simulink model "DYN_6DOF"  (R2018b)
settings: Solver=ode3  StartTime=0.0  StopTime=50  FixedStep=0.01  RelTol=1e-3
(part 2 of 18)

== matlab function DYN_6DOF/Dynamics ==
  data: the input; M output; C output; G output; thed input; m input; I input; len input; x input; y input; z input
function [M,C,G] = fcn(the, thed, m, I, len,x,y,z)
the1 = the(1); the2 = the(2); the3 = the(3);
the4 = the(4); the5 = the(5); the6 = the(6);
the1_dot = thed(1); the2_dot = thed(2); the3_dot = thed(3);
the4_dot = thed(4); the5_dot = thed(5); the6_dot = thed(6);

a1 = len(1);
a2 = len(2); a3 = len(3);
d4 = len(4); 
d7 = len(5)+len(6); d1 = len(7); 
g = 9.81;
m1 = m(1); 
m2 = m(2); 
m3 = m(3); 
m4 = m(4); 
m5 = m(5); 
m6 = m(6);

x1 = x(1); y1 = y(1); z1 = z(1);
x2 = x(2); y2 = y(2); z2 = z(2);
x3 = x(3); y3 = y(3); z3 = z(3);
x4 = x(4); y4 = y(4); z4 = z(4);
x5 = x(5); y5 = y(5); z5 = z(5);
x6 = x(6); y6 = y(6); z6 = z(6);

Ixx1 = I(1,1); Ixx2 = I(2,1); Ixx3 = I(3,1); Ixx4 = I(4,1); Ixx5 = I(5,1); Ixx6 = I(6,1);
Iyy1 = I(1,2); Iyy2 = I(2,2); Iyy3 = I(3,2); Iyy4 = I(4,2); Iyy5 = I(5,2); Iyy6 = I(6,2);
Izz1 = I(1,3); Izz2 = I(2,3); Izz3 = I(3,3); Izz4 = I(4,3); Izz5 = I(5,3); Izz6 = I(6,3);
IPx1 = I(1,4); IPx2 = I(2,4); IPx3 = I(3,4); IPx4 = I(4,4); IPx5 = I(5,4); IPx6 = I(6,4);
IPy1 = I(1,5); IPy2 = I(2,5); IPy3 = I(3,5); IPy4 = I(4,5); IPy5 = I(5,5); IPy6 = I(6,5);
IPz1 = I(1,6); IPz2 = I(2,6); IPz3 = I(3,6); IPz4 = I(4,6); IPz5 = I(5,6); IPz6 = I(6,6);

M = ...
[Ixx2 + Ixx5 + Iyy3 + Iyy6 + Izz1 + Izz4 + a1^2*m2 + a1^2*m3 + a1^2*m4 + a1^2*m5 + a1^2*m6 + a3^2*m4 + a3^2*m5 + a3^2*m6 + m1*x1^2 + m3*x3^2 + m4*x4^2 + m6*x6^2 + m1*y1^2 + m2*y2^2 + m4*y4^2 + m5*y5^2 + m2*z2^2 + m3*z3^2 + m5*z5^2 + m6*z6^2 - Ixx2*cos(the2)^2 + Ixx3*cos(the2)^2 + Ixx3*cos(the3)^2 - Ixx5*cos(the2)^2 - Ixx5*cos(the3)^2 + Ixx6*cos(the2)^2 + Ixx6*cos(the3)^2 - Ixx5*cos(the5)^2 + Ixx6*cos(the6)^2 + Iyy2*cos(the2)^2 - Iyy3*cos(the2)^2 - Iyy3*cos(the3)^2 + Iyy4*cos(the2)^2 + Iyy4*cos(the3)^2 - Iyy6*cos(the2)^2 - Iyy6*cos(the3)^2 + Iyy5*cos(the5)^2 - Iyy6*cos(the5)^2 - Iyy6*cos(the6)^2 - Izz4*cos(the2)^2 - Izz4*cos(the3)^2 + Izz5*cos(the2)^2 + Izz5*cos(the3)^2 + Izz6*cos(the5)^2 - IPx2*sin(2*the2) + IPx3*sin(2*the2) + IPx3*sin(2*the3) - IPx5*sin(2*the5) + IPx6*sin(2*the6) - 2*Ixx3*cos(the2)^2*cos(the3)^2 + Ixx4*cos(the2)^2*cos(the4)^2 + 2*Ixx5*cos(the2)^2*cos(the3)^2 + Ixx4*cos(the3)^2*cos(the4)^2 - 2*Ixx6*cos(the2)^2*cos(the3)^2 + Ixx5*cos(the2)^2*cos(the5)^2 - Ixx6*cos(the2)^2*cos(the4)^2 + Ixx5*cos(the3)^2*cos(the5)^2 - Ixx6*cos(the3)^2*cos(the4)^2 - 2*Ixx6*cos(the2)^2*cos(the6)^2 - 2*Ixx6*cos(the3)^2*cos(the6)^2 - Ixx6*cos(the5)^2*cos(the6)^2 + 2*Iyy3*cos(the2)^2*cos(the3)^2 - 2*Iyy4*cos(the2)^2*cos(the3)^2 - Iyy4*cos(the2)^2*cos(the4)^2 - Iyy4*cos(the3)^2*cos(the4)^2 + Iyy5*cos(the2)^2*cos(the4)^2 + 2*Iyy6*cos(the2)^2*cos(the3)^2 - Iyy5*cos(the2)^2*cos(the5)^2 + Iyy5*cos(the3)^2*cos(the4)^2 - Iyy5*cos(the3)^2*cos(the5)^2 + Iyy6*cos(the2)^2*cos(the5)^2 + 2*Iyy6*cos(the2)^2*cos(the6)^2 + Iyy6*cos(the3)^2*cos(the5)^2 + 2*Iyy6*cos(the3)^2*cos(the6)^2 + Iyy6*cos(the5)^2*cos(the6)^2 + 2*Izz4*cos(the2)^2*cos(the3)^2 - 2*Izz5*cos(the2)^2*cos(the3)^2 - Izz5*cos(the2)^2*cos(the4)^2 - Izz5*cos(the3)^2*cos(the4)^2 + Izz6*cos(the2)^2*cos(the4)^2 - Izz6*cos(the2)^2*cos(the5)^2 + Izz6*cos(the3)^2*cos(the4)^2 - Izz6*cos(the3)^2*cos(the5)^2 + a2^2*m3*cos(the2)^2 + a2^2*m4*cos(the2)^2 + a2^2*m5*cos(the2)^2 - a3^2*m4*cos(the2)^2 + a2^2*m6*cos(the2)^2 - a3^2*m4*cos(the3)^2 - a3^2*m5*cos(the2)^2 - a3^2*m5*cos(the3)^2 - a3^2*m6*cos(the2)^2 - a3^2*m6*cos(the3)^2 + d4^2*m4*cos(the2)^2 + d4^2*m4*cos(the3)^2 + d4^2*m5*cos(the2)^2 + d4^2*m5*cos(the3)^2 + d4^2*m6*cos(the2)^2 + d4^2*m6*cos(the3)^2 + m2*x2^2*cos(the2)^2 - m3*x3^2*cos(the2)^2 - m3*x3^2*cos(the3)^2 + m5*x5^2*cos(the2)^2 + m5*x5^2*cos(the3)^2 - m6*x6^2*cos(the2)^2 + m5*x5^2*cos(the5)^2 - m6*x6^2*cos(the3)^2 - m6*x6^2*cos(the6)^2 - m2*y2^2*cos(the2)^2 + m3*y3^2*cos(the2)^2 + m3*y3^2*cos(the3)^2 - m4*y4^2*cos(the2)^2 - m4*y4^2*cos(the3)^2 + m6*y6^2*cos(the2)^2 - m5*y5^2*cos(the5)^2 + m6*y6^2*cos(the3)^2 + m6*y6^2*cos(the5)^2 + m6*y6^2*cos(the6)^2 + m4*z4^2*cos(the2)^2 + m4*z4^2*cos(the3)^2 - m5*z5^2*cos(the2)^2 - m5*z5^2*cos(the3)^2 - m6*z6^2*cos(the5)^2 - m2*x2*y2*sin(2*the2) + m3*x3*y3*sin(2*the2) + m3*x3*y3*sin(2*the3) - m5*x5*y5*sin(2*the5) + m6*x6*y6*sin(2*the6) + 2*m3*x3^2*cos(the2)^2*cos(the3)^2 - m4*x4^2*cos(the2)^2*cos(the4)^2 - m4*x4^2*cos(the3)^2*cos(the4)^2 - 2*m5*x5^2*cos(the2)^2*cos(the3)^2 - m5*x5^2*cos(the2)^2*cos(the5)^2 + 2*m6*x6^2*cos(the2)^2*cos(the3)^2 - m5*x5^2*cos(the3)^2*cos(the5)^2 + m6*x6^2*cos(the2)^2*cos(the4)^2 + m6*x6^2*cos(the3)^2*cos(the4)^2 + 2*m6*x6^2*cos(the2)^2*cos(the6)^2 + 2*m6*x6^2*cos(the3)^2*cos(the6)^2 + m6*x6^2*cos(the5)^2*cos(the6)^2 - 2*m3*y3^2*cos(the2)^2*cos(the3)^2 + 2*m4*y4^2*cos(the2)^2*cos(the3)^2 + m4*y4^2*cos(the2)^2*cos(the4)^2 + m4*y4^2*cos(the3)^2*cos(the4)^2 - m5*y5^2*cos(the2)^2*cos(the4)^2 + m5*y5^2*cos(the2)^2*cos(the5)^2 - m5*y5^2*cos(the3)^2*cos(the4)^2 - 2*m6*y6^2*cos(the2)^2*cos(the3)^2 + m5*y5^2*cos(the3)^2*cos(the5)^2 - m6*y6^2*cos(the2)^2*cos(the5)^2 - 2*m6*y6^2*cos(the2)^2*cos(the6)^2 - m6*y6^2*cos(the3)^2*cos(the5)^2 - 2*m6*y6^2*cos(the3)^2*cos(the6)^2 - m6*y6^2*cos(the5)^2*cos(the6)^2 - 2*m4*z4^2*cos(the2)^2*cos(the3)^2 + 2*m5*z5^2*cos(the2)^2*cos(the3)^2 + m5*z5^2*cos(the2)^2*cos(the4)^2 + m5*z5^2*cos(the3)^2*cos(the4)^2 - m6*z6^2*cos(the2)^2*cos(the4)^2 + m6*z6^2*cos(the2)^2*cos(the5)^2 - m6*z6^2*cos(the3)^2*cos(the4)^2 + m6*z6^2*cos(the3)^2*cos(the5)^2 - 2*IPx5*cos(the2)*cos(the4)*sin(the2) - 2*IPx5*cos(the3)*cos(the4)*sin(the3) + 2*IPz4*cos(the2)*cos(the4)*sin(the2) + 2*IPz4*cos(the3)*cos(the4)*sin(the3) - 2*IPz6*cos(the5)*cos(the6)*sin(the5) - 2*Ixx4*cos(the2)^2*cos(the3)^2*cos(the4)^2 - 2*Ixx5*cos(the2)^2*cos(the3)^2*cos(the5)^2 + 2*Ixx6*cos(the2)^2*cos(the3)^2*cos(the4)^2 + Ixx5*cos(the2)^2*cos(the4)^2*cos(the5)^2 + Ixx5*cos(the3)^2*cos(the4)^2*cos(the5)^2 + 4*Ixx6*cos(the2)^2*cos(the3)^2*cos(the6)^2 + Ixx6*cos(the2)^2*cos(the4)^2*cos(the6)^2 + Ixx6*cos(the2)^2*cos(the5)^2*cos(the6)^2 + Ixx6*cos(the3)^2*cos(the4)^2*cos(the6)^2 + Ixx6*cos(the3)^2*cos(the5)^2*cos(the6)^2 + 2*Iyy4*cos(the2)^2*cos(the3)^2*cos(the4)^2 - 2*Iyy5*cos(the2)^2*cos(the3)^2*cos(the4)^2 + 2*Iyy5*cos(the2)^2*cos(the3)^2*cos(the5)^2 - Iyy5*cos(the2)^2*cos(the4)^2*cos(the5)^2 - 2*Iyy6*cos(the2)^2*cos(the3)^2*cos(the5)^2 - Iyy5*cos(the3)^2*cos(the4)^2*cos(the5)^2 - 4*Iyy6*cos(the2)^2*cos(the3)^2*cos(the6)^2 + Iyy6*cos(the2)^2*cos(the4)^2*cos(the5)^2 - Iyy6*cos(the2)^2*cos(the4)^2*cos(the6)^2 + Iyy6*cos(the3)^2*cos(the4)^2*cos(the5)^2 - Iyy6*cos(the2)^2*cos(the5)^2*cos(the6)^2 - Iyy6*cos(the3)^2*cos(the4)^2*cos(the6)^2 - Iyy6*cos(the3)^2*cos(the5)^2*cos(the6)^2 + 2*Izz5*cos(the2)^2*cos(the3)^2*cos(the4)^2 - 2*Izz6*cos(the2)^2*cos(the3)^2*cos(the4)^2 + 2*Izz6*cos(the2)^2*cos(the3)^2*cos(the5)^2 - Izz6*cos(the2)^2*cos(the4)^2*cos(the5)^2 - Izz6*cos(the3)^2*cos(the4)^2*cos(the5)^2 - 2*IPy4*cos(the2)*sin(the2)*sin(the4) - 2*IPy4*cos(the3)*sin(the3)*sin(the4) + 2*IPy6*cos(the5)*sin(the5)*sin(the6) + 2*a1*a2*m3*cos(the2) + 2*a1*a2*m4*cos(the2) + 2*a1*a2*m5*cos(the2) + 2*a1*a2*m6*cos(the2) + 2*a1*m2*x2*cos(the2) + 2*a3*m4*x4*cos(the4) - 2*a1*m2*y2*sin(the2) - 2*a3*m4*y4*sin(the4) + 2*a3*m5*z5*sin(the4) - 4*IPx3*cos(the2)*cos(the3)^2*sin(the2) - 4*IPx3*cos(the2)^2*cos(the3)*sin(the3) + 2*IPx4*cos(the2)^2*cos(the4)*sin(the4) + 2*IPx4*cos(the3)^2*cos(the4)*sin(the4) + 2*IPx5*cos(the2)^2*cos(the5)*sin(the5) + 2*IPx5*cos(the3)^2*cos(the5)*sin(the5) - 4*IPx6*cos(the2)^2*cos(the6)*sin(the6) - 4*IPx6*cos(the3)^2*cos(the6)*sin(the6) - 2*IPx6*cos(the5)^2*cos(the6)*sin(the6) + a3*d4*m4*sin(2*the2) + a3*d4*m4*sin(2*the3) + a3*d4*m5*sin(2*the2) + a3*d4*m5*sin(2*the3) + a3*d4*m6*sin(2*the2) + a3*d4*m6*sin(2*the3) + 2*d4*m4*z4*cos(the2)^2 + 2*d4*m4*z4*cos(the3)^2 + a3*m4*z4*sin(2*the2) + a3*m4*z4*sin(2*the3) + 2*a3^2*m4*cos(the2)^2*cos(the3)^2 + 2*a3^2*m5*cos(the2)^2*cos(the3)^2 + 2*a3^2*m6*cos(the2)^2*cos(the3)^2 - 2*d4^2*m4*cos(the2)^2*cos(the3)^2 - 2*d4^2*m5*cos(the2)^2*cos(the3)^2 - 2*d4^2*m6*cos(the2)^2*cos(the3)^2 - 2*IPz6*cos(the2)*cos(the4)*cos(the6)*sin(the2) - 2*IPz6*cos(the3)*cos(the4)*cos(the6)*sin(the3) - 4*d4*m4*z4*cos(the2)^2*cos(the3)^2 + 2*IPy5*cos(the2)*cos(the5)*sin(the2)*sin(the4) + 2*IPy5*cos(the3)*cos(the5)*sin(the3)*sin(the4) + 2*IPy6*cos(the2)*cos(the4)*sin(the2)*sin(the6) + 2*IPy6*cos(the3)*cos(the4)*sin(the3)*sin(the6) + 2*Ixx3*cos(the2)*cos(the3)*sin(the2)*sin(the3) - 2*Ixx5*cos(the2)*cos(the3)*sin(the2)*sin(the3) + 2*Ixx6*cos(the2)*cos(the3)*sin(the2)*sin(the3) - 2*Iyy3*cos(the2)*cos(the3)*sin(the2)*sin(the3) + 2*Iyy4*cos(the2)*cos(the3)*sin(the2)*sin(the3) - 2*Iyy6*cos(the2)*cos(the3)*sin(the2)*sin(the3) - 2*Izz4*cos(the2)*cos(the3)*sin(the2)*sin(the3) + 2*Izz5*cos(the2)*cos(the3)*sin(the2)*sin(the3) + 2*IPx6*cos(the2)*sin(the2)*sin(the4)*sin(the5) + 2*IPx6*cos(the3)*sin(the3)*sin(the4)*sin(the5) + 2*IPz5*cos(the2)*sin(the2)*sin(the4)*sin(the5) + 2*IPz5*cos(the3)*sin(the3)*sin(the4)*sin(the5) + 2*a1*a3*m4*cos(the2)*cos(the3) + 2*a1*a3*m5*cos(the2)*cos(the3) + 2*a1*a3*m6*cos(the2)*cos(the3) + 2*m4*x4^2*cos(the2)^2*cos(the3)^2*cos(the4)^2 + 2*m5*x5^2*cos(the2)^2*cos(the3)^2*cos(the5)^2 - m5*x5^2*cos(the2)^2*cos(the4)^2*cos(the5)^2 - 2*m6*x6^2*cos(the2)^2*cos(the3)^2*cos(the4)^2 - m5*x5^2*cos(the3)^2*cos(the4)^2*cos(the5)^2 - 4*m6*x6^2*cos(the2)^2*cos(the3)^2*cos(the6)^2 - m6*x6^2*cos(the2)^2*cos(the4)^2*cos(the6)^2 - m6*x6^2*cos(the2)^2*cos(the5)^2*cos(the6)^2 - m6*x6^2*cos(the3)^2*cos(the4)^2*cos(the6)^2 - m6*x6^2*cos(the3)^2*cos(the5)^2*cos(the6)^2 - 2*m4*y4^2*cos(the2)^2*cos(the3)^2*cos(the4)^2 + 2*m5*y5^2*cos(the2)^2*cos(the3)^2*cos(the4)^2 - 2*m5*y5^2*cos(the2)^2*cos(the3)^2*cos(the5)^2 + m5*y5^2*cos(the2)^2*cos(the4)^2*cos(the5)^2 + m5*y5^2*cos(the3)^2*cos(the4)^2*cos(the5)^2 + 2*m6*y6^2*cos(the2)^2*cos(the3)^2*cos(the5)^2 + 4*m6*y6^2*cos(the2)^2*cos(the3)^2*cos(the6)^2 - m6*y6^2*cos(the2)^2*cos(the4)^2*cos(the5)^2 + m6*y6^2*cos(the2)^2*cos(the4)^2*cos(the6)^2 - m6*y6^2*cos(the3)^2*cos(the4)^2*cos(the5)^2 + m6*y6^2*cos(the2)^2*cos(the5)^2*cos(the6)^2 + m6*y6^2*cos(the3)^2*cos(the4)^2*cos(the6)^2 + m6*y6^2*cos(the3)^2*cos(the5)^2*cos(the6)^2 - 2*m5*z5^2*cos(the2)^2*cos(the3)^2*cos(the4)^2 + 2*m6*z6^2*cos(the2)^2*cos(the3)^2*cos(the4)^2 - 2*m6*z6^2*cos(the2)^2*cos(the3)^2*cos(the5)^2 + m6*z6^2*cos(the2)^2*cos(the4)^2*cos(the5)^2 + m6*z6^2*cos(the3)^2*cos(the4)^2*cos(the5)^2 - 2*a1*d4*m4*cos(the2)*sin(the3) - 2*a1*d4*m4*cos(the3)*sin(the2) - 2*a1*d4*m5*cos(the2)*sin(the3) - 2*a1*d4*m5*cos(the3)*sin(the2) - 2*a1*d4*m6*cos(the2)*sin(the3) - 2*a1*d4*m6*cos(the3)*sin(the2) + 2*a1*m3*x3*cos(the2)*cos(the3) + 2*a3*m5*x5*cos(the4)*cos(the5) - 2*a1*a3*m4*sin(the2)*sin(the3) - 2*a1*a3*m5*sin(the2)*sin(the3) - 2*a1*a3*m6*sin(the2)*sin(the3) - 2*a1*m3*y3*cos(the2)*sin(the3) - 2*a1*m3*y3*cos(the3)*sin(the2) - 2*a3*m5*y5*cos(the4)*sin(the5) - 2*a3*m6*y6*cos(the6)*sin(the4) - 2*a1*m4*z4*cos(the2)*sin(the3) - 2*a1*m4*z4*cos(the3)*sin(the2) - 2*a3*m6*z6*cos(the4)*sin(the5) - 2*a1*m3*x3*sin(the2)*sin(the3) - 2*a3*m6*x6*sin(the4)*sin(the6) + 4*IPx5*cos(the2)*cos(the3)^2*cos(the4)*sin(the2) + 4*IPx5*cos(the2)^2*cos(the3)*cos(the4)*sin(the3) + 4*IPx5*cos(the2)*cos(the4)*cos(the5)^2*sin(the2) + 4*IPx5*cos(the3)*cos(the4)*cos(the5)^2*sin(the3) - 2*IPx6*cos(the2)^2*cos(the4)*cos(the5)*sin(the4) - 2*IPx6*cos(the3)^2*cos(the4)*cos(the5)*sin(the4) - 4*IPz4*cos(the2)*cos(the3)^2*cos(the4)*sin(the2) - 4*IPz4*cos(the2)^2*cos(the3)*cos(the4)*sin(the3) - 2*IPz5*cos(the2)^2*cos(the4)*cos(the5)*sin(the4) - 2*IPz5*cos(the3)^2*cos(the4)*cos(the5)*sin(the4) + 2*IPz6*cos(the2)^2*cos(the5)*cos(the6)*sin(the5) + 2*IPz6*cos(the3)^2*cos(the5)*cos(the6)*sin(the5) - 2*Ixx5*cos(the2)^2*cos(the3)^2*cos(the4)^2*cos(the5)^2 - 2*Ixx6*cos(the2)^2*cos(the3)^2*cos(the4)^2*cos(the6)^2 - 2*Ixx6*cos(the2)^2*cos(the3)^2*cos(the5)^2*cos(the6)^2 + Ixx6*cos(the2)^2*cos(the4)^2*cos(the5)^2*cos(the6)^2 + Ixx6*cos(the3)^2*cos(the4)^2*cos(the5)^2*cos(the6)^2 + 2*Iyy5*cos(the2)^2*cos(the3)^2*cos(the4)^2*cos(the5)^2 - 2*Iyy6*cos(the2)^2*cos(the3)^2*cos(the4)^2*cos(the5)^2 + 2*Iyy6*cos(the2)^2*cos(the3)^2*cos(the4)^2*cos(the6)^2 + 2*Iyy6*cos(the2)^2*cos(the3)^2*cos(the5)^2*cos(the6)^2 - Iyy6*cos(the2)^2*cos(the4)^2*cos(the5)^2*cos(the6)^2 - Iyy6*cos(the3)^2*cos(the4)^2*cos(the5)^2*cos(the6)^2 + 2*Izz6*cos(the2)^2*cos(the3)^2*cos(the4)^2*cos(the5)^2 + 4*IPy4*cos(the2)*cos(the3)^2*sin(the2)*sin(the4) + 4*IPy4*cos(the2)^2*cos(the3)*sin(the3)*sin(the4) + 2*IPy5*cos(the2)^2*cos(the4)*sin(the4)*sin(the5) + 2*IPy5*cos(the3)^2*cos(the4)*sin(the4)*sin(the5) - 2*IPy6*cos(the2)^2*cos(the5)*sin(the5)*sin(the6) - 2*IPy6*cos(the3)^2*cos(the5)*sin(the5)*sin(the6) + 2*a2*a3*m4*cos(the2)^2*cos(the3) + 2*a2*a3*m5*cos(the2)^2*cos(the3) + 2*a2*a3*m6*cos(the2)^2*cos(the3) - 2*a2*d4*m4*cos(the2)^2*sin(the3) - 2*a2*d4*m5*cos(the2)^2*sin(the3) - 2*a2*d4*m6*cos(the2)^2*sin(the3) + 2*a2*m3*x3*cos(the2)^2*cos(the3) - 2*a3*m4*x4*cos(the2)^2*cos(the4) - 2*a3*m4*x4*cos(the3)^2*cos(the4) + 2*d4*m5*y5*cos(the2)^2*cos(the5) + 2*d4*m5*y5*cos(the3)^2*cos(the5) + 2*d4*m6*z6*cos(the2)^2*cos(the5) + 2*d4*m6*z6*cos(the3)^2*cos(the5) - 2*a2*m3*y3*cos(the2)^2*sin(the3) + 2*a3*m4*y4*cos(the2)^2*sin(the4) + 2*a3*m4*y4*cos(the3)^2*sin(the4) - 2*a2*m4*z4*cos(the2)^2*sin(the3) - 2*a3*m5*z5*cos(the2)^2*sin(the4) - 2*a3*m5*z5*cos(the3)^2*sin(the4) + 2*d4*m5*x5*cos(the2)^2*sin(the5) + 2*d4*m5*x5*cos(the3)^2*sin(the5) - 4*IPx4*cos(the2)^2*cos(the3)^2*cos(the4)*sin(the4) - 4*IPx5*cos(the2)^2*cos(the3)^2*cos(the5)*sin(the5) + 2*IPx5*cos(the2)^2*cos(the4)^2*cos(the5)*sin(the5) + 2*IPx5*cos(the3)^2*cos(the4)^2*cos(the5)*sin(the5) + 8*IPx6*cos(the2)^2*cos(the3)^2*cos(the6)*sin(the6) + 2*IPx6*cos(the2)^2*cos(the4)^2*cos(the6)*sin(the6) + 2*IPx6*cos(the2)^2*cos(the5)^2*cos(the6)*sin(the6) + 2*IPx6*cos(the3)^2*cos(the4)^2*cos(the6)*sin(the6) + 2*IPx6*cos(the3)^2*cos(the5)^2*cos(the6)*sin(the6) - 2*Ixx5*cos(the2)*cos(the4)*cos(the5)*sin(the2)*sin(the5) - 2*Ixx5*cos(the3)*cos(the4)*cos(the5)*sin(the3)*sin(the5) + 2*Iyy5*cos(the2)*cos(the4)*cos(the5)*sin(the2)*sin(the5) - 2*Iyy6*cos(the2)*cos(the4)*cos(the5)*sin(the2)*sin(the5) + 2*Iyy5*cos(the3)*cos(the4)*cos(the5)*sin(the3)*sin(the5) - 2*Iyy6*cos(the3)*cos(the4)*cos(the5)*sin(the3)*sin(the5) + 2*Izz6*cos(the2)*cos(the4)*cos(the5)*sin(the2)*sin(the5) + 2*Izz6*cos(the3)*cos(the4)*cos(the5)*sin(the3)*sin(the5) - 2*a3^2*m4*cos(the2)*cos(the3)*sin(the2)*sin(the3) - 2*a3^2*m5*cos(the2)*cos(the3)*sin(the2)*sin(the3) - 2*a3^2*m6*cos(the2)*cos(the3)*sin(the2)*sin(the3) - 4*IPx5*cos(the2)^2*cos(the3)^2*cos(the4)^2*cos(the5)*sin(the5) - 4*IPx6*cos(the2)^2*cos(the3)^2*cos(the4)^2*cos(the6)*sin(the6) - 4*IPx6*cos(the2)^2*cos(the3)^2*cos(the5)^2*cos(the6)*sin(the6) + 2*IPx6*cos(the2)^2*cos(the4)^2*cos(the5)^2*cos(the6)*sin(the6) + 2*IPx6*cos(the3)^2*cos(the4)^2*cos(the5)^2*cos(the6)*sin(the6) + 2*d4^2*m4*cos(the2)*cos(the3)*sin(the2)*sin(the3) + 2*d4^2*m5*cos(the2)*cos(the3)*sin(the2)*sin(the3) + 2*d4^2*m6*cos(the2)*cos(the3)*sin(the2)*sin(the3) - 2*IPz6*cos(the2)*cos(the5)*sin(the2)*sin(the4)*sin(the6) - 2*IPz6*cos(the3)*cos(the5)*sin(the3)*sin(the4)*sin(the6) - 2*m3*x3^2*cos(the2)*cos(the3)*sin(the2)*sin(the3) + 2*m5*x5^2*cos(the2)*cos(the3)*sin(the2)*sin(the3) - 2*m6*x6^2*cos(the2)*cos(the3)*sin(the2)*sin(the3) + 2*m3*y3^2*cos(the2)*cos(the3)*sin(the2)*sin(the3) - 2*m4*y4^2*cos(the2)*cos(the3)*sin(the2)*sin(the3) + 2*m6*y6^2*cos(the2)*cos(the3)*sin(the2)*sin(the3) + 2*m4*z4^2*cos(the2)*cos(the3)*sin(the2)*sin(the3) - 2*m5*z5^2*cos(the2)*cos(the3)*sin(the2)*sin(the3) - 2*a2*d4*m4*cos(the2)*cos(the3)*sin(the2) - 2*a2*d4*m5*cos(the2)*cos(the3)*sin(the2) - 2*a2*d4*m6*cos(the2)*cos(the3)*sin(the2) + 2*a1*m4*x4*cos(the2)*cos(the3)*cos(the4) + 2*a3*m6*x6*cos(the4)*cos(the5)*cos(the6) - 2*a2*a3*m4*cos(the2)*sin(the2)*sin(the3) - 2*a2*a3*m5*cos(the2)*sin(the2)*sin(the3) - 2*a2*a3*m6*cos(the2)*sin(the2)*sin(the3) - 2*a2*m3*y3*cos(the2)*cos(the3)*sin(the2) - 2*a1*m4*y4*cos(the2)*cos(the3)*sin(the4) - 2*a1*m5*y5*cos(the2)*cos(the5)*sin(the3) - 2*a1*m5*y5*cos(the3)*cos(the5)*sin(the2) + 2*a3*m5*y5*cos(the2)*cos(the5)*sin(the2) + 2*a3*m5*y5*cos(the3)*cos(the5)*sin(the3) - 2*a3*m6*y6*cos(the4)*cos(the5)*sin(the6) - 2*a2*m4*z4*cos(the2)*cos(the3)*sin(the2) + 2*a1*m5*z5*cos(the2)*cos(the3)*sin(the4) - 2*a1*m6*z6*cos(the2)*cos(the5)*sin(the3) - 2*a1*m6*z6*cos(the3)*cos(the5)*sin(the2) + 2*a3*m6*z6*cos(the2)*cos(the5)*sin(the2) + 2*a3*m6*z6*cos(the3)*cos(the5)*sin(the3) + 2*d4*m4*x4*cos(the2)*cos(the4)*sin(the2) + 2*d4*m4*x4*cos(the3)*cos(the4)*sin(the3) - 2*a2*m3*x3*cos(the2)*sin(the2)*sin(the3) - 2*a1*m4*x4*cos(the4)*sin(the2)*sin(the3) - 2*a1*m5*x5*cos(the2)*sin(the3)*sin(the5) - 2*a1*m5*x5*cos(the3)*sin(the2)*sin(the5) + 2*a3*m5*x5*cos(the2)*sin(the2)*sin(the5) + 2*a3*m5*x5*cos(the3)*sin(the3)*sin(the5) + 4*IPz6*cos(the2)*cos(the3)^2*cos(the4)*cos(the6)*sin(the2) + 4*IPz6*cos(the2)^2*cos(the3)*cos(the4)*cos(the6)*sin(the3) + 4*IPz6*cos(the2)*cos(the4)*cos(the5)^2*cos(the6)*sin(the2) + 4*IPz6*cos(the3)*cos(the4)*cos(the5)^2*cos(the6)*sin(the3) - 2*d4*m4*y4*cos(the2)*sin(the2)*sin(the4) - 2*d4*m4*y4*cos(the3)*sin(the3)*sin(the4) + 2*d4*m5*z5*cos(the2)*sin(the2)*sin(the4) + 2*d4*m5*z5*cos(the3)*sin(the3)*sin(the4) - 2*m5*x5*y5*cos(the2)*cos(the4)*sin(the2) - 2*m5*x5*y5*cos(the3)*cos(the4)*sin(the3) + 2*m4*x4*z4*cos(the2)*cos(the4)*sin(the2) + 2*m4*x4*z4*cos(the3)*cos(the4)*sin(the3) - 2*m6*x6*z6*cos(the5)*cos(the6)*sin(the5) + 2*a1*m4*y4*sin(the2)*sin(the3)*sin(the4) - 2*a1*m5*z5*sin(the2)*sin(the3)*sin(the4) - 4*IPy5*cos(the2)*cos(the3)^2*cos(the5)*sin(the2)*sin(the4) - 4*IPy5*cos(the2)^2*cos(the3)*cos(the5)*sin(the3)*sin(the4) - 4*IPy6*cos(the2)*cos(the3)^2*cos(the4)*sin(the2)*sin(the6) - 4*IPy6*cos(the2)^2*cos(the3)*cos(the4)*sin(the3)*sin(the6) - 4*IPy6*cos(the2)*cos(the4)*cos(the5)^2*sin(the2)*sin(the6) - 4*IPy6*cos(the3)*cos(the4)*cos(the5)^2*sin(the3)*sin(the6) - 2*IPy6*cos(the2)^2*cos(the4)*cos(the6)*sin(the4)*sin(the5) - 2*IPy6*cos(the3)^2*cos(the4)*cos(the6)*sin(the4)*sin(the5) + 2*Ixx4*cos(the2)*cos(the3)*cos(the4)^2*sin(the2)*sin(the3) + 2*Ixx5*cos(the2)*cos(the3)*cos(the5)^2*sin(the2)*sin(the3) - 2*Ixx6*cos(the2)*cos(the3)*cos(the4)^2*sin(the2)*sin(the3) - 4*Ixx6*cos(the2)*cos(the3)*cos(the6)^2*sin(the2)*sin(the3) - 2*Iyy4*cos(the2)*cos(the3)*cos(the4)^2*sin(the2)*sin(the3) + 2*Iyy5*cos(the2)*cos(the3)*cos(the4)^2*sin(the2)*sin(the3) - 2*Iyy5*cos(the2)*cos(the3)*cos(the5)^2*sin(the2)*sin(the3) + 2*Iyy6*cos(the2)*cos(the3)*cos(the5)^2*sin(the2)*sin(the3) + 4*Iyy6*cos(the2)*cos(the3)*cos(the6)^2*sin(the2)*sin(the3) - 2*Izz5*cos(the2)*cos(the3)*cos(the4)^2*sin(the2)*sin(the3) + 2*Izz6*cos(the2)*cos(the3)*cos(the4)^2*sin(the2)*sin(the3) - 2*Izz6*cos(the2)*cos(the3)*cos(the5)^2*sin(the2)*sin(the3) - 2*m4*y4*z4*cos(the2)*sin(the2)*sin(the4) - 2*m4*y4*z4*cos(the3)*sin(the3)*sin(the4) + 2*m6*y6*z6*cos(the5)*sin(the5)*sin(the6) - 4*IPx6*cos(the2)*cos(the3)^2*sin(the2)*sin(the4)*sin(the5) - 4*IPx6*cos(the2)^2*cos(the3)*sin(the3)*sin(the4)*sin(the5) - 4*IPx6*cos(the2)*cos(the6)^2*sin(the2)*sin(the4)*sin(the5) - 4*IPx6*cos(the3)*cos(the6)^2*sin(the3)*sin(the4)*sin(the5) - 4*IPz5*cos(the2)*cos(the3)^2*sin(the2)*sin(the4)*sin(the5) - 4*IPz5*cos(the2)^2*cos(the3)*sin(the3)*sin(the4)*sin(the5) - 2*IPz6*cos(the2)^2*cos(the4)*sin(the4)*sin(the5)*sin(the6) - 2*IPz6*cos(the3)^2*cos(the4)*sin(the4)*sin(the5)*sin(the6) + 2*m5*x5^2*cos(the2)^2*cos(the3)^2*cos(the4)^2*cos(the5)^2 + 2*m6*x6^2*cos(the2)^2*cos(the3)^2*cos(the4)^2*cos(the6)^2 + 2*m6*x6^2*cos(the2)^2*cos(the3)^2*cos(the5)^2*cos(the6)^2 - m6*x6^2*cos(the2)^2*cos(the4)^2*cos(the5)^2*cos(the6)^2 - m6*x6^2*cos(the3)^2*cos(the4)^2*cos(the5)^2*cos(the6)^2 - 2*m5*y5^2*cos(the2)^2*cos(the3)^2*cos(the4)^2*cos(the5)^2 + 2*m6*y6^2*cos(the2)^2*cos(the3)^2*cos(the4)^2*cos(the5)^2 - 2*m6*y6^2*cos(the2)^2*cos(the3)^2*cos(the4)^2*cos(the6)^2 - 2*m6*y6^2*cos(the2)^2*cos(the3)^2*cos(the5)^2*cos(the6)^2 + m6*y6^2*cos(the2)^2*cos(the4)^2*cos(the5)^2*cos(the6)^2 + m6*y6^2*cos(the3)^2*cos(the4)^2*cos(the5)^2*cos(the6)^2 - 2*m6*z6^2*cos(the2)^2*cos(the3)^2*cos(the4)^2*cos(the5)^2 - 4*a3*d4*m4*cos(the2)*cos(the3)^2*sin(the2) - 4*a3*d4*m4*cos(the2)^2*cos(the3)*sin(the3) - 4*a3*d4*m5*cos(the2)*cos(the3)^2*sin(the2) - 4*a3*d4*m5*cos(the2)^2*cos(the3)*sin(the3) - 4*a3*d4*m6*cos(the2)*cos(the3)^2*sin(the2) - 4*a3*d4*m6*cos(the2)^2*cos(the3)*sin(the3) + 2*a2*m4*x4*cos(the2)^2*cos(the3)*cos(the4) - 2*a3*m5*x5*cos(the2)^2*cos(the4)*cos(the5) - 2*a3*m5*x5*cos(the3)^2*cos(the4)*cos(the5) - 2*a2*m4*y4*cos(the2)^2*cos(the3)*sin(the4) - 2*a2*m5*y5*cos(the2)^2*cos(the5)*sin(the3) + 2*a3*m5*y5*cos(the2)^2*cos(the4)*sin(the5) + 2*a3*m5*y5*cos(the3)^2*cos(the4)*sin(the5) + 2*a3*m6*y6*cos(the2)^2*cos(the6)*sin(the4) + 2*a3*m6*y6*cos(the3)^2*cos(the6)*sin(the4) - 4*a3*m4*z4*cos(the2)*cos(the3)^2*sin(the2) - 4*a3*m4*z4*cos(the2)^2*cos(the3)*sin(the3) + 2*a2*m5*z5*cos(the2)^2*cos(the3)*sin(the4) - 2*a2*m6*z6*cos(the2)^2*cos(the5)*sin(the3) + 2*a3*m6*z6*cos(the2)^2*cos(the4)*sin(the5) + 2*a3*m6*z6*cos(the3)^2*cos(the4)*sin(the5) + 2*d4*m6*x6*cos(the2)^2*cos(the6)*sin(the5) + 2*d4*m6*x6*cos(the3)^2*cos(the6)*sin(the5) - 2*a2*m5*x5*cos(the2)^2*sin(the3)*sin(the5) + 2*a3*m6*x6*cos(the2)^2*sin(the4)*sin(the6) + 2*a3*m6*x6*cos(the3)^2*sin(the4)*sin(the6) - 8*IPx5*cos(the2)*cos(the3)^2*cos(the4)*cos(the5)^2*sin(the2) - 8*IPx5*cos(the2)^2*cos(the3)*cos(the4)*cos(the5)^2*sin(the3) + 4*IPx6*cos(the2)^2*cos(the3)^2*cos(the4)*cos(the5)*sin(the4) + 4*IPx6*cos(the2)^2*cos(the4)*cos(the5)*cos(the6)^2*sin(the4) + 4*IPx6*cos(the3)^2*cos(the4)*cos(the5)*cos(the6)^2*sin(the4) + 4*IPz5*cos(the2)^2*cos(the3)^2*cos(the4)*cos(the5)*sin(the4) - 4*IPz6*cos(the2)^2*cos(the3)^2*cos(the5)*cos(the6)*sin(the5) + 2*IPz6*cos(the2)^2*cos(the4)^2*cos(the5)*cos(the6)*sin(the5) + 2*IPz6*cos(the3)^2*cos(the4)^2*cos(the5)*cos(the6)*sin(the5) - 2*d4*m6*y6*cos(the2)^2*sin(the5)*sin(the6) - 2*d4*m6*y6*cos(the3)^2*sin(the5)*sin(the6) - 4*m3*x3*y3*cos(the2)*cos(the3)^2*sin(the2) - 4*m3*x3*y3*cos(the2)^2*cos(the3)*sin(the3) + 2*m4*x4*y4*cos(the2)^2*cos(the4)*sin(the4) + 2*m4*x4*y4*cos(the3)^2*cos(the4)*sin(the4) + 2*m5*x5*y5*cos(the2)^2*cos(the5)*sin(the5) + 2*m5*x5*y5*cos(the3)^2*cos(the5)*sin(the5) - 4*m6*x6*y6*cos(the2)^2*cos(the6)*sin(the6) - 4*m6*x6*y6*cos(the3)^2*cos(the6)*sin(the6) - 2*m6*x6*y6*cos(the5)^2*cos(the6)*sin(the6) - 2*Ixx6*cos(the2)^2*cos(the3)^2*cos(the4)^2*cos(the5)^2*cos(the6)^2 + 2*Iyy6*cos(the2)^2*cos(the3)^2*cos(the4)^2*cos(the5)^2*cos(the6)^2 - 4*IPy5*cos(the2)^2*cos(the3)^2*cos(the4)*sin(the4)*sin(the5) + 4*IPy6*cos(the2)^2*cos(the3)^2*cos(the5)*sin(the5)*sin(the6) - 2*IPy6*cos(the2)^2*cos(the4)^2*cos(the5)*sin(the5)*sin(the6) - 2*IPy6*cos(the3)^2*cos(the4)^2*cos(the5)*sin(the5)*sin(the6) + 4*a3*m4*x4*cos(the2)^2*cos(the3)^2*cos(the4) - 4*d4*m5*y5*cos(the2)^2*cos(the3)^2*cos(the5) - 4*d4*m6*z6*cos(the2)^2*cos(the3)^2*cos(the5) - 4*a3*m4*y4*cos(the2)^2*cos(the3)^2*sin(the4) + 4*a3*m5*z5*cos(the2)^2*cos(the3)^2*sin(the4) - 4*d4*m5*x5*cos(the2)^2*cos(the3)^2*sin(the5) - 2*IPy6*cos(the2)*cos(the5)*cos(the6)*sin(the2)*sin(the4) - 2*IPy6*cos(the3)*cos(the5)*cos(the6)*sin(the3)*sin(the4) + 2*a1*m5*x5*cos(the2)*cos(the3)*cos(the4)*cos(the5) - 2*a2*m5*y5*cos(the2)*cos(the3)*cos(the5)*sin(the2) - 2*a1*m5*y5*cos(the2)*cos(the3)*cos(the4)*sin(the5) - 2*a1*m6*y6*cos(the2)*cos(the3)*cos(the6)*sin(the4) - 2*a2*m6*z6*cos(the2)*cos(the3)*cos(the5)*sin(the2) - 2*a1*m6*z6*cos(the2)*cos(the3)*cos(the4)*sin(the5) + 2*d4*m5*x5*cos(the2)*cos(the4)*cos(the5)*sin(the2) + 2*d4*m5*x5*cos(the3)*cos(the4)*cos(the5)*sin(the3) - 2*a2*m4*x4*cos(the2)*cos(the4)*sin(the2)*sin(the3) - 2*a2*m5*x5*cos(the2)*cos(the3)*sin(the2)*sin(the5) - 2*a1*m5*x5*cos(the4)*cos(the5)*sin(the2)*sin(the3) - 2*a1*m6*x6*cos(the2)*cos(the3)*sin(the4)*sin(the6) - 2*a1*m6*x6*cos(the2)*cos(the6)*sin(the3)*sin(the5) - 2*a1*m6*x6*cos(the3)*cos(the6)*sin(the2)*sin(the5) + 2*a3*m6*x6*cos(the2)*cos(the6)*sin(the2)*sin(the5) + 2*a3*m6*x6*cos(the3)*cos(the6)*sin(the3)*sin(the5) - 2*d4*m5*y5*cos(the2)*cos(the4)*sin(the2)*sin(the5) - 2*d4*m5*y5*cos(the3)*cos(the4)*sin(the3)*sin(the5) - 2*d4*m6*y6*cos(the2)*cos(the6)*sin(the2)*sin(the4) - 2*d4*m6*y6*cos(the3)*cos(the6)*sin(the3)*sin(the4) + 4*d4*m4*z4*cos(the2)*cos(the3)*sin(the2)*sin(the3) - 2*d4*m6*z6*cos(the2)*cos(the4)*sin(the2)*sin(the5) - 2*d4*m6*z6*cos(the3)*cos(the4)*sin(the3)*sin(the5) - 2*m6*x6*z6*cos(the2)*cos(the4)*cos(the6)*sin(the2) - 2*m6*x6*z6*cos(the3)*cos(the4)*cos(the6)*sin(the3) + 2*a2*m4*y4*cos(the2)*sin(the2)*sin(the3)*sin(the4) + 2*a1*m5*y5*cos(the4)*sin(the2)*sin(the3)*sin(the5) + 2*a1*m6*y6*cos(the6)*sin(the2)*sin(the3)*sin(the4) + 2*a1*m6*y6*cos(the2)*sin(the3)*sin(the5)*sin(the6) + 2*a1*m6*y6*cos(the3)*sin(the2)*sin(the5)*sin(the6) - 2*a3*m6*y6*cos(the2)*sin(the2)*sin(the5)*sin(the6) - 2*a3*m6*y6*cos(the3)*sin(the3)*sin(the5)*sin(the6) - 2*a2*m5*z5*cos(the2)*sin(the2)*sin(the3)*sin(the4) + 2*a1*m6*z6*cos(the4)*sin(the2)*sin(the3)*sin(the5) + 4*IPy6*cos(the2)*cos(the3)^2*cos(the5)*cos(the6)*sin(the2)*sin(the4) + 4*IPy6*cos(the2)^2*cos(the3)*cos(the5)*cos(the6)*sin(the3)*sin(the4) + 4*Ixx5*cos(the2)*cos(the3)^2*cos(the4)*cos(the5)*sin(the2)*sin(the5) + 4*Ixx5*cos(the2)^2*cos(the3)*cos(the4)*cos(the5)*sin(the3)*sin(the5) - 2*Ixx6*cos(the2)*cos(the4)*cos(the5)*cos(the6)^2*sin(the2)*sin(the5) - 2*Ixx6*cos(the3)*cos(the4)*cos(the5)*cos(the6)^2*sin(the3)*sin(the5) - 2*Ixx6*cos(the2)^2*cos(the4)*cos(the5)*cos(the6)*sin(the4)*sin(the6) - 2*Ixx6*cos(the3)^2*cos(the4)*cos(the5)*cos(the6)*sin(the4)*sin(the6) - 4*Iyy5*cos(the2)*cos(the3)^2*cos(the4)*cos(the5)*sin(the2)*sin(the5) - 4*Iyy5*cos(the2)^2*cos(the3)*cos(the4)*cos(the5)*sin(the3)*sin(the5) + 4*Iyy6*cos(the2)*cos(the3)^2*cos(the4)*cos(the5)*sin(the2)*sin(the5) + 4*Iyy6*cos(the2)^2*cos(the3)*cos(the4)*cos(the5)*sin(the3)*sin(the5) + 2*Iyy6*cos(the2)*cos(the4)*cos(the5)*cos(the6)^2*sin(the2)*sin(the5) + 2*Iyy6*cos(the3)*cos(the4)*cos(the5)*cos(the6)^2*sin(the3)*sin(the5) + 2*Iyy6*cos(the2)^2*cos(the4)*cos(the5)*cos(the6)*sin(the4)*sin(the6) + 2*Iyy6*cos(the3)^2*cos(the4)*cos(the5)*cos(the6)*sin(the4)*sin(the6) - 4*Izz6*cos(the2)*cos(the3)^2*cos(the4)*cos(the5)*sin(the2)*sin(the5) - 4*Izz6*cos(the2)^2*cos(the3)*cos(the4)*cos(the5)*sin(the3)*sin(the5) - 2*d4*m6*x6*cos(the2)*sin(the2)*sin(the4)*sin(the6) - 2*d4*m6*x6*cos(the3)*sin(the3)*sin(the4)*sin(the6) + 2*m5*y5*z5*cos(the2)*cos(the5)*sin(the2)*sin(the4) + 2*m5*y5*z5*cos(the3)*cos(the5)*sin(the3)*sin(the4) + 2*m6*y6*z6*cos(the2)*cos(the4)*sin(the2)*sin(the6) + 2*m6*y6*z6*cos(the3)*cos(the4)*sin(the3)*sin(the6) + 2*a1*m6*x6*sin(the2)*sin(the3)*sin(the4)*sin(the6) - 4*IPx6*cos(the2)^2*cos(the3)^2*cos(the4)^2*cos(the5)^2*cos(the6)*sin(the6) + 4*IPz6*cos(the2)*cos(the3)^2*cos(the5)*sin(the2)*sin(the4)*sin(the6) + 4*IPz6*cos(the2)^2*cos(the3)*cos(the5)*sin(the3)*sin(the4)*sin(the6) + 2*m6*x6*y6*cos(the2)*sin(the2)*sin(the4)*sin(the5) + 2*m6*x6*y6*cos(the3)*sin(the3)*sin(the4)*sin(the5) + 2*m5*x5*z5*cos(the2)*sin(the2)*sin(the4)*sin(the5) + 2*m5*x5*z5*cos(the3)*sin(the3)*sin(the4)*sin(the5) - 2*m4*x4^2*cos(the2)*cos(the3)*cos(the4)^2*sin(the2)*sin(the3) - 2*m5*x5^2*cos(the2)*cos(the3)*cos(the5)^2*sin(the2)*sin(the3) + 2*m6*x6^2*cos(the2)*cos(the3)*cos(the4)^2*sin(the2)*sin(the3) + 4*m6*x6^2*cos(the2)*cos(the3)*cos(the6)^2*sin(the2)*sin(the3) + 2*m4*y4^2*cos(the2)*cos(the3)*cos(the4)^2*sin(the2)*sin(the3) - 2*m5*y5^2*cos(the2)*cos(the3)*cos(the4)^2*sin(the2)*sin(the3) + 2*m5*y5^2*cos(the2)*cos(the3)*cos(the5)^2*sin(the2)*sin(the3) - 2*m6*y6^2*cos(the2)*cos(the3)*cos(the5)^2*sin(the2)*sin(the3) - 4*m6*y6^2*cos(the2)*cos(the3)*cos(the6)^2*sin(the2)*sin(the3) + 2*m5*z5^2*cos(the2)*cos(the3)*cos(the4)^2*sin(the2)*sin(the3) - 2*m6*z6^2*cos(the2)*cos(the3)*cos(the4)^2*sin(the2)*sin(the3) + 2*m6*z6^2*cos(the2)*cos(the3)*cos(the5)^2*sin(the2)*sin(the3) + 2*a2*m5*x5*cos(the2)^2*cos(the3)*cos(the4)*cos(the5) - 2*a3*m6*x6*cos(the2)^2*cos(the4)*cos(the5)*cos(the6) - 2*a3*m6*x6*cos(the3)^2*cos(the4)*cos(the5)*cos(the6) - 4*a3*m5*y5*cos(the2)*cos(the3)^2*cos(the5)*sin(the2) - 2*a2*m5*y5*cos(the2)^2*cos(the3)*cos(the4)*sin(the5) - 4*a3*m5*y5*cos(the2)^2*cos(the3)*cos(the5)*sin(the3) - 2*a2*m6*y6*cos(the2)^2*cos(the3)*cos(the6)*sin(the4) + 2*a3*m6*y6*cos(the2)^2*cos(the4)*cos(the5)*sin(the6) + 2*a3*m6*y6*cos(the3)^2*cos(the4)*cos(the5)*sin(the6) - 4*a3*m6*z6*cos(the2)*cos(the3)^2*cos(the5)*sin(the2) - 2*a2*m6*z6*cos(the2)^2*cos(the3)*cos(the4)*sin(the5) - 4*a3*m6*z6*cos(the2)^2*cos(the3)*cos(the5)*sin(the3) - 4*d4*m4*x4*cos(the2)*cos(the3)^2*cos(the4)*sin(the2) - 4*d4*m4*x4*cos(the2)^2*cos(the3)*cos(the4)*sin(the3) - 4*a3*m5*x5*cos(the2)*cos(the3)^2*sin(the2)*sin(the5) - 4*a3*m5*x5*cos(the2)^2*cos(the3)*sin(the3)*sin(the5) - 2*a2*m6*x6*cos(the2)^2*cos(the3)*sin(the4)*sin(the6) - 2*a2*m6*x6*cos(the2)^2*cos(the6)*sin(the3)*sin(the5) - 8*IPz6*cos(the2)*cos(the3)^2*cos(the4)*cos(the5)^2*cos(the6)*sin(the2) - 8*IPz6*cos(the2)^2*cos(the3)*cos(the4)*cos(the5)^2*cos(the6)*sin(the3) + 4*d4*m4*y4*cos(the2)*cos(the3)^2*sin(the2)*sin(the4) + 4*d4*m4*y4*cos(the2)^2*cos(the3)*sin(the3)*sin(the4) - 4*d4*m5*z5*cos(the2)*cos(the3)^2*sin(the2)*sin(the4) - 4*d4*m5*z5*cos(the2)^2*cos(the3)*sin(the3)*sin(the4) + 4*m5*x5*y5*cos(the2)*cos(the3)^2*cos(the4)*sin(the2) + 4*m5*x5*y5*cos(the2)^2*cos(the3)*cos(the4)*sin(the3) + 4*m5*x5*y5*cos(the2)*cos(the4)*cos(the5)^2*sin(the2) + 4*m5*x5*y5*cos(the3)*cos(the4)*cos(the5)^2*sin(the3) - 2*m6*x6*y6*cos(the2)^2*cos(the4)*cos(the5)*sin(the4) - 2*m6*x6*y6*cos(the3)^2*cos(the4)*cos(the5)*sin(the4) - 4*m4*x4*z4*cos(the2)*cos(the3)^2*cos(the4)*sin(the2) - 4*m4*x4*z4*cos(the2)^2*cos(the3)*cos(the4)*sin(the3) - 2*m5*x5*z5*cos(the2)^2*cos(the4)*cos(the5)*sin(the4) - 2*m5*x5*z5*cos(the3)^2*cos(the4)*cos(the5)*sin(the4) + 2*m6*x6*z6*cos(the2)^2*cos(the5)*cos(the6)*sin(the5) + 2*m6*x6*z6*cos(the3)^2*cos(the5)*cos(the6)*sin(the5) + 2*a2*m6*y6*cos(the2)^2*sin(the3)*sin(the5)*sin(the6) + 8*IPy6*cos(the2)*cos(the3)^2*cos(the4)*cos(the5)^2*sin(the2)*sin(the6) + 8*IPy6*cos(the2)^2*cos(the3)*cos(the4)*cos(the5)^2*sin(the3)*sin(the6) + 4*IPy6*cos(the2)^2*cos(the3)^2*cos(the4)*cos(the6)*sin(the4)*sin(the5) + 2*Ixx5*cos(the2)*cos(the3)*cos(the4)^2*cos(the5)^2*sin(the2)*sin(the3) + 2*Ixx6*cos(the2)*cos(the3)*cos(the4)^2*cos(the6)^2*sin(the2)*sin(the3) + 2*Ixx6*cos(the2)*cos(the3)*cos(the5)^2*cos(the6)^2*sin(the2)*sin(the3) - 2*Iyy5*cos(the2)*cos(the3)*cos(the4)^2*cos(the5)^2*sin(the2)*sin(the3) + 2*Iyy6*cos(the2)*cos(the3)*cos(the4)^2*cos(the5)^2*sin(the2)*sin(the3) - 2*Iyy6*cos(the2)*cos(the3)*cos(the4)^2*cos(the6)^2*sin(the2)*sin(the3) - 2*Iyy6*cos(the2)*cos(the3)*cos(the5)^2*cos(the6)^2*sin(the2)*sin(the3) - 2*Izz6*cos(the2)*cos(the3)*cos(the4)^2*cos(the5)^2*sin(the2)*sin(the3) + 4*m4*y4*z4*cos(the2)*cos(the3)^2*sin(the2)*sin(the4) + 4*m4*y4*z4*cos(the2)^2*cos(the3)*sin(the3)*sin(the4) + 2*m5*y5*z5*cos(the2)^2*cos(the4)*sin(the4)*sin(the5) + 2*m5*y5*z5*cos(the3)^2*cos(the4)*sin(the4)*sin(the5) - 2*m6*y6*z6*cos(the2)^2*cos(the5)*sin(the5)*sin(the6) - 2*m6*y6*z6*cos(the3)^2*cos(the5)*sin(the5)*sin(the6) + 8*IPx6*cos(the2)*cos(the3)^2*cos(the6)^2*sin(the2)*sin(the4)*sin(the5) + 8*IPx6*cos(the2)^2*cos(the3)*cos(the6)^2*sin(the3)*sin(the4)*sin(the5) + 4*IPz6*cos(the2)^2*cos(the3)^2*cos(the4)*sin(the4)*sin(the5)*sin(the6) + 2*m6*x6^2*cos(the2)^2*cos(the3)^2*cos(the4)^2*cos(the5)^2*cos(the6)^2 - 2*m6*y6^2*cos(the2)^2*cos(the3)^2*cos(the4)^2*cos(the5)^2*cos(the6)^2 + 4*a3*m5*x5*cos(the2)^2*cos(the3)^2*cos(the4)*cos(the5) - 4*a3*m5*y5*cos(the2)^2*cos(the3)^2*cos(the4)*sin(the5) - 4*a3*m6*y6*cos(the2)^2*cos(the3)^2*cos(the6)*sin(the4) - 4*a3*m6*z6*cos(the2)^2*cos(the3)^2*cos(the4)*sin(the5) - 4*d4*m6*x6*cos(the2)^2*cos(the3)^2*cos(the6)*sin(the5) - 4*a3*m6*x6*cos(the2)^2*cos(the3)^2*sin(the4)*sin(the6) - 8*IPx6*cos(the2)^2*cos(the3)^2*cos(the4)*cos(the5)*cos(the6)^2*sin(the4) - 4*IPz6*cos(the2)^2*cos(the3)^2*cos(the4)^2*cos(the5)*cos(the6)*sin(the5) + 4*d4*m6*y6*cos(the2)^2*cos(the3)^2*sin(the5)*sin(the6) + 4*IPx4*cos(the2)*cos(the3)*cos(the4)*sin(the2)*sin(the3)*sin(the4) + 4*IPx5*cos(the2)*cos(the3)*cos(the5)*sin(the2)*sin(the3)*sin(the5) - 8*IPx6*cos(the2)*cos(the3)*cos(the6)*sin(the2)*sin(the3)*sin(the6) - 4*m4*x4*y4*cos(the2)^2*cos(the3)^2*cos(the4)*sin(the4) - 4*m5*x5*y5*cos(the2)^2*cos(the3)^2*cos(the5)*sin(the5) + 2*m5*x5*y5*cos(the2)^2*cos(the4)^2*cos(the5)*sin(the5) + 2*m5*x5*y5*cos(the3)^2*cos(the4)^2*cos(the5)*sin(the5) + 8*m6*x6*y6*cos(the2)^2*cos(the3)^2*cos(the6)*sin(the6) + 2*m6*x6*y6*cos(the2)^2*cos(the4)^2*cos(the6)*sin(the6) + 2*m6*x6*y6*cos(the2)^2*cos(the5)^2*cos(the6)*sin(the6) + 2*m6*x6*y6*cos(the3)^2*cos(the4)^2*cos(the6)*sin(the6) + 2*m6*x6*y6*cos(the3)^2*cos(the5)^2*cos(the6)*sin(the6) + 4*IPy6*cos(the2)^2*cos(the3)^2*cos(the4)^2*cos(the5)*sin(the5)*sin(the6) + 2*Ixx6*cos(the2)*cos(the6)*sin(the2)*sin(the4)*sin(the5)*sin(the6) + 2*Ixx6*cos(the3)*cos(the6)*sin(the3)*sin(the4)*sin(the5)*sin(the6) - 2*Iyy6*cos(the2)*cos(the6)*sin(the2)*sin(the4)*sin(the5)*sin(the6) - 2*Iyy6*cos(the3)*cos(the6)*sin(the3)*sin(the4)*sin(the5)*sin(the6) + 2*m5*x5^2*cos(the2)*cos(the4)*cos(the5)*sin(the2)*sin(the5) + 2*m5*x5^2*cos(the3)*cos(the4)*cos(the5)*sin(the3)*sin(the5) - 2*m5*y5^2*cos(the2)*cos(the4)*cos(the5)*sin(the2)*sin(the5) - 2*m5*y5^2*cos(the3)*cos(the4)*cos(the5)*sin(the3)*sin(the5) + 2*m6*y6^2*cos(the2)*cos(the4)*cos(the5)*sin(the2)*sin(the5) + 2*m6*y6^2*cos(the3)*cos(the4)*cos(the5)*sin(the3)*sin(the5) - 2*m6*z6^2*cos(the2)*cos(the4)*cos(the5)*sin(the2)*sin(the5) - 2*m6*z6^2*cos(the3)*cos(the4)*cos(the5)*sin(the3)*sin(the5) + 4*d4*m5*y5*cos(the2)*cos(the3)*cos(the5)*sin(the2)*sin(the3) - 2*d4*m6*y6*cos(the2)*cos(the4)*cos(the5)*sin(the2)*sin(the6) - 2*d4*m6*y6*cos(the3)*cos(the4)*cos(the5)*sin(the3)*sin(the6) + 4*d4*m6*z6*cos(the2)*cos(the3)*cos(the5)*sin(the2)*sin(the3) + 4*a3*m4*y4*cos(the2)*cos(the3)*sin(the2)*sin(the3)*sin(the4) + 2*a2*m5*y5*cos(the2)*cos(the4)*sin(the2)*sin(the3)*sin(the5) + 2*a2*m6*y6*cos(the2)*cos(the6)*sin(the2)*sin(the3)*sin(the4) + 2*a2*m6*y6*cos(the2)*cos(the3)*sin(the2)*sin(the5)*sin(the6) + 2*a1*m6*y6*cos(the4)*cos(the5)*sin(the2)*sin(the3)*sin(the6) - 4*a3*m5*z5*cos(the2)*cos(the3)*sin(the2)*sin(the3)*sin(the4) + 2*a2*m6*z6*cos(the2)*cos(the4)*sin(the2)*sin(the3)*sin(the5) + 4*d4*m5*x5*cos(the2)*cos(the3)*sin(the2)*sin(the3)*sin(the5) - 2*m6*y6*z6*cos(the2)*cos(the5)*cos(the6)*sin(the2)*sin(the4) - 2*m6*y6*z6*cos(the3)*cos(the5)*cos(the6)*sin(the3)*sin(the4) + 2*a2*m6*x6*cos(the2)*sin(the2)*sin(the3)*sin(the4)*sin(the6) + 4*IPx5*cos(the2)*cos(the3)*cos(the4)^2*cos(the5)*sin(the2)*sin(the3)*sin(the5) + 4*IPx6*cos(the2)*cos(the3)*cos(the4)^2*cos(the6)*sin(the2)*sin(the3)*sin(the6) + 4*IPx6*cos(the2)*cos(the3)*cos(the5)^2*cos(the6)*sin(the2)*sin(the3)*sin(the6) - 4*m5*x5*y5*cos(the2)^2*cos(the3)^2*cos(the4)^2*cos(the5)*sin(the5) - 4*m6*x6*y6*cos(the2)^2*cos(the3)^2*cos(the4)^2*cos(the6)*sin(the6) - 4*m6*x6*y6*cos(the2)^2*cos(the3)^2*cos(the5)^2*cos(the6)*sin(the6) + 2*m6*x6*y6*cos(the2)^2*cos(the4)^2*cos(the5)^2*cos(the6)*sin(the6) + 2*m6*x6*y6*cos(the3)^2*cos(the4)^2*cos(the5)^2*cos(the6)*sin(the6) - 2*m6*x6*z6*cos(the2)*cos(the5)*sin(the2)*sin(the4)*sin(the6) - 2*m6*x6*z6*cos(the3)*cos(the5)*sin(the3)*sin(the4)*sin(the6) - 4*Ixx6*cos(the2)*cos(the3)^2*cos(the6)*sin(the2)*sin(the4)*sin(the5)*sin(the6) - 4*Ixx6*cos(the2)^2*cos(the3)*cos(the6)*sin(the3)*sin(the4)*sin(the5)*sin(the6) + 4*Iyy6*cos(the2)*cos(the3)^2*cos(the6)*sin(the2)*sin(the4)*sin(the5)*sin(the6) + 4*Iyy6*cos(the2)^2*cos(the3)*cos(the6)*sin(the3)*sin(the4)*sin(the5)*sin(the6) - 4*m5*x5^2*cos(the2)*cos(the3)^2*cos(the4)*cos(the5)*sin(the2)*sin(the5) - 4*m5*x5^2*cos(the2)^2*cos(the3)*cos(the4)*cos(the5)*sin(the3)*sin(the5) + 2*m6*x6^2*cos(the2)*cos(the4)*cos(the5)*cos(the6)^2*sin(the2)*sin(the5) + 2*m6*x6^2*cos(the3)*cos(the4)*cos(the5)*cos(the6)^2*sin(the3)*sin(the5) + 2*m6*x6^2*cos(the2)^2*cos(the4)*cos(the5)*cos(the6)*sin(the4)*sin(the6) + 2*m6*x6^2*cos(the3)^2*cos(the4)*cos(the5)*cos(the6)*sin(the4)*sin(the6) + 4*m5*y5^2*cos(the2)*cos(the3)^2*cos(the4)*cos(the5)*sin(the2)*sin(the5) + 4*m5*y5^2*cos(the2)^2*cos(the3)*cos(the4)*cos(the5)*sin(the3)*sin(the5) - 4*m6*y6^2*cos(the2)*cos(the3)^2*cos(the4)*cos(the5)*sin(the2)*sin(the5) - 4*m6*y6^2*cos(the2)^2*cos(the3)*cos(the4)*cos(the5)*sin(the3)*sin(the5) - 2*m6*y6^2*cos(the2)*cos(the4)*cos(the5)*cos(the6)^2*sin(the2)*sin(the5) - 2*m6*y6^2*cos(the3)*cos(the4)*cos(the5)*cos(the6)^2*sin(the3)*sin(the5) - 2*m6*y6^2*cos(the2)^2*cos(the4)*cos(the5)*cos(the6)*sin(the4)*sin(the6) - 2*m6*y6^2*cos(the3)^2*cos(the4)*cos(the5)*cos(the6)*sin(the4)*sin(the6) + 4*m6*z6^2*cos(the2)*cos(the3)^2*cos(the4)*cos(the5)*sin(the2)*sin(the5) + 4*m6*z6^2*cos(the2)^2*cos(the3)*cos(the4)*cos(the5)*sin(the3)*sin(the5) + 2*a2*m6*x6*cos(the2)^2*cos(the3)*cos(the4)*cos(the5)*cos(the6) - 2*a2*m6*y6*cos(the2)^2*cos(the3)*cos(the4)*cos(the5)*sin(the6) - 4*d4*m5*x5*cos(the2)*cos(the3)^2*cos(the4)*cos(the5)*sin(the2) - 4*d4*m5*x5*cos(the2)^2*cos(the3)*cos(the4)*cos(the5)*sin(the3) - 4*a3*m6*x6*cos(the2)*cos(the3)^2*cos(the6)*sin(the2)*sin(the5) - 4*a3*m6*x6*cos(the2)^2*cos(the3)*cos(the6)*sin(the3)*sin(the5) + 4*d4*m5*y5*cos(the2)*cos(the3)^2*cos(the4)*sin(the2)*sin(the5) + 4*d4*m5*y5*cos(the2)^2*cos(the3)*cos(the4)*sin(the3)*sin(the5) + 4*d4*m6*y6*cos(the2)*cos(the3)^2*cos(the6)*sin(the2)*sin(the4) + 4*d4*m6*y6*cos(the2)^2*cos(the3)*cos(the6)*sin(the3)*sin(the4) + 4*d4*m6*z6*cos(the2)*cos(the3)^2*cos(the4)*sin(the2)*sin(the5) + 4*d4*m6*z6*cos(the2)^2*cos(the3)*cos(the4)*sin(the3)*sin(the5) + 4*m6*x6*z6*cos(the2)*cos(the3)^2*cos(the4)*cos(the6)*sin(the2) + 4*m6*x6*z6*cos(the2)^2*cos(the3)*cos(the4)*cos(the6)*sin(the3) + 4*m6*x6*z6*cos(the2)*cos(the4)*cos(the5)^2*cos(the6)*sin(the2) + 4*m6*x6*z6*cos(the3)*cos(the4)*cos(the5)^2*cos(the6)*sin(the3) + 4*a3*m6*y6*cos(the2)*cos(the3)^2*sin(the2)*sin(the5)*sin(the6) + 4*a3*m6*y6*cos(the2)^2*cos(the3)*sin(the3)*sin(the5)*sin(the6) + 4*Ixx6*cos(the2)*cos(the3)^2*cos(the4)*cos(the5)*cos(the6)^2*sin(the2)*sin(the5) + 4*Ixx6*cos(the2)^2*cos(the3)*cos(the4)*cos(the5)*cos(the6)^2*sin(the3)*sin(the5) + 4*Ixx6*cos(the2)^2*cos(the3)^2*cos(the4)*cos(the5)*cos(the6)*sin(the4)*sin(the6) - 4*Iyy6*cos(the2)*cos(the3)^2*cos(the4)*cos(the5)*cos(the6)^2*sin(the2)*sin(the5) - 4*Iyy6*cos(the2)^2*cos(the3)*cos(the4)*cos(the5)*cos(the6)^2*sin(the3)*sin(the5) - 4*Iyy6*cos(the2)^2*cos(the3)^2*cos(the4)*cos(the5)*cos(the6)*sin(the4)*sin(the6) + 4*d4*m6*x6*cos(the2)*cos(the3)^2*sin(the2)*sin(the4)*sin(the6) + 4*d4*m6*x6*cos(the2)^2*cos(the3)*sin(the3)*sin(the4)*sin(the6) - 4*m5*y5*z5*cos(the2)*cos(the3)^2*cos(the5)*sin(the2)*sin(the4) - 4*m5*y5*z5*cos(the2)^2*cos(the3)*cos(the5)*sin(the3)*sin(the4) - 4*m6*y6*z6*cos(the2)*cos(the3)^2*cos(the4)*sin(the2)*sin(the6) - 4*m6*y6*z6*cos(the2)^2*cos(the3)*cos(the4)*sin(the3)*sin(the6) - 4*m6*y6*z6*cos(the2)*cos(the4)*cos(the5)^2*sin(the2)*sin(the6) - 4*m6*y6*z6*cos(the3)*cos(the4)*cos(the5)^2*sin(the3)*sin(the6) - 2*m6*y6*z6*cos(the2)^2*cos(the4)*cos(the6)*sin(the4)*sin(the5) - 2*m6*y6*z6*cos(the3)^2*cos(the4)*cos(the6)*sin(the4)*sin(the5) - 4*m6*x6*y6*cos(the2)*cos(the3)^2*sin(the2)*sin(the4)*sin(the5) - 4*m6*x6*y6*cos(the2)^2*cos(the3)*sin(the3)*sin(the4)*sin(the5) - 4*m6*x6*y6*cos(the2)*cos(the6)^2*sin(the2)*sin(the4)*sin(the5) - 4*m6*x6*y6*cos(the3)*cos(the6)^2*sin(the3)*sin(the4)*sin(the5) - 4*m5*x5*z5*cos(the2)*cos(the3)^2*sin(the2)*sin(the4)*sin(the5) - 4*m5*x5*z5*cos(the2)^2*cos(the3)*sin(the3)*sin(the4)*sin(the5) - 2*m6*x6*z6*cos(the2)^2*cos(the4)*sin(the4)*sin(the5)*sin(the6) - 2*m6*x6*z6*cos(the3)^2*cos(the4)*sin(the4)*sin(the5)*sin(the6) - 2*m5*x5^2*cos(the2)*cos(the3)*cos(the4)^2*cos(the5)^2*sin(the2)*sin(the3) - 2*m6*x6^2*cos(the2)*cos(the3)*cos(the4)^2*cos(the6)^2*sin(the2)*sin(the3) - 2*m6*x6^2*cos(the2)*cos(the3)*cos(the5)^2*cos(the6)^2*sin(the2)*sin(the3) + 2*m5*y5^2*cos(the2)*cos(the3)*cos(the4)^2*cos(the5)^2*sin(the2)*sin(the3) - 2*m6*y6^2*cos(the2)*cos(the3)*cos(the4)^2*cos(the5)^2*sin(the2)*sin(the3) + 2*m6*y6^2*cos(the2)*cos(the3)*cos(the4)^2*cos(the6)^2*sin(the2)*sin(the3) + 2*m6*y6^2*cos(the2)*cos(the3)*cos(the5)^2*cos(the6)^2*sin(the2)*sin(the3) + 2*m6*z6^2*cos(the2)*cos(the3)*cos(the4)^2*cos(the5)^2*sin(the2)*sin(the3) + 4*a3*m6*x6*cos(the2)^2*cos(the3)^2*cos(the4)*cos(the5)*cos(the6) - 4*a3*m6*y6*cos(the2)^2*cos(the3)^2*cos(the4)*cos(the5)*sin(the6) - 4*IPx6*cos(the2)*cos(the3)*cos(the4)*cos(the5)*sin(the2)*sin(the3)*sin(the4) - 4*IPx6*cos(the2)*cos(the4)*cos(the5)*cos(the6)*sin(the2)*sin(the5)*sin(the6) - 4*IPx6*cos(the3)*cos(the4)*cos(the5)*cos(the6)*sin(the3)*sin(the5)*sin(the6) - 4*IPz5*cos(the2)*cos(the3)*cos(the4)*cos(the5)*sin(the2)*sin(the3)*sin(the4) + 4*IPz6*cos(the2)*cos(the3)*cos(the5)*cos(the6)*sin(the2)*sin(the3)*sin(the5) - 8*m5*x5*y5*cos(the2)*cos(the3)^2*cos(the4)*cos(the5)^2*sin(the2) - 8*m5*x5*y5*cos(the2)^2*cos(the3)*cos(the4)*cos(the5)^2*sin(the3) + 4*m6*x6*y6*cos(the2)^2*cos(the3)^2*cos(the4)*cos(the5)*sin(the4) + 4*m6*x6*y6*cos(the2)^2*cos(the4)*cos(the5)*cos(the6)^2*sin(the4) + 4*m6*x6*y6*cos(the3)^2*cos(the4)*cos(the5)*cos(the6)^2*sin(the4) + 4*m5*x5*z5*cos(the2)^2*cos(the3)^2*cos(the4)*cos(the5)*sin(the4) - 4*m6*x6*z6*cos(the2)^2*cos(the3)^2*cos(the5)*cos(the6)*sin(the5) + 2*m6*x6*z6*cos(the2)^2*cos(the4)^2*cos(the5)*cos(the6)*sin(the5) + 2*m6*x6*z6*cos(the3)^2*cos(the4)^2*cos(the5)*cos(the6)*sin(the5) + 2*Ixx6*cos(the2)*cos(the3)*cos(the4)^2*cos(the5)^2*cos(the6)^2*sin(the2)*sin(the3) - 2*Iyy6*cos(the2)*cos(the3)*cos(the4)^2*cos(the5)^2*cos(the6)^2*sin(the2)*sin(the3) + 4*IPy5*cos(the2)*cos(the3)*cos(the4)*sin(the2)*sin(the3)*sin(the4)*sin(the5) - 4*IPy6*cos(the2)*cos(the3)*cos(the5)*sin(the2)*sin(the3)*sin(the5)*sin(the6) - 4*m5*y5*z5*cos(the2)^2*cos(the3)^2*cos(the4)*sin(the4)*sin(the5) + 4*m6*y6*z6*cos(the2)^2*cos(the3)^2*cos(the5)*sin(the5)*sin(the6) - 2*m6*y6*z6*cos(the2)^2*cos(the4)^2*cos(the5)*sin(the5)*sin(the6) - 2*m6*y6*z6*cos(the3)^2*cos(the4)^2*cos(the5)*sin(the5)*sin(the6) + 2*a1*m6*x6*cos(the2)*cos(the3)*cos(the4)*cos(the5)*cos(the6) - 2*a1*m6*y6*cos(the2)*cos(the3)*cos(the4)*cos(the5)*sin(the6) + 2*d4*m6*x6*cos(the2)*cos(the4)*cos(the5)*cos(the6)*sin(the2) + 2*d4*m6*x6*cos(the3)*cos(the4)*cos(the5)*cos(the6)*sin(the3) - 2*m6*x6^2*cos(the2)*cos(the6)*sin(the2)*sin(the4)*sin(the5)*sin(the6) - 2*m6*x6^2*cos(the3)*cos(the6)*sin(the3)*sin(the4)*sin(the5)*sin(the6) + 2*m6*y6^2*cos(the2)*cos(the6)*sin(the2)*sin(the4)*sin(the5)*sin(the6) + 2*m6*y6^2*cos(the3)*cos(the6)*sin(the3)*sin(the4)*sin(the5)*sin(the6) - 4*a3*m4*x4*cos(the2)*cos(the3)*cos(the4)*sin(the2)*sin(the3) - 2*a2*m5*x5*cos(the2)*cos(the4)*cos(the5)*sin(the2)*sin(the3) - 2*a2*m6*x6*cos(the2)*cos(the3)*cos(the6)*sin(the2)*sin(the5) - 2*a1*m6*x6*cos(the4)*cos(the5)*cos(the6)*sin(the2)*sin(the3) - 4*IPy6*cos(the2)*cos(the3)*cos(the4)^2*cos(the5)*sin(the2)*sin(the3)*sin(the5)*sin(the6) + 4*m6*y6*z6*cos(the2)^2*cos(the3)^2*cos(the4)^2*cos(the5)*sin(the5)*sin(the6) - 4*d4*m6*x6*cos(the2)*cos(the3)^2*cos(the4)*cos(the5)*cos(the6)*sin(the2) - 4*d4*m6*x6*cos(the2)^2*cos(the3)*cos(the4)*cos(the5)*cos(the6)*sin(the3) + 4*m6*x6^2*cos(the2)*cos(the3)^2*cos(the6)*sin(the2)*sin(the4)*sin(the5)*sin(the6) + 4*m6*x6^2*cos(the2)^2*cos(the3)*cos(the6)*sin(the3)*sin(the4)*sin(the5)*sin(the6) - 4*m6*y6^2*cos(the2)*cos(the3)^2*cos(the6)*sin(the2)*sin(the4)*sin(the5)*sin(the6) - 4*m6*y6^2*cos(the2)^2*cos(the3)*cos(the6)*sin(the3)*sin(the4)*sin(the5)*sin(the6) + 4*d4*m6*y6*cos(the2)*cos(the3)^2*cos(the4)*cos(the5)*sin(the2)*sin(the6) + 4*d4*m6*y6*cos(the2)^2*cos(the3)*cos(the4)*cos(the5)*sin(the3)*sin(the6) + 4*m6*y6*z6*cos(the2)*cos(the3)^2*cos(the5)*cos(the6)*sin(the2)*sin(the4) + 4*m6*y6*z6*cos(the2)^2*cos(the3)*cos(the5)*cos(the6)*sin(the3)*sin(the4) + 4*IPx6*cos(the2)*cos(the3)*cos(the4)^2*cos(the5)^2*cos(the6)*sin(the2)*sin(the3)*sin(the6) - 4*m6*x6*y6*cos(the2)^2*cos(the3)^2*cos(the4)^2*cos(the5)^2*cos(the6)*sin(the6) + 4*m6*x6*z6*cos(the2)*cos(the3)^2*cos(the5)*sin(the2)*sin(the4)*sin(the6) + 4*m6*x6*z6*cos(the2)^2*cos(the3)*cos(the5)*sin(the3)*sin(the4)*sin(the6) - 4*m6*x6^2*cos(the2)*cos(the3)^2*cos(the4)*cos(the5)*cos(the6)^2*sin(the2)*sin(the5) - 4*m6*x6^2*cos(the2)^2*cos(the3)*cos(the4)*cos(the5)*cos(the6)^2*sin(the3)*sin(the5) - 4*m6*x6^2*cos(the2)^2*cos(the3)^2*cos(the4)*cos(the5)*cos(the6)*sin(the4)*sin(the6) + 4*m6*y6^2*cos(the2)*cos(the3)^2*cos(the4)*cos(the5)*cos(the6)^2*sin(the2)*sin(the5) + 4*m6*y6^2*cos(the2)^2*cos(the3)*cos(the4)*cos(the5)*cos(the6)^2*sin(the3)*sin(the5) + 4*m6*y6^2*cos(the2)^2*cos(the3)^2*cos(the4)*cos(the5)*cos(the6)*sin(the4)*sin(the6) - 8*m6*x6*z6*cos(the2)*cos(the3)^2*cos(the4)*cos(the5)^2*cos(the6)*sin(the2) - 8*m6*x6*z6*cos(the2)^2*cos(the3)*cos(the4)*cos(the5)^2*cos(the6)*sin(the3) - 4*IPy6*cos(the2)*cos(the3)*cos(the4)*cos(the6)*sin(the2)*sin(the3)*sin(the4)*sin(the5) + 8*m6*y6*z6*cos(the2)*cos(the3)^2*cos(the4)*cos(the5)^2*sin(the2)*sin(the6) + 8*m6*y6*z6*cos(the2)^2*cos(the3)*cos(the4)*cos(the5)^2*sin(the3)*sin(the6) + 4*m6*y6*z6*cos(the2)^2*cos(the3)^2*cos(the4)*cos(the6)*sin(the4)*sin(the5) - 4*IPz6*cos(the2)*cos(the3)*cos(the4)*sin(the2)*sin(the3)*sin(the4)*sin(the5)*sin(the6) + 8*m6*x6*y6*cos(the2)*cos(the3)^2*cos(the6)^2*sin(the2)*sin(the4)*sin(the5) + 8*m6*x6*y6*cos(the2)^2*cos(the3)*cos(the6)^2*sin(the3)*sin(the4)*sin(the5) + 4*m6*x6*z6*cos(the2)^2*cos(the3)^2*cos(the4)*sin(the4)*sin(the5)*sin(the6) - 2*m6*x6^2*cos(the2)*cos(the3)*cos(the4)^2*cos(the5)^2*cos(the6)^2*sin(the2)*sin(the3) + 2*m6*y6^2*cos(the2)*cos(the3)*cos(the4)^2*cos(the5)^2*cos(the6)^2*sin(the2)*sin(the3) - 4*a3*m5*x5*cos(the2)*cos(the3)*cos(the4)*cos(the5)*sin(the2)*sin(the3) - 2*a2*m6*x6*cos(the2)*cos(the4)*cos(the5)*cos(the6)*sin(the2)*sin(the3) + 4*a3*m5*y5*cos(the2)*cos(the3)*cos(the4)*sin(the2)*sin(the3)*sin(the5) + 4*a3*m6*y6*cos(the2)*cos(the3)*cos(the6)*sin(the2)*sin(the3)*sin(the4) + 2*a2*m6*y6*cos(the2)*cos(the4)*cos(the5)*sin(the2)*sin(the3)*sin(the6) + 4*a3*m6*z6*cos(the2)*cos(the3)*cos(the4)*sin(the2)*sin(the3)*sin(the5) + 4*d4*m6*x6*cos(the2)*cos(the3)*cos(the6)*sin(the2)*sin(the3)*sin(the5) + 4*a3*m6*x6*cos(the2)*cos(the3)*sin(the2)*sin(the3)*sin(the4)*sin(the6) + 8*IPx6*cos(the2)*cos(the3)*cos(the4)*cos(the5)*cos(the6)^2*sin(the2)*sin(the3)*sin(the4) + 8*IPx6*cos(the2)*cos(the3)^2*cos(the4)*cos(the5)*cos(the6)*sin(the2)*sin(the5)*sin(the6) + 8*IPx6*cos(the2)^2*cos(the3)*cos(the4)*cos(the5)*cos(the6)*sin(the3)*sin(the5)*sin(the6) + 4*IPz6*cos(the2)*cos(the3)*cos(the4)^2*cos(the5)*cos(the6)*sin(the2)*sin(the3)*sin(the5) - 4*d4*m6*y6*cos(the2)*cos(the3)*sin(the2)*sin(the3)*sin(the5)*sin(the6) - 8*m6*x6*y6*cos(the2)^2*cos(the3)^2*cos(the4)*cos(the5)*cos(the6)^2*sin(the4) - 4*m6*x6*z6*cos(the2)^2*cos(the3)^2*cos(the4)^2*cos(the5)*cos(the6)*sin(the5) + 4*m4*x4*y4*cos(the2)*cos(the3)*cos(the4)*sin(the2)*sin(the3)*sin(the4) + 4*m5*x5*y5*cos(the2)*cos(the3)*cos(the5)*sin(the2)*sin(the3)*sin(the5) - 8*m6*x6*y6*cos(the2)*cos(the3)*cos(the6)*sin(the2)*sin(the3)*sin(the6) + 4*m5*x5*y5*cos(the2)*cos(the3)*cos(the4)^2*cos(the5)*sin(the2)*sin(the3)*sin(the5) + 4*m6*x6*y6*cos(the2)*cos(the3)*cos(the4)^2*cos(the6)*sin(the2)*sin(the3)*sin(the6) + 4*m6*x6*y6*cos(the2)*cos(the3)*cos(the5)^2*cos(the6)*sin(the2)*sin(the3)*sin(the6) - 4*Ixx6*cos(the2)*cos(the3)*cos(the4)*cos(the5)*cos(the6)*sin(the2)*sin(the3)*sin(the4)*sin(the6) + 4*Iyy6*cos(the2)*cos(the3)*cos(the4)*cos(the5)*cos(the6)*sin(the2)*sin(the3)*sin(the4)*sin(the6) - 4*a3*m6*x6*cos(the2)*cos(the3)*cos(the4)*cos(the5)*cos(the6)*sin(the2)*sin(the3) + 4*a3*m6*y6*cos(the2)*cos(the3)*cos(the4)*cos(the5)*sin(the2)*sin(the3)*sin(the6) - 4*m6*x6*y6*cos(the2)*cos(the3)*cos(the4)*cos(the5)*sin(the2)*sin(the3)*sin(the4) - 4*m6*x6*y6*cos(the2)*cos(the4)*cos(the5)*cos(the6)*sin(the2)*sin(the5)*sin(the6) - 4*m6*x6*y6*cos(the3)*cos(the4)*cos(the5)*cos(the6)*sin(the3)*sin(the5)*sin(the6) - 4*m5*x5*z5*cos(the2)*cos(the3)*cos(the4)*cos(the5)*sin(the2)*sin(the3)*sin(the4) + 4*m6*x6*z6*cos(the2)*cos(the3)*cos(the5)*cos(the6)*sin(the2)*sin(the3)*sin(the5) + 4*m5*y5*z5*cos(the2)*cos(the3)*cos(the4)*sin(the2)*sin(the3)*sin(the4)*sin(the5) - 4*m6*y6*z6*cos(the2)*cos(the3)*cos(the5)*sin(the2)*sin(the3)*sin(the5)*sin(the6) + 8*m6*x6*y6*cos(the2)*cos(the3)*cos(the4)*cos(the5)*cos(the6)^2*sin(the2)*sin(the3)*sin(the4) + 8*m6*x6*y6*cos(the2)*cos(the3)^2*cos(the4)*cos(the5)*cos(the6)*sin(the2)*sin(the5)*sin(the6) + 8*m6*x6*y6*cos(the2)^2*cos(the3)*cos(the4)*cos(the5)*cos(the6)*sin(the3)*sin(the5)*sin(the6) + 4*m6*x6*z6*cos(the2)*cos(the3)*cos(the4)^2*cos(the5)*cos(the6)*sin(the2)*sin(the3)*sin(the5) - 4*m6*y6*z6*cos(the2)*cos(the3)*cos(the4)^2*cos(the5)*sin(the2)*sin(the3)*sin(the5)*sin(the6) + 4*m6*x6*y6*cos(the2)*cos(the3)*cos(the4)^2*cos(the5)^2*cos(the6)*sin(the2)*sin(the3)*sin(the6) + 4*m6*x6^2*cos(the2)*cos(the3)*cos(the4)*cos(the5)*cos(the6)*sin(the2)*sin(the3)*sin(the4)*sin(the6) - 4*m6*y6^2*cos(the2)*cos(the3)*cos(the4)*cos(the5)*cos(the6)*sin(the2)*sin(the3)*sin(the4)*sin(the6) - 4*m6*y6*z6*cos(the2)*cos(the3)*cos(the4)*cos(the6)*sin(the2)*sin(the3)*sin(the4)*sin(the5) - 4*m6*x6*z6*cos(the2)*cos(the3)*cos(the4)*sin(the2)*sin(the3)*sin(the4)*sin(the5)*sin(the6),IPy2*cos(the2) + IPz2*sin(the2) + IPy3*cos(the2)*cos(the3) + IPx4*cos(the2)*sin(the3) + IPx4*cos(the3)*sin(the2) + IPz3*cos(the2)*sin(the3) + IPz3*cos(the3)*sin(the2) - IPy3*sin(the2)*sin(the3) - IPy4*cos(the2)*cos(the3)*cos(the4) + IPx5*cos(the2)*cos(the3)*sin(the4) - IPx6*cos(the2)*cos(the5)*sin(the3) - IPx6*cos(the3)*cos(the5)*sin(the2) - IPz4*cos(the2)*cos(the3)*sin(the4) - IPz5*cos(the2)*cos(the5)*sin(the3) - IPz5*cos(the3)*cos(the5)*sin(the2) + IPy4*cos(the4)*sin(the2)*sin(the3) + IPy5*cos(the2)*sin(the3)*sin(the5) + IPy5*cos(the3)*sin(the2)*sin(the5) - IPx5*sin(the2)*sin(the3)*sin(the4) + IPz4*sin(the2)*sin(the3)*sin(the4) + a2*m3*z3*sin(the2) + m2*y2*z2*cos(the2) - 2*IPx4*cos(the2)*cos(the4)^2*sin(the3) - 2*IPx4*cos(the3)*cos(the4)^2*sin(the2) + m2*x2*z2*sin(the2) + IPy5*cos(the2)*cos(the3)*cos(the4)*cos(the5) + IPx6*cos(the2)*cos(the3)*cos(the4)*sin(the5) + IPz5*cos(the2)*cos(the3)*cos(the4)*sin(the5) + IPz6*cos(the2)*cos(the3)*cos(the6)*sin(the4) - IPy5*cos(the4)*cos(the5)*sin(the2)*sin(the3) - IPy6*cos(the2)*cos(the3)*sin(the4)*sin(the6) - IPy6*cos(the2)*cos(the6)*sin(the3)*sin(the5) - IPy6*cos(the3)*cos(the6)*sin(the2)*sin(the5) + Ixx4*cos(the2)*cos(the4)*sin(the3)*sin(the4) + Ixx4*cos(the3)*cos(the4)*sin(the2)*sin(the4) - Ixx6*cos(the2)*cos(the4)*sin(the3)*sin(the4) - Ixx6*cos(the3)*cos(the4)*sin(the2)*sin(the4) - Iyy4*cos(the2)*cos(the4)*sin(the3)*sin(the4) - Iyy4*cos(the3)*cos(the4)*sin(the2)*sin(the4) + Iyy5*cos(the2)*cos(the4)*sin(the3)*sin(the4) + Iyy5*cos(the3)*cos(the4)*sin(the2)*sin(the4) - Izz5*cos(the2)*cos(the4)*sin(the3)*sin(the4) - Izz5*cos(the3)*cos(the4)*sin(the2)*sin(the4) + Izz6*cos(the2)*cos(the4)*sin(the3)*sin(the4) + Izz6*cos(the3)*cos(the4)*sin(the2)*sin(the4) - IPx6*cos(the4)*sin(the2)*sin(the3)*sin(the5) - IPz5*cos(the4)*sin(the2)*sin(the3)*sin(the5) - IPz6*cos(the6)*sin(the2)*sin(the3)*sin(the4) - IPz6*cos(the2)*sin(the3)*sin(the5)*sin(the6) - IPz6*cos(the3)*sin(the2)*sin(the5)*sin(the6) + IPy6*sin(the2)*sin(the3)*sin(the4)*sin(the6) - a2*m4*y4*cos(the4)*sin(the2) + a2*m5*z5*cos(the4)*sin(the2) + m3*y3*z3*cos(the2)*cos(the3) - a2*m4*x4*sin(the2)*sin(the4) - 2*IPx5*cos(the2)*cos(the3)*cos(the5)^2*sin(the4) + 2*IPx6*cos(the2)*cos(the4)^2*cos(the5)*sin(the3) + 2*IPx6*cos(the3)*cos(the4)^2*cos(the5)*sin(the2) + 2*IPx6*cos(the2)*cos(the5)*cos(the6)^2*sin(the3) + 2*IPx6*cos(the3)*cos(the5)*cos(the6)^2*sin(the2) + 2*IPz5*cos(the2)*cos(the4)^2*cos(the5)*sin(the3) + 2*IPz5*cos(the3)*cos(the4)^2*cos(the5)*sin(the2) + m4*x4*y4*cos(the2)*sin(the3) + m4*x4*y4*cos(the3)*sin(the2) + m3*x3*z3*cos(the2)*sin(the3) + m3*x3*z3*cos(the3)*sin(the2) - 2*IPy5*cos(the2)*cos(the4)^2*sin(the3)*sin(the5) - 2*IPy5*cos(the3)*cos(the4)^2*sin(the2)*sin(the5) - m3*y3*z3*sin(the2)*sin(the3) + 2*IPx5*cos(the5)^2*sin(the2)*sin(the3)*sin(the4) + Ixx5*cos(the2)*cos(the3)*cos(the5)*sin(the4)*sin(the5) - Ixx6*cos(the2)*cos(the5)*cos(the6)*sin(the3)*sin(the6) - Ixx6*cos(the3)*cos(the5)*cos(the6)*sin(the2)*sin(the6) - Iyy5*cos(the2)*cos(the3)*cos(the5)*sin(the4)*sin(the5) + Iyy6*cos(the2)*cos(the3)*cos(the5)*sin(the4)*sin(the5) + Iyy6*cos(the2)*cos(the5)*cos(the6)*sin(the3)*sin(the6) + Iyy6*cos(the3)*cos(the5)*cos(the6)*sin(the2)*sin(the6) - Izz6*cos(the2)*cos(the3)*cos(the5)*sin(the4)*sin(the5) + IPz6*cos(the4)*cos(the5)*sin(the2)*sin(the3)*sin(the6) - Ixx5*cos(the5)*sin(the2)*sin(the3)*sin(the4)*sin(the5) + Iyy5*cos(the5)*sin(the2)*sin(the3)*sin(the4)*sin(the5) - Iyy6*cos(the5)*sin(the2)*sin(the3)*sin(the4)*sin(the5) + Izz6*cos(the5)*sin(the2)*sin(the3)*sin(the4)*sin(the5) - m4*x4^2*cos(the2)*cos(the4)*sin(the3)*sin(the4) - m4*x4^2*cos(the3)*cos(the4)*sin(the2)*sin(the4) + m6*x6^2*cos(the2)*cos(the4)*sin(the3)*sin(the4) + m6*x6^2*cos(the3)*cos(the4)*sin(the2)*sin(the4) + m4*y4^2*cos(the2)*cos(the4)*sin(the3)*sin(the4) + m4*y4^2*cos(the3)*cos(the4)*sin(the2)*sin(the4) - m5*y5^2*cos(the2)*cos(the4)*sin(the3)*sin(the4) - m5*y5^2*cos(the3)*cos(the4)*sin(the2)*sin(the4) + m5*z5^2*cos(the2)*cos(the4)*sin(the3)*sin(the4) + m5*z5^2*cos(the3)*cos(the4)*sin(the2)*sin(the4) - m6*z6^2*cos(the2)*cos(the4)*sin(the3)*sin(the4) - m6*z6^2*cos(the3)*cos(the4)*sin(the2)*sin(the4) - d4*m4*y4*cos(the2)*cos(the3)*cos(the4) + d4*m5*z5*cos(the2)*cos(the3)*cos(the4) - a3*m4*y4*cos(the2)*cos(the4)*sin(the3) - a3*m4*y4*cos(the3)*cos(the4)*sin(the2) - a2*m6*y6*cos(the4)*cos(the6)*sin(the2) + a3*m5*z5*cos(the2)*cos(the4)*sin(the3) + a3*m5*z5*cos(the3)*cos(the4)*sin(the2) - d4*m4*x4*cos(the2)*cos(the3)*sin(the4) - m4*y4*z4*cos(the2)*cos(the3)*cos(the4) - a3*m4*x4*cos(the2)*sin(the3)*sin(the4) - a3*m4*x4*cos(the3)*sin(the2)*sin(the4) - a2*m5*x5*cos(the5)*sin(the2)*sin(the4) - a2*m6*x6*cos(the4)*sin(the2)*sin(the6) - 2*IPx6*cos(the2)*cos(the3)*cos(the4)*cos(the6)^2*sin(the5) - 2*IPz6*cos(the2)*cos(the3)*cos(the5)^2*cos(the6)*sin(the4) + d4*m4*y4*cos(the4)*sin(the2)*sin(the3) - d4*m5*z5*cos(the4)*sin(the2)*sin(the3) + m5*x5*y5*cos(the2)*cos(the3)*sin(the4) - m6*x6*y6*cos(the2)*cos(the5)*sin(the3) - m6*x6*y6*cos(the3)*cos(the5)*sin(the2) - m4*x4*z4*cos(the2)*cos(the3)*sin(the4) - m5*x5*z5*cos(the2)*cos(the5)*sin(the3) - m5*x5*z5*cos(the3)*cos(the5)*sin(the2) + a2*m5*y5*sin(the2)*sin(the4)*sin(the5) + a2*m6*z6*sin(the2)*sin(the4)*sin(the5) + 2*IPy6*cos(the2)*cos(the3)*cos(the5)^2*sin(the4)*sin(the6) + 2*IPy6*cos(the2)*cos(the4)^2*cos(the6)*sin(the3)*sin(the5) + 2*IPy6*cos(the3)*cos(the4)^2*cos(the6)*sin(the2)*sin(the5) + Ixx5*cos(the2)*cos(the4)*cos(the5)^2*sin(the3)*sin(the4) + Ixx5*cos(the3)*cos(the4)*cos(the5)^2*sin(the2)*sin(the4) + Ixx6*cos(the2)*cos(the4)*cos(the6)^2*sin(the3)*sin(the4) + Ixx6*cos(the3)*cos(the4)*cos(the6)^2*sin(the2)*sin(the4) - Iyy5*cos(the2)*cos(the4)*cos(the5)^2*sin(the3)*sin(the4) - Iyy5*cos(the3)*cos(the4)*cos(the5)^2*sin(the2)*sin(the4) + Iyy6*cos(the2)*cos(the4)*cos(the5)^2*sin(the3)*sin(the4) + Iyy6*cos(the3)*cos(the4)*cos(the5)^2*sin(the2)*sin(the4) - Iyy6*cos(the2)*cos(the4)*cos(the6)^2*sin(the3)*sin(the4) - Iyy6*cos(the3)*cos(the4)*cos(the6)^2*sin(the2)*sin(the4) - Izz6*cos(the2)*cos(the4)*cos(the5)^2*sin(the3)*sin(the4) - Izz6*cos(the3)*cos(the4)*cos(the5)^2*sin(the2)*sin(the4) + d4*m4*x4*sin(the2)*sin(the3)*sin(the4) + m4*y4*z4*cos(the4)*sin(the2)*sin(the3) + m5*y5*z5*cos(the2)*sin(the3)*sin(the5) + m5*y5*z5*cos(the3)*sin(the2)*sin(the5) + 2*IPx6*cos(the4)*cos(the6)^2*sin(the2)*sin(the3)*sin(the5) + 2*IPz6*cos(the2)*cos(the4)^2*sin(the3)*sin(the5)*sin(the6) + 2*IPz6*cos(the3)*cos(the4)^2*sin(the2)*sin(the5)*sin(the6) + 2*IPz6*cos(the5)^2*cos(the6)*sin(the2)*sin(the3)*sin(the4) - m5*x5*y5*sin(the2)*sin(the3)*sin(the4) + m4*x4*z4*sin(the2)*sin(the3)*sin(the4) - 2*IPy6*cos(the5)^2*sin(the2)*sin(the3)*sin(the4)*sin(the6) - 4*IPx6*cos(the2)*cos(the4)^2*cos(the5)*cos(the6)^2*sin(the3) - 4*IPx6*cos(the3)*cos(the4)^2*cos(the5)*cos(the6)^2*sin(the2) - 2*m4*x4*y4*cos(the2)*cos(the4)^2*sin(the3) - 2*m4*x4*y4*cos(the3)*cos(the4)^2*sin(the2) - IPy6*cos(the2)*cos(the3)*cos(the4)*cos(the5)*cos(the6) - IPz6*cos(the2)*cos(the3)*cos(the4)*cos(the5)*sin(the6) + IPy6*cos(the4)*cos(the5)*cos(the6)*sin(the2)*sin(the3) - d4*m6*y6*cos(the2)*cos(the3)*cos(the4)*cos(the6) - a3*m6*y6*cos(the2)*cos(the4)*cos(the6)*sin(the3) - a3*m6*y6*cos(the3)*cos(the4)*cos(the6)*sin(the2) - d4*m5*x5*cos(the2)*cos(the3)*cos(the5)*sin(the4) - d4*m6*x6*cos(the2)*cos(the3)*cos(the4)*sin(the6) + m5*x5^2*cos(the5)*sin(the2)*sin(the3)*sin(the4)*sin(the5) - m5*y5^2*cos(the5)*sin(the2)*sin(the3)*sin(the4)*sin(the5) + m6*y6^2*cos(the5)*sin(the2)*sin(the3)*sin(the4)*sin(the5) - m6*z6^2*cos(the5)*sin(the2)*sin(the3)*sin(the4)*sin(the5) + m5*y5*z5*cos(the2)*cos(the3)*cos(the4)*cos(the5) - a3*m5*x5*cos(the2)*cos(the5)*sin(the3)*sin(the4) - a3*m5*x5*cos(the3)*cos(the5)*sin(the2)*sin(the4) - a3*m6*x6*cos(the2)*cos(the4)*sin(the3)*sin(the6) - a3*m6*x6*cos(the3)*cos(the4)*sin(the2)*sin(the6) - a2*m6*x6*cos(the5)*cos(the6)*sin(the2)*sin(the4) + d4*m5*y5*cos(the2)*cos(the3)*sin(the4)*sin(the5) + d4*m6*y6*cos(the4)*cos(the6)*sin(the2)*sin(the3) + d4*m6*z6*cos(the2)*cos(the3)*sin(the4)*sin(the5) + m6*x6*y6*cos(the2)*cos(the3)*cos(the4)*sin(the5) + m5*x5*z5*cos(the2)*cos(the3)*cos(the4)*sin(the5) + m6*x6*z6*cos(the2)*cos(the3)*cos(the6)*sin(the4) + a3*m5*y5*cos(the2)*sin(the3)*sin(the4)*sin(the5) + a3*m5*y5*cos(the3)*sin(the2)*sin(the4)*sin(the5) + a2*m6*y6*cos(the5)*sin(the2)*sin(the4)*sin(the6) + a3*m6*z6*cos(the2)*sin(the3)*sin(the4)*sin(the5) + a3*m6*z6*cos(the3)*sin(the2)*sin(the4)*sin(the5) + Ixx6*cos(the2)*cos(the3)*cos(the5)*cos(the6)^2*sin(the4)*sin(the5) + 2*Ixx6*cos(the2)*cos(the4)^2*cos(the5)*cos(the6)*sin(the3)*sin(the6) + 2*Ixx6*cos(the3)*cos(the4)^2*cos(the5)*cos(the6)*sin(the2)*sin(the6) - Iyy6*cos(the2)*cos(the3)*cos(the5)*cos(the6)^2*sin(the4)*sin(the5) - 2*Iyy6*cos(the2)*cos(the4)^2*cos(the5)*cos(the6)*sin(the3)*sin(the6) - 2*Iyy6*cos(the3)*cos(the4)^2*cos(the5)*cos(the6)*sin(the2)*sin(the6) + d4*m5*x5*cos(the5)*sin(the2)*sin(the3)*sin(the4) + d4*m6*x6*cos(the4)*sin(the2)*sin(the3)*sin(the6) - m5*y5*z5*cos(the4)*cos(the5)*sin(the2)*sin(the3) - m6*y6*z6*cos(the2)*cos(the3)*sin(the4)*sin(the6) - m6*y6*z6*cos(the2)*cos(the6)*sin(the3)*sin(the5) - m6*y6*z6*cos(the3)*cos(the6)*sin(the2)*sin(the5) - d4*m5*y5*sin(the2)*sin(the3)*sin(the4)*sin(the5) - d4*m6*z6*sin(the2)*sin(the3)*sin(the4)*sin(the5) - m6*x6*y6*cos(the4)*sin(the2)*sin(the3)*sin(the5) - m5*x5*z5*cos(the4)*sin(the2)*sin(the3)*sin(the5) - m6*x6*z6*cos(the6)*sin(the2)*sin(the3)*sin(the4) - m6*x6*z6*cos(the2)*sin(the3)*sin(the5)*sin(the6) - m6*x6*z6*cos(the3)*sin(the2)*sin(the5)*sin(the6) - Ixx6*cos(the5)*cos(the6)^2*sin(the2)*sin(the3)*sin(the4)*sin(the5) + Iyy6*cos(the5)*cos(the6)^2*sin(the2)*sin(the3)*sin(the4)*sin(the5) - m5*x5^2*cos(the2)*cos(the4)*cos(the5)^2*sin(the3)*sin(the4) - m5*x5^2*cos(the3)*cos(the4)*cos(the5)^2*sin(the2)*sin(the4) - m6*x6^2*cos(the2)*cos(the4)*cos(the6)^2*sin(the3)*sin(the4) - m6*x6^2*cos(the3)*cos(the4)*cos(the6)^2*sin(the2)*sin(the4) + m5*y5^2*cos(the2)*cos(the4)*cos(the5)^2*sin(the3)*sin(the4) + m5*y5^2*cos(the3)*cos(the4)*cos(the5)^2*sin(the2)*sin(the4) - m6*y6^2*cos(the2)*cos(the4)*cos(the5)^2*sin(the3)*sin(the4) - m6*y6^2*cos(the3)*cos(the4)*cos(the5)^2*sin(the2)*sin(the4) + m6*y6^2*cos(the2)*cos(the4)*cos(the6)^2*sin(the3)*sin(the4) + m6*y6^2*cos(the3)*cos(the4)*cos(the6)^2*sin(the2)*sin(the4) + m6*z6^2*cos(the2)*cos(the4)*cos(the5)^2*sin(the3)*sin(the4) + m6*z6^2*cos(the3)*cos(the4)*cos(the5)^2*sin(the2)*sin(the4) + m6*y6*z6*sin(the2)*sin(the3)*sin(the4)*sin(the6) - 2*m5*x5*y5*cos(the2)*cos(the3)*cos(the5)^2*sin(the4) + 2*m6*x6*y6*cos(the2)*cos(the4)^2*cos(the5)*sin(the3) + 2*m6*x6*y6*cos(the3)*cos(the4)^2*cos(the5)*sin(the2) + 2*m6*x6*y6*cos(the2)*cos(the5)*cos(the6)^2*sin(the3) + 2*m6*x6*y6*cos(the3)*cos(the5)*cos(the6)^2*sin(the2) + 2*m5*x5*z5*cos(the2)*cos(the4)^2*cos(the5)*sin(the3) + 2*m5*x5*z5*cos(the3)*cos(the4)^2*cos(the5)*sin(the2) + Ixx6*cos(the2)*cos(the4)*cos(the5)^2*cos(the6)^2*sin(the3)*sin(the4) + Ixx6*cos(the3)*cos(the4)*cos(the5)^2*cos(the6)^2*sin(the2)*sin(the4) - Iyy6*cos(the2)*cos(the4)*cos(the5)^2*cos(the6)^2*sin(the3)*sin(the4) - Iyy6*cos(the3)*cos(the4)*cos(the5)^2*cos(the6)^2*sin(the2)*sin(the4) - 2*m5*y5*z5*cos(the2)*cos(the4)^2*sin(the3)*sin(the5) - 2*m5*y5*z5*cos(the3)*cos(the4)^2*sin(the2)*sin(the5) + 2*m5*x5*y5*cos(the5)^2*sin(the2)*sin(the3)*sin(the4) + Ixx6*cos(the2)*cos(the3)*cos(the4)*cos(the6)*sin(the5)*sin(the6) - Iyy6*cos(the2)*cos(the3)*cos(the4)*cos(the6)*sin(the5)*sin(the6) + 2*IPx5*cos(the2)*cos(the4)*cos(the5)*sin(the3)*sin(the4)*sin(the5) + 2*IPx5*cos(the3)*cos(the4)*cos(the5)*sin(the2)*sin(the4)*sin(the5) + 2*IPx6*cos(the2)*cos(the4)*cos(the6)*sin(the3)*sin(the4)*sin(the6) + 2*IPx6*cos(the3)*cos(the4)*cos(the6)*sin(the2)*sin(the4)*sin(the6) - Ixx6*cos(the4)*cos(the6)*sin(the2)*sin(the3)*sin(the5)*sin(the6) + Iyy6*cos(the4)*cos(the6)*sin(the2)*sin(the3)*sin(the5)*sin(the6) - m5*x5^2*cos(the2)*cos(the3)*cos(the5)*sin(the4)*sin(the5) + m6*x6^2*cos(the2)*cos(the5)*cos(the6)*sin(the3)*sin(the6) + m6*x6^2*cos(the3)*cos(the5)*cos(the6)*sin(the2)*sin(the6) + m5*y5^2*cos(the2)*cos(the3)*cos(the5)*sin(the4)*sin(the5) - m6*y6^2*cos(the2)*cos(the3)*cos(the5)*sin(the4)*sin(the5) - m6*y6^2*cos(the2)*cos(the5)*cos(the6)*sin(the3)*sin(the6) - m6*y6^2*cos(the3)*cos(the5)*cos(the6)*sin(the2)*sin(the6) + m6*z6^2*cos(the2)*cos(the3)*cos(the5)*sin(the4)*sin(the5) + d4*m6*y6*cos(the2)*cos(the3)*cos(the5)*sin(the4)*sin(the6) - m6*x6*z6*cos(the2)*cos(the3)*cos(the4)*cos(the5)*sin(the6) + a3*m6*y6*cos(the2)*cos(the5)*sin(the3)*sin(the4)*sin(the6) + a3*m6*y6*cos(the3)*cos(the5)*sin(the2)*sin(the4)*sin(the6) + d4*m6*x6*cos(the5)*cos(the6)*sin(the2)*sin(the3)*sin(the4) + m6*y6*z6*cos(the4)*cos(the5)*cos(the6)*sin(the2)*sin(the3) + 2*IPx6*cos(the2)*cos(the4)*cos(the5)^2*cos(the6)*sin(the3)*sin(the4)*sin(the6) + 2*IPx6*cos(the3)*cos(the4)*cos(the5)^2*cos(the6)*sin(the2)*sin(the4)*sin(the6) - d4*m6*y6*cos(the5)*sin(the2)*sin(the3)*sin(the4)*sin(the6) + m6*x6*z6*cos(the4)*cos(the5)*sin(the2)*sin(the3)*sin(the6) - m6*x6^2*cos(the2)*cos(the3)*cos(the5)*cos(the6)^2*sin(the4)*sin(the5) - 2*m6*x6^2*cos(the2)*cos(the4)^2*cos(the5)*cos(the6)*sin(the3)*sin(the6) - 2*m6*x6^2*cos(the3)*cos(the4)^2*cos(the5)*cos(the6)*sin(the2)*sin(the6) + m6*y6^2*cos(the2)*cos(the3)*cos(the5)*cos(the6)^2*sin(the4)*sin(the5) + 2*m6*y6^2*cos(the2)*cos(the4)^2*cos(the5)*cos(the6)*sin(the3)*sin(the6) + 2*m6*y6^2*cos(the3)*cos(the4)^2*cos(the5)*cos(the6)*sin(the2)*sin(the6) + m6*x6^2*cos(the5)*cos(the6)^2*sin(the2)*sin(the3)*sin(the4)*sin(the5) - m6*y6^2*cos(the5)*cos(the6)^2*sin(the2)*sin(the3)*sin(the4)*sin(the5) - 2*m6*x6*y6*cos(the2)*cos(the3)*cos(the4)*cos(the6)^2*sin(the5) - 2*m6*x6*z6*cos(the2)*cos(the3)*cos(the5)^2*cos(the6)*sin(the4) + 2*m6*y6*z6*cos(the2)*cos(the3)*cos(the5)^2*sin(the4)*sin(the6) + 2*m6*y6*z6*cos(the2)*cos(the4)^2*cos(the6)*sin(the3)*sin(the5) + 2*m6*y6*z6*cos(the3)*cos(the4)^2*cos(the6)*sin(the2)*sin(the5) + 2*m6*x6*y6*cos(the4)*cos(the6)^2*sin(the2)*sin(the3)*sin(the5) + 2*m6*x6*z6*cos(the2)*cos(the4)^2*sin(the3)*sin(the5)*sin(the6) + 2*m6*x6*z6*cos(the3)*cos(the4)^2*sin(the2)*sin(the5)*sin(the6) + 2*m6*x6*z6*cos(the5)^2*cos(the6)*sin(the2)*sin(the3)*sin(the4) - m6*x6^2*cos(the2)*cos(the4)*cos(the5)^2*cos(the6)^2*sin(the3)*sin(the4) - m6*x6^2*cos(the3)*cos(the4)*cos(the5)^2*cos(the6)^2*sin(the2)*sin(the4) + m6*y6^2*cos(the2)*cos(the4)*cos(the5)^2*cos(the6)^2*sin(the3)*sin(the4) + m6*y6^2*cos(the3)*cos(the4)*cos(the5)^2*cos(the6)^2*sin(the2)*sin(the4) - 2*m6*y6*z6*cos(the5)^2*sin(the2)*sin(the3)*sin(the4)*sin(the6) + 2*IPx6*cos(the2)*cos(the3)*cos(the5)*cos(the6)*sin(the4)*sin(the5)*sin(the6) + 2*IPz6*cos(the2)*cos(the4)*cos(the5)*cos(the6)*sin(the3)*sin(the4)*sin(the5) + 2*IPz6*cos(the3)*cos(the4)*cos(the5)*cos(the6)*sin(the2)*sin(the4)*sin(the5) - 4*m6*x6*y6*cos(the2)*cos(the4)^2*cos(the5)*cos(the6)^2*sin(the3) - 4*m6*x6*y6*cos(the3)*cos(the4)^2*cos(the5)*cos(the6)^2*sin(the2) - 2*IPy6*cos(the2)*cos(the4)*cos(the5)*sin(the3)*sin(the4)*sin(the5)*sin(the6) - 2*IPy6*cos(the3)*cos(the4)*cos(the5)*sin(the2)*sin(the4)*sin(the5)*sin(the6) - m6*x6^2*cos(the2)*cos(the3)*cos(the4)*cos(the6)*sin(the5)*sin(the6) + m6*y6^2*cos(the2)*cos(the3)*cos(the4)*cos(the6)*sin(the5)*sin(the6) - 2*IPx6*cos(the5)*cos(the6)*sin(the2)*sin(the3)*sin(the4)*sin(the5)*sin(the6) - d4*m6*x6*cos(the2)*cos(the3)*cos(the5)*cos(the6)*sin(the4) + m6*x6^2*cos(the4)*cos(the6)*sin(the2)*sin(the3)*sin(the5)*sin(the6) - m6*y6^2*cos(the4)*cos(the6)*sin(the2)*sin(the3)*sin(the5)*sin(the6) - m6*y6*z6*cos(the2)*cos(the3)*cos(the4)*cos(the5)*cos(the6) - a3*m6*x6*cos(the2)*cos(the5)*cos(the6)*sin(the3)*sin(the4) - a3*m6*x6*cos(the3)*cos(the5)*cos(the6)*sin(the2)*sin(the4) + 2*m5*x5*y5*cos(the2)*cos(the4)*cos(the5)*sin(the3)*sin(the4)*sin(the5) + 2*m5*x5*y5*cos(the3)*cos(the4)*cos(the5)*sin(the2)*sin(the4)*sin(the5) + 2*m6*x6*y6*cos(the2)*cos(the4)*cos(the6)*sin(the3)*sin(the4)*sin(the6) + 2*m6*x6*y6*cos(the3)*cos(the4)*cos(the6)*sin(the2)*sin(the4)*sin(the6) + 2*m6*x6*y6*cos(the2)*cos(the4)*cos(the5)^2*cos(the6)*sin(the3)*sin(the4)*sin(the6) + 2*m6*x6*y6*cos(the3)*cos(the4)*cos(the5)^2*cos(the6)*sin(the2)*sin(the4)*sin(the6) + 2*m6*x6*y6*cos(the2)*cos(the3)*cos(the5)*cos(the6)*sin(the4)*sin(the5)*sin(the6) + 2*m6*x6*z6*cos(the2)*cos(the4)*cos(the5)*cos(the6)*sin(the3)*sin(the4)*sin(the5) + 2*m6*x6*z6*cos(the3)*cos(the4)*cos(the5)*cos(the6)*sin(the2)*sin(the4)*sin(the5) - 2*m6*y6*z6*cos(the2)*cos(the4)*cos(the5)*sin(the3)*sin(the4)*sin(the5)*sin(the6) - 2*m6*y6*z6*cos(the3)*cos(the4)*cos(the5)*sin(the2)*sin(the4)*sin(the5)*sin(the6) - 2*m6*x6*y6*cos(the5)*cos(the6)*sin(the2)*sin(the3)*sin(the4)*sin(the5)*sin(the6),IPy3*cos(the2)*cos(the3) + IPx4*cos(the2)*sin(the3) + IPx4*cos(the3)*sin(the2) + IPz3*cos(the2)*sin(the3) + IPz3*cos(the3)*sin(the2) - IPy3*sin(the2)*sin(the3) - IPy4*cos(the2)*cos(the3)*cos(the4) + IPx5*cos(the2)*cos(the3)*sin(the4) - IPx6*cos(the2)*cos(the5)*sin(the3) - IPx6*cos(the3)*cos(the5)*sin(the2) - IPz4*cos(the2)*cos(the3)*sin(the4) - IPz5*cos(the2)*cos(the5)*sin(the3) - IPz5*cos(the3)*cos(the5)*sin(the2) + IPy4*cos(the4)*sin(the2)*sin(the3) + IPy5*cos(the2)*sin(the3)*sin(the5) + IPy5*cos(the3)*sin(the2)*sin(the5) - IPx5*sin(the2)*sin(the3)*sin(the4) + IPz4*sin(the2)*sin(the3)*sin(the4) - 2*IPx4*cos(the2)*cos(the4)^2*sin(the3) - 2*IPx4*cos(the3)*cos(the4)^2*sin(the2) + IPy5*cos(the2)*cos(the3)*cos(the4)*cos(the5) + IPx6*cos(the2)*cos(the3)*cos(the4)*sin(the5) + IPz5*cos(the2)*cos(the3)*cos(the4)*sin(the5) + IPz6*cos(the2)*cos(the3)*cos(the6)*sin(the4) - IPy5*cos(the4)*cos(the5)*sin(the2)*sin(the3) - IPy6*cos(the2)*cos(the3)*sin(the4)*sin(the6) - IPy6*cos(the2)*cos(the6)*sin(the3)*sin(the5) - IPy6*cos(the3)*cos(the6)*sin(the2)*sin(the5) + Ixx4*cos(the2)*cos(the4)*sin(the3)*sin(the4) + Ixx4*cos(the3)*cos(the4)*sin(the2)*sin(the4) - Ixx6*cos(the2)*cos(the4)*sin(the3)*sin(the4) - Ixx6*cos(the3)*cos(the4)*sin(the2)*sin(the4) - Iyy4*cos(the2)*cos(the4)*sin(the3)*sin(the4) - Iyy4*cos(the3)*cos(the4)*sin(the2)*sin(the4) + Iyy5*cos(the2)*cos(the4)*sin(the3)*sin(the4) + Iyy5*cos(the3)*cos(the4)*sin(the2)*sin(the4) - Izz5*cos(the2)*cos(the4)*sin(the3)*sin(the4) - Izz5*cos(the3)*cos(the4)*sin(the2)*sin(the4) + Izz6*cos(the2)*cos(the4)*sin(the3)*sin(the4) + Izz6*cos(the3)*cos(the4)*sin(the2)*sin(the4) - IPx6*cos(the4)*sin(the2)*sin(the3)*sin(the5) - IPz5*cos(the4)*sin(the2)*sin(the3)*sin(the5) - IPz6*cos(the6)*sin(the2)*sin(the3)*sin(the4) - IPz6*cos(the2)*sin(the3)*sin(the5)*sin(the6) - IPz6*cos(the3)*sin(the2)*sin(the5)*sin(the6) + IPy6*sin(the2)*sin(the3)*sin(the4)*sin(the6) + m3*y3*z3*cos(the2)*cos(the3) - 2*IPx5*cos(the2)*cos(the3)*cos(the5)^2*sin(the4) + 2*IPx6*cos(the2)*cos(the4)^2*cos(the5)*sin(the3) + 2*IPx6*cos(the3)*cos(the4)^2*cos(the5)*sin(the2) + 2*IPx6*cos(the2)*cos(the5)*cos(the6)^2*sin(the3) + 2*IPx6*cos(the3)*cos(the5)*cos(the6)^2*sin(the2) + 2*IPz5*cos(the2)*cos(the4)^2*cos(the5)*sin(the3) + 2*IPz5*cos(the3)*cos(the4)^2*cos(the5)*sin(the2) + m4*x4*y4*cos(the2)*sin(the3) + m4*x4*y4*cos(the3)*sin(the2) + m3*x3*z3*cos(the2)*sin(the3) + m3*x3*z3*cos(the3)*sin(the2) - 2*IPy5*cos(the2)*cos(the4)^2*sin(the3)*sin(the5) - 2*IPy5*cos(the3)*cos(the4)^2*sin(the2)*sin(the5) - m3*y3*z3*sin(the2)*sin(the3) + 2*IPx5*cos(the5)^2*sin(the2)*sin(the3)*sin(the4) + Ixx5*cos(the2)*cos(the3)*cos(the5)*sin(the4)*sin(the5) - Ixx6*cos(the2)*cos(the5)*cos(the6)*sin(the3)*sin(the6) - Ixx6*cos(the3)*cos(the5)*cos(the6)*sin(the2)*sin(the6) - Iyy5*cos(the2)*cos(the3)*cos(the5)*sin(the4)*sin(the5) + Iyy6*cos(the2)*cos(the3)*cos(the5)*sin(the4)*sin(the5) + Iyy6*cos(the2)*cos(the5)*cos(the6)*sin(the3)*sin(the6) + Iyy6*cos(the3)*cos(the5)*cos(the6)*sin(the2)*sin(the6) - Izz6*cos(the2)*cos(the3)*cos(the5)*sin(the4)*sin(the5) + IPz6*cos(the4)*cos(the5)*sin(the2)*sin(the3)*sin(the6) - Ixx5*cos(the5)*sin(the2)*sin(the3)*sin(the4)*sin(the5) + Iyy5*cos(the5)*sin(the2)*sin(the3)*sin(the4)*sin(the5) - Iyy6*cos(the5)*sin(the2)*sin(the3)*sin(the4)*sin(the5) + Izz6*cos(the5)*sin(the2)*sin(the3)*sin(the4)*sin(the5) - m4*x4^2*cos(the2)*cos(the4)*sin(the3)*sin(the4) - m4*x4^2*cos(the3)*cos(the4)*sin(the2)*sin(the4) + m6*x6^2*cos(the2)*cos(the4)*sin(the3)*sin(the4) + m6*x6^2*cos(the3)*cos(the4)*sin(the2)*sin(the4) + m4*y4^2*cos(the2)*cos(the4)*sin(the3)*sin(the4) + m4*y4^2*cos(the3)*cos(the4)*sin(the2)*sin(the4) - m5*y5^2*cos(the2)*cos(the4)*sin(the3)*sin(the4) - m5*y5^2*cos(the3)*cos(the4)*sin(the2)*sin(the4) + m5*z5^2*cos(the2)*cos(the4)*sin(the3)*sin(the4) + m5*z5^2*cos(the3)*cos(the4)*sin(the2)*sin(the4) - m6*z6^2*cos(the2)*cos(the4)*sin(the3)*sin(the4) - m6*z6^2*cos(the3)*cos(the4)*sin(the2)*sin(the4) - d4*m4*y4*cos(the2)*cos(the3)*cos(the4) + d4*m5*z5*cos(the2)*cos(the3)*cos(the4) - a3*m4*y4*cos(the2)*cos(the4)*sin(the3) - a3*m4*y4*cos(the3)*cos(the4)*sin(the2) + a3*m5*z5*cos(the2)*cos(the4)*sin(the3) + a3*m5*z5*cos(the3)*cos(the4)*sin(the2) - d4*m4*x4*cos(the2)*cos(the3)*sin(the4) - m4*y4*z4*cos(the2)*cos(the3)*cos(the4) - a3*m4*x4*cos(the2)*sin(the3)*sin(the4) - a3*m4*x4*cos(the3)*sin(the2)*sin(the4) - 2*IPx6*cos(the2)*cos(the3)*cos(the4)*cos(the6)^2*sin(the5) - 2*IPz6*cos(the2)*cos(the3)*cos(the5)^2*cos(the6)*sin(the4) + d4*m4*y4*cos(the4)*sin(the2)*sin(the3) - d4*m5*z5*cos(the4)*sin(the2)*sin(the3) + m5*x5*y5*cos(the2)*cos(the3)*sin(the4) - m6*x6*y6*cos(the2)*cos(the5)*sin(the3) - m6*x6*y6*cos(the3)*cos(the5)*sin(the2) - m4*x4*z4*cos(the2)*cos(the3)*sin(the4) - m5*x5*z5*cos(the2)*cos(the5)*sin(the3) - m5*x5*z5*cos(the3)*cos(the5)*sin(the2) + 2*IPy6*cos(the2)*cos(the3)*cos(the5)^2*sin(the4)*sin(the6) + 2*IPy6*cos(the2)*cos(the4)^2*cos(the6)*sin(the3)*sin(the5) + 2*IPy6*cos(the3)*cos(the4)^2*cos(the6)*sin(the2)*sin(the5) + Ixx5*cos(the2)*cos(the4)*cos(the5)^2*sin(the3)*sin(the4) + Ixx5*cos(the3)*cos(the4)*cos(the5)^2*sin(the2)*sin(the4) + Ixx6*cos(the2)*cos(the4)*cos(the6)^2*sin(the3)*sin(the4) + Ixx6*cos(the3)*cos(the4)*cos(the6)^2*sin(the2)*sin(the4) - Iyy5*cos(the2)*cos(the4)*cos(the5)^2*sin(the3)*sin(the4) - Iyy5*cos(the3)*cos(the4)*cos(the5)^2*sin(the2)*sin(the4) + Iyy6*cos(the2)*cos(the4)*cos(the5)^2*sin(the3)*sin(the4) + Iyy6*cos(the3)*cos(the4)*cos(the5)^2*sin(the2)*sin(the4) - Iyy6*cos(the2)*cos(the4)*cos(the6)^2*sin(the3)*sin(the4) - Iyy6*cos(the3)*cos(the4)*cos(the6)^2*sin(the2)*sin(the4) - Izz6*cos(the2)*cos(the4)*cos(the5)^2*sin(the3)*sin(the4) - Izz6*cos(the3)*cos(the4)*cos(the5)^2*sin(the2)*sin(the4) + d4*m4*x4*sin(the2)*sin(the3)*sin(the4) + m4*y4*z4*cos(the4)*sin(the2)*sin(the3) + m5*y5*z5*cos(the2)*sin(the3)*sin(the5) + m5*y5*z5*cos(the3)*sin(the2)*sin(the5) + 2*IPx6*cos(the4)*cos(the6)^2*sin(the2)*sin(the3)*sin(the5) + 2*IPz6*cos(the2)*cos(the4)^2*sin(the3)*sin(the5)*sin(the6) + 2*IPz6*cos(the3)*cos(the4)^2*sin(the2)*sin(the5)*sin(the6) + 2*IPz6*cos(the5)^2*cos(the6)*sin(the2)*sin(the3)*sin(the4) - m5*x5*y5*sin(the2)*sin(the3)*sin(the4) + m4*x4*z4*sin(the2)*sin(the3)*sin(the4) - 2*IPy6*cos(the5)^2*sin(the2)*sin(the3)*sin(the4)*sin(the6) - 4*IPx6*cos(the2)*cos(the4)^2*cos(the5)*cos(the6)^2*sin(the3) - 4*IPx6*cos(the3)*cos(the4)^2*cos(the5)*cos(the6)^2*sin(the2) - 2*m4*x4*y4*cos(the2)*cos(the4)^2*sin(the3) - 2*m4*x4*y4*cos(the3)*cos(the4)^2*sin(the2) - IPy6*cos(the2)*cos(the3)*cos(the4)*cos(the5)*cos(the6) - IPz6*cos(the2)*cos(the3)*cos(the4)*cos(the5)*sin(the6) + IPy6*cos(the4)*cos(the5)*cos(the6)*sin(the2)*sin(the3) - d4*m6*y6*cos(the2)*cos(the3)*cos(the4)*cos(the6) - a3*m6*y6*cos(the2)*cos(the4)*cos(the6)*sin(the3) - a3*m6*y6*cos(the3)*cos(the4)*cos(the6)*sin(the2) - d4*m5*x5*cos(the2)*cos(the3)*cos(the5)*sin(the4) - d4*m6*x6*cos(the2)*cos(the3)*cos(the4)*sin(the6) + m5*x5^2*cos(the5)*sin(the2)*sin(the3)*sin(the4)*sin(the5) - m5*y5^2*cos(the5)*sin(the2)*sin(the3)*sin(the4)*sin(the5) + m6*y6^2*cos(the5)*sin(the2)*sin(the3)*sin(the4)*sin(the5) - m6*z6^2*cos(the5)*sin(the2)*sin(the3)*sin(the4)*sin(the5) + m5*y5*z5*cos(the2)*cos(the3)*cos(the4)*cos(the5) - a3*m5*x5*cos(the2)*cos(the5)*sin(the3)*sin(the4) - a3*m5*x5*cos(the3)*cos(the5)*sin(the2)*sin(the4) - a3*m6*x6*cos(the2)*cos(the4)*sin(the3)*sin(the6) - a3*m6*x6*cos(the3)*cos(the4)*sin(the2)*sin(the6) + d4*m5*y5*cos(the2)*cos(the3)*sin(the4)*sin(the5) + d4*m6*y6*cos(the4)*cos(the6)*sin(the2)*sin(the3) + d4*m6*z6*cos(the2)*cos(the3)*sin(the4)*sin(the5) + m6*x6*y6*cos(the2)*cos(the3)*cos(the4)*sin(the5) + m5*x5*z5*cos(the2)*cos(the3)*cos(the4)*sin(the5) + m6*x6*z6*cos(the2)*cos(the3)*cos(the6)*sin(the4) + a3*m5*y5*cos(the2)*sin(the3)*sin(the4)*sin(the5) + a3*m5*y5*cos(the3)*sin(the2)*sin(the4)*sin(the5) + a3*m6*z6*cos(the2)*sin(the3)*sin(the4)*sin(the5) + a3*m6*z6*cos(the3)*sin(the2)*sin(the4)*sin(the5) + Ixx6*cos(the2)*cos(the3)*cos(the5)*cos(the6)^2*sin(the4)*sin(the5) + 2*Ixx6*cos(the2)*cos(the4)^2*cos(the5)*cos(the6)*sin(the3)*sin(the6) + 2*Ixx6*cos(the3)*cos(the4)^2*cos(the5)*cos(the6)*sin(the2)*sin(the6) - Iyy6*cos(the2)*cos(the3)*cos(the5)*cos(the6)^2*sin(the4)*sin(the5) - 2*Iyy6*cos(the2)*cos(the4)^2*cos(the5)*cos(the6)*sin(the3)*sin(the6) - 2*Iyy6*cos(the3)*cos(the4)^2*cos(the5)*cos(the6)*sin(the2)*sin(the6) + d4*m5*x5*cos(the5)*sin(the2)*sin(the3)*sin(the4) + d4*m6*x6*cos(the4)*sin(the2)*sin(the3)*sin(the6) - m5*y5*z5*cos(the4)*cos(the5)*sin(the2)*sin(the3) - m6*y6*z6*cos(the2)*cos(the3)*sin(the4)*sin(the6) - m6*y6*z6*cos(the2)*cos(the6)*sin(the3)*sin(the5) - m6*y6*z6*cos(the3)*cos(the6)*sin(the2)*sin(the5) - d4*m5*y5*sin(the2)*sin(the3)*sin(the4)*sin(the5) - d4*m6*z6*sin(the2)*sin(the3)*sin(the4)*sin(the5) - m6*x6*y6*cos(the4)*sin(the2)*sin(the3)*sin(the5) - m5*x5*z5*cos(the4)*sin(the2)*sin(the3)*sin(the5) - m6*x6*z6*cos(the6)*sin(the2)*sin(the3)*sin(the4) - m6*x6*z6*cos(the2)*sin(the3)*sin(the5)*sin(the6) - m6*x6*z6*cos(the3)*sin(the2)*sin(the5)*sin(the6) - Ixx6*cos(the5)*cos(the6)^2*sin(the2)*sin(the3)*sin(the4)*sin(the5) + Iyy6*cos(the5)*cos(the6)^2*sin(the2)*sin(the3)*sin(the4)*sin(the5) - m5*x5^2*cos(the2)*cos(the4)*cos(the5)^2*sin(the3)*sin(the4) - m5*x5^2*cos(the3)*cos(the4)*cos(the5)^2*sin(the2)*sin(the4) - m6*x6^2*cos(the2)*cos(the4)*cos(the6)^2*sin(the3)*sin(the4) - m6*x6^2*cos(the3)*cos(the4)*cos(the6)^2*sin(the2)*sin(the4) + m5*y5^2*cos(the2)*cos(the4)*cos(the5)^2*sin(the3)*sin(the4) + m5*y5^2*cos(the3)*cos(the4)*cos(the5)^2*sin(the2)*sin(the4) - m6*y6^2*cos(the2)*cos(the4)*cos(the5)^2*sin(the3)*sin(the4) - m6*y6^2*cos(the3)*cos(the4)*cos(the5)^2*sin(the2)*sin(the4) + m6*y6^2*cos(the2)*cos(the4)*cos(the6)^2*sin(the3)*sin(the4) + m6*y6^2*cos(the3)*cos(the4)*cos(the6)^2*sin(the2)*sin(the4) + m6*z6^2*cos(the2)*cos(the4)*cos(the5)^2*sin(the3)*sin(the4) + m6*z6^2*cos(the3)*cos(the4)*cos(the5)^2*sin(the2)*sin(the4) + m6*y6*z6*sin(the2)*sin(the3)*sin(the4)*sin(the6) - 2*m5*x5*y5*cos(the2)*cos(the3)*cos(the5)^2*sin(the4) + 2*m6*x6*y6*cos(the2)*cos(the4)^2*cos(the5)*sin(the3) + 2*m6*x6*y6*cos(the3)*cos(the4)^2*cos(the5)*sin(the2) + 2*m6*x6*y6*cos(the2)*cos(the5)*cos(the6)^2*sin(the3) + 2*m6*x6*y6*cos(the3)*cos(the5)*cos(the6)^2*sin(the2) + 2*m5*x5*z5*cos(the2)*cos(the4)^2*cos(the5)*sin(the3) + 2*m5*x5*z5*cos(the3)*cos(the4)^2*cos(the5)*sin(the2) + Ixx6*cos(the2)*cos(the4)*cos(the5)^2*cos(the6)^2*sin(the3)*sin(the4) + Ixx6*cos(the3)*cos(the4)*cos(the5)^2*cos(the6)^2*sin(the2)*sin(the4) - Iyy6*cos(the2)*cos(the4)*cos(the5)^2*cos(the6)^2*sin(the3)*sin(the4) - Iyy6*cos(the3)*cos(the4)*cos(the5)^2*cos(the6)^2*sin(the2)*sin(the4) - 2*m5*y5*z5*cos(the2)*cos(the4)^2*sin(the3)*sin(the5) - 2*m5*y5*z5*cos(the3)*cos(the4)^2*sin(the2)*sin(the5) + 2*m5*x5*y5*cos(the5)^2*sin(the2)*sin(the3)*sin(the4) + Ixx6*cos(the2)*cos(the3)*cos(the4)*cos(the6)*sin(the5)*sin(the6) - Iyy6*cos(the2)*cos(the3)*cos(the4)*cos(the6)*sin(the5)*sin(the6) + 2*IPx5*cos(the2)*cos(the4)*cos(the5)*sin(the3)*sin(the4)*sin(the5) + 2*IPx5*cos(the3)*cos(the4)*cos(the5)*sin(the2)*sin(the4)*sin(the5) + 2*IPx6*cos(the2)*cos(the4)*cos(the6)*sin(the3)*sin(the4)*sin(the6) + 2*IPx6*cos(the3)*cos(the4)*cos(the6)*sin(the2)*sin(the4)*sin(the6) - Ixx6*cos(the4)*cos(the6)*sin(the2)*sin(the3)*sin(the5)*sin(the6) + Iyy6*cos(the4)*cos(the6)*sin(the2)*sin(the3)*sin(the5)*sin(the6) - m5*x5^2*cos(the2)*cos(the3)*cos(the5)*sin(the4)*sin(the5) + m6*x6^2*cos(the2)*cos(the5)*cos(the6)*sin(the3)*sin(the6) + m6*x6^2*cos(the3)*cos(the5)*cos(the6)*sin(the2)*sin(the6) + m5*y5^2*cos(the2)*cos(the3)*cos(the5)*sin(the4)*sin(the5) - m6*y6^2*cos(the2)*cos(the3)*cos(the5)*sin(the4)*sin(the5) - m6*y6^2*cos(the2)*cos(the5)*cos(the6)*sin(the3)*sin(the6) - m6*y6^2*cos(the3)*cos(the5)*cos(the6)*sin(the2)*sin(the6) + m6*z6^2*cos(the2)*cos(the3)*cos(the5)*sin(the4)*sin(the5) + d4*m6*y6*cos(the2)*cos(the3)*cos(the5)*sin(the4)*sin(the6) - m6*x6*z6*cos(the2)*cos(the3)*cos(the4)*cos(the5)*sin(the6) + a3*m6*y6*cos(the2)*cos(the5)*sin(the3)*sin(the4)*sin(the6) + a3*m6*y6*cos(the3)*cos(the5)*sin(the2)*sin(the4)*sin(the6) + d4*m6*x6*cos(the5)*cos(the6)*sin(the2)*sin(the3)*sin(the4) + m6*y6*z6*cos(the4)*cos(the5)*cos(the6)*sin(the2)*sin(the3) + 2*IPx6*cos(the2)*cos(the4)*cos(the5)^2*cos(the6)*sin(the3)*sin(the4)*sin(the6) + 2*IPx6*cos(the3)*cos(the4)*cos(the5)^2*cos(the6)*sin(the2)*sin(the4)*sin(the6) - d4*m6*y6*cos(the5)*sin(the2)*sin(the3)*sin(the4)*sin(the6) + m6*x6*z6*cos(the4)*cos(the5)*sin(the2)*sin(the3)*sin(the6) - m6*x6^2*cos(the2)*cos(the3)*cos(the5)*cos(the6)^2*sin(the4)*sin(the5) - 2*m6*x6^2*cos(the2)*cos(the4)^2*cos(the5)*cos(the6)*sin(the3)*sin(the6) - 2*m6*x6^2*cos(the3)*cos(the4)^2*cos(the5)*cos(the6)*sin(the2)*sin(the6) + m6*y6^2*cos(the2)*cos(the3)*cos(the5)*cos(the6)^2*sin(the4)*sin(the5) + 2*m6*y6^2*cos(the2)*cos(the4)^2*cos(the5)*cos(the6)*sin(the3)*sin(the6) + 2*m6*y6^2*cos(the3)*cos(the4)^2*cos(the5)*cos(the6)*sin(the2)*sin(the6) + m6*x6^2*cos(the5)*cos(the6)^2*sin(the2)*sin(the3)*sin(the4)*sin(the5) - m6*y6^2*cos(the5)*cos(the6)^2*sin(the2)*sin(the3)*sin(the4)*sin(the5) - 2*m6*x6*y6*cos(the2)*cos(the3)*cos(the4)*cos(the6)^2*sin(the5) - 2*m6*x6*z6*cos(the2)*cos(the3)*cos(the5)^2*cos(the6)*sin(the4) + 2*m6*y6*z6*cos(the2)*cos(the3)*cos(the5)^2*sin(the4)*sin(the6) + 2*m6*y6*z6*cos(the2)*cos(the4)^2*cos(the6)*sin(the3)*sin(the5) + 2*m6*y6*z6*cos(the3)*cos(the4)^2*cos(the6)*sin(the2)*sin(the5) + 2*m6*x6*y6*cos(the4)*cos(the6)^2*sin(the2)*sin(the3)*sin(the5) + 2*m6*x6*z6*cos(the2)*cos(the4)^2*sin(the3)*sin(the5)*sin(the6) + 2*m6*x6*z6*cos(the3)*cos(the4)^2*sin(the2)*sin(the5)*sin(the6) + 2*m6*x6*z6*cos(the5)^2*cos(the6)*sin(the2)*sin(the3)*sin(the4) - m6*x6^2*cos(the2)*cos(the4)*cos(the5)^2*cos(the6)^2*sin(the3)*sin(the4) - m6*x6^2*cos(the3)*cos(the4)*cos(the5)^2*cos(the6)^2*sin(the2)*sin(the4) + m6*y6^2*cos(the2)*cos(the4)*cos(the5)^2*cos(the6)^2*sin(the3)*sin(the4) + m6*y6^2*cos(the3)*cos(the4)*cos(the5)^2*cos(the6)^2*sin(the2)*sin(the4) - 2*m6*y6*z6*cos(the5)^2*sin(the2)*sin(the3)*sin(the4)*sin(the6) + 2*IPx6*cos(the2)*cos(the3)*cos(the5)*cos(the6)*sin(the4)*sin(the5)*sin(the6) + 2*IPz6*cos(the2)*cos(the4)*cos(the5)*cos(the6)*sin(the3)*sin(the4)*sin(the5) + 2*IPz6*cos(the3)*cos(the4)*cos(the5)*cos(the6)*sin(the2)*sin(the4)*sin(the5) - 4*m6*x6*y6*cos(the2)*cos(the4)^2*cos(the5)*cos(the6)^2*sin(the3) - 4*m6*x6*y6*cos(the3)*cos(the4)^2*cos(the5)*cos(the6)^2*sin(the2) - 2*IPy6*cos(the2)*cos(the4)*cos(the5)*sin(the3)*sin(the4)*sin(the5)*sin(the6) - 2*IPy6*cos(the3)*cos(the4)*cos(the5)*sin(the2)*sin(the4)*sin(the5)*sin(the6) - m6*x6^2*cos(the2)*cos(the3)*cos(the4)*cos(the6)*sin(the5)*sin(the6) + m6*y6^2*cos(the2)*cos(the3)*cos(the4)*cos(the6)*sin(the5)*sin(the6) - 2*IPx6*cos(the5)*cos(the6)*sin(the2)*sin(the3)*sin(the4)*sin(the5)*sin(the6) - d4*m6*x6*cos(the2)*cos(the3)*cos(the5)*cos(the6)*sin(the4) + m6*x6^2*cos(the4)*cos(the6)*sin(the2)*sin(the3)*sin(the5)*sin(the6) - m6*y6^2*cos(the4)*cos(the6)*sin(the2)*sin(the3)*sin(the5)*sin(the6) - m6*y6*z6*cos(the2)*cos(the3)*cos(the4)*cos(the5)*cos(the6) - a3*m6*x6*cos(the2)*cos(the5)*cos(the6)*sin(the3)*sin(the4) - a3*m6*x6*cos(the3)*cos(the5)*cos(the6)*sin(the2)*sin(the4) + 2*m5*x5*y5*cos(the2)*cos(the4)*cos(the5)*sin(the3)*sin(the4)*sin(the5) + 2*m5*x5*y5*cos(the3)*cos(the4)*cos(the5)*sin(the2)*sin(the4)*sin(the5) + 2*m6*x6*y6*cos(the2)*cos(the4)*cos(the6)*sin(the3)*sin(the4)*sin(the6) + 2*m6*x6*y6*cos(the3)*cos(the4)*cos(the6)*sin(the2)*sin(the4)*sin(the6) + 2*m6*x6*y6*cos(the2)*cos(the4)*cos(the5)^2*cos(the6)*sin(the3)*sin(the4)*sin(the6) + 2*m6*x6*y6*cos(the3)*cos(the4)*cos(the5)^2*cos(the6)*sin(the2)*sin(the4)*sin(the6) + 2*m6*x6*y6*cos(the2)*cos(the3)*cos(the5)*cos(the6)*sin(the4)*sin(the5)*sin(the6) + 2*m6*x6*z6*cos(the2)*cos(the4)*cos(the5)*cos(the6)*sin(the3)*sin(the4)*sin(the5) + 2*m6*x6*z6*cos(the3)*cos(the4)*cos(the5)*cos(the6)*sin(the2)*sin(the4)*sin(the5) - 2*m6*y6*z6*cos(the2)*cos(the4)*cos(the5)*sin(the3)*sin(the4)*sin(the5)*sin(the6) - 2*m6*y6*z6*cos(the3)*cos(the4)*cos(the5)*sin(the2)*sin(the4)*sin(the5)*sin(the6) - 2*m6*x6*y6*cos(the5)*cos(the6)*sin(the2)*sin(the3)*sin(the4)*sin(the5)*sin(the6),Ixx5*sin(the2)*sin(the3) - Iyy6*cos(the2)*cos(the3) - Izz4*cos(the2)*cos(the3) - Ixx5*cos(the2)*cos(the3) + Iyy6*sin(the2)*sin(the3) + Izz4*sin(the2)*sin(the3) - IPx5*cos(the2)*cos(the4)*sin(the3) - IPx5*cos(the3)*cos(the4)*sin(the2) + IPz4*cos(the2)*cos(the4)*sin(the3) + IPz4*cos(the3)*cos(the4)*sin(the2) - IPy4*cos(the2)*sin(the3)*sin(the4) - IPy4*cos(the3)*sin(the2)*sin(the4) - m4*x4^2*cos(the2)*cos(the3) - m6*x6^2*cos(the2)*cos(the3) - m4*y4^2*cos(the2)*cos(the3) - m5*y5^2*cos(the2)*cos(the3) - m5*z5^2*cos(the2)*cos(the3) - m6*z6^2*cos(the2)*cos(the3) + m4*x4^2*sin(the2)*sin(the3) + m6*x6^2*sin(the2)*sin(the3) + m4*y4^2*sin(the2)*sin(the3) + m5*y5^2*sin(the2)*sin(the3) + m5*z5^2*sin(the2)*sin(the3) + m6*z6^2*sin(the2)*sin(the3) - a1*m4*x4*cos(the4) + a1*m4*y4*sin(the4) - a1*m5*z5*sin(the4) + Ixx5*cos(the2)*cos(the3)*cos(the5)^2 - Ixx6*cos(the2)*cos(the3)*cos(the6)^2 - Iyy5*cos(the2)*cos(the3)*cos(the5)^2 + Iyy6*cos(the2)*cos(the3)*cos(the5)^2 + Iyy6*cos(the2)*cos(the3)*cos(the6)^2 - Izz6*cos(the2)*cos(the3)*cos(the5)^2 - Ixx5*cos(the5)^2*sin(the2)*sin(the3) + Ixx6*cos(the6)^2*sin(the2)*sin(the3) + Iyy5*cos(the5)^2*sin(the2)*sin(the3) - Iyy6*cos(the5)^2*sin(the2)*sin(the3) - Iyy6*cos(the6)^2*sin(the2)*sin(the3) + Izz6*cos(the5)^2*sin(the2)*sin(the3) + 2*IPx5*cos(the2)*cos(the3)*cos(the5)*sin(the5) - 2*IPx6*cos(the2)*cos(the3)*cos(the6)*sin(the6) - IPz6*cos(the2)*cos(the4)*cos(the6)*sin(the3) - IPz6*cos(the3)*cos(the4)*cos(the6)*sin(the2) + IPy5*cos(the2)*cos(the5)*sin(the3)*sin(the4) + IPy5*cos(the3)*cos(the5)*sin(the2)*sin(the4) + IPy6*cos(the2)*cos(the4)*sin(the3)*sin(the6) + IPy6*cos(the3)*cos(the4)*sin(the2)*sin(the6) - 2*IPx5*cos(the5)*sin(the2)*sin(the3)*sin(the5) + IPx6*cos(the2)*sin(the3)*sin(the4)*sin(the5) + IPx6*cos(the3)*sin(the2)*sin(the4)*sin(the5) + 2*IPx6*cos(the6)*sin(the2)*sin(the3)*sin(the6) + IPz5*cos(the2)*sin(the3)*sin(the4)*sin(the5) + IPz5*cos(the3)*sin(the2)*sin(the4)*sin(the5) - a2*m4*x4*cos(the2)*cos(the4) - a1*m5*x5*cos(the4)*cos(the5) + a2*m4*y4*cos(the2)*sin(the4) + a1*m5*y5*cos(the4)*sin(the5) + a1*m6*y6*cos(the6)*sin(the4) - a2*m5*z5*cos(the2)*sin(the4) + a1*m6*z6*cos(the4)*sin(the5) + a1*m6*x6*sin(the4)*sin(the6) + 2*IPx5*cos(the2)*cos(the4)*cos(the5)^2*sin(the3) + 2*IPx5*cos(the3)*cos(the4)*cos(the5)^2*sin(the2) - m5*x5^2*cos(the2)*cos(the3)*cos(the5)^2 + m6*x6^2*cos(the2)*cos(the3)*cos(the6)^2 + m5*y5^2*cos(the2)*cos(the3)*cos(the5)^2 - m6*y6^2*cos(the2)*cos(the3)*cos(the5)^2 - m6*y6^2*cos(the2)*cos(the3)*cos(the6)^2 + m6*z6^2*cos(the2)*cos(the3)*cos(the5)^2 + m5*x5^2*cos(the5)^2*sin(the2)*sin(the3) - m6*x6^2*cos(the6)^2*sin(the2)*sin(the3) - m5*y5^2*cos(the5)^2*sin(the2)*sin(the3) + m6*y6^2*cos(the5)^2*sin(the2)*sin(the3) + m6*y6^2*cos(the6)^2*sin(the2)*sin(the3) - m6*z6^2*cos(the5)^2*sin(the2)*sin(the3) + Ixx6*cos(the2)*cos(the3)*cos(the5)^2*cos(the6)^2 - Iyy6*cos(the2)*cos(the3)*cos(the5)^2*cos(the6)^2 - Ixx6*cos(the5)^2*cos(the6)^2*sin(the2)*sin(the3) + Iyy6*cos(the5)^2*cos(the6)^2*sin(the2)*sin(the3) - Ixx5*cos(the2)*cos(the4)*cos(the5)*sin(the3)*sin(the5) - Ixx5*cos(the3)*cos(the4)*cos(the5)*sin(the2)*sin(the5) + Iyy5*cos(the2)*cos(the4)*cos(the5)*sin(the3)*sin(the5) + Iyy5*cos(the3)*cos(the4)*cos(the5)*sin(the2)*sin(the5) - Iyy6*cos(the2)*cos(the4)*cos(the5)*sin(the3)*sin(the5) - Iyy6*cos(the3)*cos(the4)*cos(the5)*sin(the2)*sin(the5) + Izz6*cos(the2)*cos(the4)*cos(the5)*sin(the3)*sin(the5) + Izz6*cos(the3)*cos(the4)*cos(the5)*sin(the2)*sin(the5) - IPz6*cos(the2)*cos(the5)*sin(the3)*sin(the4)*sin(the6) - IPz6*cos(the3)*cos(the5)*sin(the2)*sin(the4)*sin(the6) - 2*IPz6*cos(the5)*cos(the6)*sin(the2)*sin(the3)*sin(the5) + 2*IPy6*cos(the5)*sin(the2)*sin(the3)*sin(the5)*sin(the6) - a3*m4*x4*cos(the2)*cos(the3)*cos(the4) - a2*m5*x5*cos(the2)*cos(the4)*cos(the5) - a1*m6*x6*cos(the4)*cos(the5)*cos(the6) + a3*m4*y4*cos(the2)*cos(the3)*sin(the4) + a2*m5*y5*cos(the2)*cos(the4)*sin(the5) + a2*m6*y6*cos(the2)*cos(the6)*sin(the4) + a1*m6*y6*cos(the4)*cos(the5)*sin(the6) - a3*m5*z5*cos(the2)*cos(the3)*sin(the4) + a2*m6*z6*cos(the2)*cos(the4)*sin(the5) + d4*m4*x4*cos(the2)*cos(the4)*sin(the3) + d4*m4*x4*cos(the3)*cos(the4)*sin(the2) + a3*m4*x4*cos(the4)*sin(the2)*sin(the3) + a2*m6*x6*cos(the2)*sin(the4)*sin(the6) + 2*IPx6*cos(the2)*cos(the3)*cos(the5)^2*cos(the6)*sin(the6) + 2*IPz6*cos(the2)*cos(the4)*cos(the5)^2*cos(the6)*sin(the3) + 2*IPz6*cos(the3)*cos(the4)*cos(the5)^2*cos(the6)*sin(the2) - d4*m4*y4*cos(the2)*sin(the3)*sin(the4) - d4*m4*y4*cos(the3)*sin(the2)*sin(the4) + d4*m5*z5*cos(the2)*sin(the3)*sin(the4) + d4*m5*z5*cos(the3)*sin(the2)*sin(the4) - m5*x5*y5*cos(the2)*cos(the4)*sin(the3) - m5*x5*y5*cos(the3)*cos(the4)*sin(the2) + m4*x4*z4*cos(the2)*cos(the4)*sin(the3) + m4*x4*z4*cos(the3)*cos(the4)*sin(the2) - a3*m4*y4*sin(the2)*sin(the3)*sin(the4) + a3*m5*z5*sin(the2)*sin(the3)*sin(the4) - 2*IPy6*cos(the2)*cos(the4)*cos(the5)^2*sin(the3)*sin(the6) - 2*IPy6*cos(the3)*cos(the4)*cos(the5)^2*sin(the2)*sin(the6) - m4*y4*z4*cos(the2)*sin(the3)*sin(the4) - m4*y4*z4*cos(the3)*sin(the2)*sin(the4) - 2*IPx6*cos(the2)*cos(the6)^2*sin(the3)*sin(the4)*sin(the5) - 2*IPx6*cos(the3)*cos(the6)^2*sin(the2)*sin(the4)*sin(the5) - 2*IPx6*cos(the5)^2*cos(the6)*sin(the2)*sin(the3)*sin(the6) - m6*x6^2*cos(the2)*cos(the3)*cos(the5)^2*cos(the6)^2 + m6*y6^2*cos(the2)*cos(the3)*cos(the5)^2*cos(the6)^2 + m6*x6^2*cos(the5)^2*cos(the6)^2*sin(the2)*sin(the3) - m6*y6^2*cos(the5)^2*cos(the6)^2*sin(the2)*sin(the3) + 2*IPz6*cos(the2)*cos(the3)*cos(the5)*cos(the6)*sin(the5) - IPy6*cos(the2)*cos(the5)*cos(the6)*sin(the3)*sin(the4) - IPy6*cos(the3)*cos(the5)*cos(the6)*sin(the2)*sin(the4) - 2*IPy6*cos(the2)*cos(the3)*cos(the5)*sin(the5)*sin(the6) - a3*m5*x5*cos(the2)*cos(the3)*cos(the4)*cos(the5) - a2*m6*x6*cos(the2)*cos(the4)*cos(the5)*cos(the6) + a3*m5*y5*cos(the2)*cos(the3)*cos(the4)*sin(the5) + a3*m6*y6*cos(the2)*cos(the3)*cos(the6)*sin(the4) + a2*m6*y6*cos(the2)*cos(the4)*cos(the5)*sin(the6) + a3*m6*z6*cos(the2)*cos(the3)*cos(the4)*sin(the5) + d4*m5*x5*cos(the2)*cos(the4)*cos(the5)*sin(the3) + d4*m5*x5*cos(the3)*cos(the4)*cos(the5)*sin(the2) + a3*m5*x5*cos(the4)*cos(the5)*sin(the2)*sin(the3) + a3*m6*x6*cos(the2)*cos(the3)*sin(the4)*sin(the6) - d4*m5*y5*cos(the2)*cos(the4)*sin(the3)*sin(the5) - d4*m5*y5*cos(the3)*cos(the4)*sin(the2)*sin(the5) - d4*m6*y6*cos(the2)*cos(the6)*sin(the3)*sin(the4) - d4*m6*y6*cos(the3)*cos(the6)*sin(the2)*sin(the4) - d4*m6*z6*cos(the2)*cos(the4)*sin(the3)*sin(the5) - d4*m6*z6*cos(the3)*cos(the4)*sin(the2)*sin(the5) + 2*m5*x5*y5*cos(the2)*cos(the3)*cos(the5)*sin(the5) - 2*m6*x6*y6*cos(the2)*cos(the3)*cos(the6)*sin(the6) - m6*x6*z6*cos(the2)*cos(the4)*cos(the6)*sin(the3) - m6*x6*z6*cos(the3)*cos(the4)*cos(the6)*sin(the2) - a3*m5*y5*cos(the4)*sin(the2)*sin(the3)*sin(the5) - a3*m6*y6*cos(the6)*sin(the2)*sin(the3)*sin(the4) - a3*m6*z6*cos(the4)*sin(the2)*sin(the3)*sin(the5) - Ixx6*cos(the2)*cos(the4)*cos(the5)*cos(the6)^2*sin(the3)*sin(the5) - Ixx6*cos(the3)*cos(the4)*cos(the5)*cos(the6)^2*sin(the2)*sin(the5) + Iyy6*cos(the2)*cos(the4)*cos(the5)*cos(the6)^2*sin(the3)*sin(the5) + Iyy6*cos(the3)*cos(the4)*cos(the5)*cos(the6)^2*sin(the2)*sin(the5) - d4*m6*x6*cos(the2)*sin(the3)*sin(the4)*sin(the6) - d4*m6*x6*cos(the3)*sin(the2)*sin(the4)*sin(the6) + m5*y5*z5*cos(the2)*cos(the5)*sin(the3)*sin(the4) + m5*y5*z5*cos(the3)*cos(the5)*sin(the2)*sin(the4) + m6*y6*z6*cos(the2)*cos(the4)*sin(the3)*sin(the6) + m6*y6*z6*cos(the3)*cos(the4)*sin(the2)*sin(the6) - a3*m6*x6*sin(the2)*sin(the3)*sin(the4)*sin(the6) - 2*m5*x5*y5*cos(the5)*sin(the2)*sin(the3)*sin(the5) + m6*x6*y6*cos(the2)*sin(the3)*sin(the4)*sin(the5) + m6*x6*y6*cos(the3)*sin(the2)*sin(the4)*sin(the5) + 2*m6*x6*y6*cos(the6)*sin(the2)*sin(the3)*sin(the6) + m5*x5*z5*cos(the2)*sin(the3)*sin(the4)*sin(the5) + m5*x5*z5*cos(the3)*sin(the2)*sin(the4)*sin(the5) + 2*m5*x5*y5*cos(the2)*cos(the4)*cos(the5)^2*sin(the3) + 2*m5*x5*y5*cos(the3)*cos(the4)*cos(the5)^2*sin(the2) + Ixx6*cos(the2)*cos(the6)*sin(the3)*sin(the4)*sin(the5)*sin(the6) + Ixx6*cos(the3)*cos(the6)*sin(the2)*sin(the4)*sin(the5)*sin(the6) - Iyy6*cos(the2)*cos(the6)*sin(the3)*sin(the4)*sin(the5)*sin(the6) - Iyy6*cos(the3)*cos(the6)*sin(the2)*sin(the4)*sin(the5)*sin(the6) + m5*x5^2*cos(the2)*cos(the4)*cos(the5)*sin(the3)*sin(the5) + m5*x5^2*cos(the3)*cos(the4)*cos(the5)*sin(the2)*sin(the5) - m5*y5^2*cos(the2)*cos(the4)*cos(the5)*sin(the3)*sin(the5) - m5*y5^2*cos(the3)*cos(the4)*cos(the5)*sin(the2)*sin(the5) + m6*y6^2*cos(the2)*cos(the4)*cos(the5)*sin(the3)*sin(the5) + m6*y6^2*cos(the3)*cos(the4)*cos(the5)*sin(the2)*sin(the5) - m6*z6^2*cos(the2)*cos(the4)*cos(the5)*sin(the3)*sin(the5) - m6*z6^2*cos(the3)*cos(the4)*cos(the5)*sin(the2)*sin(the5) - d4*m6*y6*cos(the2)*cos(the4)*cos(the5)*sin(the3)*sin(the6) - d4*m6*y6*cos(the3)*cos(the4)*cos(the5)*sin(the2)*sin(the6) + 2*m6*x6*z6*cos(the2)*cos(the3)*cos(the5)*cos(the6)*sin(the5) - a3*m6*y6*cos(the4)*cos(the5)*sin(the2)*sin(the3)*sin(the6) - m6*y6*z6*cos(the2)*cos(the5)*cos(the6)*sin(the3)*sin(the4) - m6*y6*z6*cos(the3)*cos(the5)*cos(the6)*sin(the2)*sin(the4) - 2*m6*y6*z6*cos(the2)*cos(the3)*cos(the5)*sin(the5)*sin(the6) - m6*x6*z6*cos(the2)*cos(the5)*sin(the3)*sin(the4)*sin(the6) - m6*x6*z6*cos(the3)*cos(the5)*sin(the2)*sin(the4)*sin(the6) - 2*m6*x6*z6*cos(the5)*cos(the6)*sin(the2)*sin(the3)*sin(the5) + m6*x6^2*cos(the2)*cos(the4)*cos(the5)*cos(the6)^2*sin(the3)*sin(the5) + m6*x6^2*cos(the3)*cos(the4)*cos(the5)*cos(the6)^2*sin(the2)*sin(the5) - m6*y6^2*cos(the2)*cos(the4)*cos(the5)*cos(the6)^2*sin(the3)*sin(the5) - m6*y6^2*cos(the3)*cos(the4)*cos(the5)*cos(the6)^2*sin(the2)*sin(the5) + 2*m6*y6*z6*cos(the5)*sin(the2)*sin(the3)*sin(the5)*sin(the6) + 2*m6*x6*y6*cos(the2)*cos(the3)*cos(the5)^2*cos(the6)*sin(the6) + 2*m6*x6*z6*cos(the2)*cos(the4)*cos(the5)^2*cos(the6)*sin(the3) + 2*m6*x6*z6*cos(the3)*cos(the4)*cos(the5)^2*cos(the6)*sin(the2) - 2*m6*y6*z6*cos(the2)*cos(the4)*cos(the5)^2*sin(the3)*sin(the6) - 2*m6*y6*z6*cos(the3)*cos(the4)*cos(the5)^2*sin(the2)*sin(the6) - 2*m6*x6*y6*cos(the2)*cos(the6)^2*sin(the3)*sin(the4)*sin(the5) - 2*m6*x6*y6*cos(the3)*cos(the6)^2*sin(the2)*sin(the4)*sin(the5) - 2*m6*x6*y6*cos(the5)^2*cos(the6)*sin(the2)*sin(the3)*sin(the6) - 2*IPx6*cos(the2)*cos(the4)*cos(the5)*cos(the6)*sin(the3)*sin(the5)*sin(the6) - 2*IPx6*cos(the3)*cos(the4)*cos(the5)*cos(the6)*sin(the2)*sin(the5)*sin(the6) - a3*m6*x6*cos(the2)*cos(the3)*cos(the4)*cos(the5)*cos(the6) + a3*m6*y6*cos(the2)*cos(the3)*cos(the4)*cos(the5)*sin(the6) + d4*m6*x6*cos(the2)*cos(the4)*cos(the5)*cos(the6)*sin(the3) + d4*m6*x6*cos(the3)*cos(the4)*cos(the5)*cos(the6)*sin(the2) - m6*x6^2*cos(the2)*cos(the6)*sin(the3)*sin(the4)*sin(the5)*sin(the6) - m6*x6^2*cos(the3)*cos(the6)*sin(the2)*sin(the4)*sin(the5)*sin(the6) + m6*y6^2*cos(the2)*cos(the6)*sin(the3)*sin(the4)*sin(the5)*sin(the6) + m6*y6^2*cos(the3)*cos(the6)*sin(the2)*sin(the4)*sin(the5)*sin(the6) + a3*m6*x6*cos(the4)*cos(the5)*cos(the6)*sin(the2)*sin(the3) - 2*m6*x6*y6*cos(the2)*cos(the4)*cos(the5)*cos(the6)*sin(the3)*sin(the5)*sin(the6) - 2*m6*x6*y6*cos(the3)*cos(the4)*cos(the5)*cos(the6)*sin(the2)*sin(the5)*sin(the6),IPy5*cos(the2)*cos(the3)*cos(the5) + IPx6*cos(the2)*cos(the3)*sin(the5) + IPz5*cos(the2)*cos(the3)*sin(the5) - IPy5*cos(the5)*sin(the2)*sin(the3) - Ixx6*cos(the2)*sin(the3)*sin(the4) - Ixx6*cos(the3)*sin(the2)*sin(the4) - Izz5*cos(the2)*sin(the3)*sin(the4) - Izz5*cos(the3)*sin(the2)*sin(the4) - IPx6*sin(the2)*sin(the3)*sin(the5) - IPz5*sin(the2)*sin(the3)*sin(the5) - IPy6*cos(the2)*cos(the3)*cos(the5)*cos(the6) + IPx6*cos(the2)*cos(the4)*cos(the5)*sin(the3) + IPx6*cos(the3)*cos(the4)*cos(the5)*sin(the2) + IPz5*cos(the2)*cos(the4)*cos(the5)*sin(the3) + IPz5*cos(the3)*cos(the4)*cos(the5)*sin(the2) - IPz6*cos(the2)*cos(the3)*cos(the5)*sin(the6) - IPy5*cos(the2)*cos(the4)*sin(the3)*sin(the5) - IPy5*cos(the3)*cos(the4)*sin(the2)*sin(the5) + IPy6*cos(the5)*cos(the6)*sin(the2)*sin(the3) + IPz6*cos(the5)*sin(the2)*sin(the3)*sin(the6) - m5*x5^2*cos(the2)*sin(the3)*sin(the4) - m5*x5^2*cos(the3)*sin(the2)*sin(the4) - m5*y5^2*cos(the2)*sin(the3)*sin(the4) - m5*y5^2*cos(the3)*sin(the2)*sin(the4) - m6*y6^2*cos(the2)*sin(the3)*sin(the4) - m6*y6^2*cos(the3)*sin(the2)*sin(the4) - m6*z6^2*cos(the2)*sin(the3)*sin(the4) - m6*z6^2*cos(the3)*sin(the2)*sin(the4) + a1*m5*y5*cos(the5)*sin(the4) + a1*m6*z6*cos(the5)*sin(the4) + a1*m5*x5*sin(the4)*sin(the5) - 2*IPx6*cos(the2)*cos(the3)*cos(the6)^2*sin(the5) + Ixx6*cos(the2)*cos(the6)^2*sin(the3)*sin(the4) + Ixx6*cos(the3)*cos(the6)^2*sin(the2)*sin(the4) - Iyy6*cos(the2)*cos(the6)^2*sin(the3)*sin(the4) - Iyy6*cos(the3)*cos(the6)^2*sin(the2)*sin(the4) + 2*IPx6*cos(the6)^2*sin(the2)*sin(the3)*sin(the5) + Ixx6*cos(the2)*cos(the3)*cos(the6)*sin(the5)*sin(the6) - Iyy6*cos(the2)*cos(the3)*cos(the6)*sin(the5)*sin(the6) + 2*IPx6*cos(the2)*cos(the6)*sin(the3)*sin(the4)*sin(the6) + 2*IPx6*cos(the3)*cos(the6)*sin(the2)*sin(the4)*sin(the6) + IPz6*cos(the2)*cos(the4)*sin(the3)*sin(the5)*sin(the6) + IPz6*cos(the3)*cos(the4)*sin(the2)*sin(the5)*sin(the6) - Ixx6*cos(the6)*sin(the2)*sin(the3)*sin(the5)*sin(the6) + Iyy6*cos(the6)*sin(the2)*sin(the3)*sin(the5)*sin(the6) + a2*m5*y5*cos(the2)*cos(the5)*sin(the4) + a2*m6*z6*cos(the2)*cos(the5)*sin(the4) + m5*y5*z5*cos(the2)*cos(the3)*cos(the5) + a2*m5*x5*cos(the2)*sin(the4)*sin(the5) + a1*m6*x6*cos(the6)*sin(the4)*sin(the5) - 2*IPx6*cos(the2)*cos(the4)*cos(the5)*cos(the6)^2*sin(the3) - 2*IPx6*cos(the3)*cos(the4)*cos(the5)*cos(the6)^2*sin(the2) + m6*x6*y6*cos(the2)*cos(the3)*sin(the5) + m5*x5*z5*cos(the2)*cos(the3)*sin(the5) - a1*m6*y6*sin(the4)*sin(the5)*sin(the6) - m5*y5*z5*cos(the5)*sin(the2)*sin(the3) - m6*x6*y6*sin(the2)*sin(the3)*sin(the5) - m5*x5*z5*sin(the2)*sin(the3)*sin(the5) - m6*x6^2*cos(the2)*cos(the6)^2*sin(the3)*sin(the4) - m6*x6^2*cos(the3)*cos(the6)^2*sin(the2)*sin(the4) + m6*y6^2*cos(the2)*cos(the6)^2*sin(the3)*sin(the4) + m6*y6^2*cos(the3)*cos(the6)^2*sin(the2)*sin(the4) + IPy6*cos(the2)*cos(the4)*cos(the6)*sin(the3)*sin(the5) + IPy6*cos(the3)*cos(the4)*cos(the6)*sin(the2)*sin(the5) + a3*m5*y5*cos(the2)*cos(the3)*cos(the5)*sin(the4) + a3*m6*z6*cos(the2)*cos(the3)*cos(the5)*sin(the4) + m6*x6^2*cos(the6)*sin(the2)*sin(the3)*sin(the5)*sin(the6) - m6*y6^2*cos(the6)*sin(the2)*sin(the3)*sin(the5)*sin(the6) - m6*y6*z6*cos(the2)*cos(the3)*cos(the5)*cos(the6) + a3*m5*x5*cos(the2)*cos(the3)*sin(the4)*sin(the5) + a2*m6*x6*cos(the2)*cos(the6)*sin(the4)*sin(the5) - d4*m5*y5*cos(the2)*cos(the5)*sin(the3)*sin(the4) - d4*m5*y5*cos(the3)*cos(the5)*sin(the2)*sin(the4) - d4*m6*z6*cos(the2)*cos(the5)*sin(the3)*sin(the4) - d4*m6*z6*cos(the3)*cos(the5)*sin(the2)*sin(the4) + m6*x6*y6*cos(the2)*cos(the4)*cos(the5)*sin(the3) + m6*x6*y6*cos(the3)*cos(the4)*cos(the5)*sin(the2) + m5*x5*z5*cos(the2)*cos(the4)*cos(the5)*sin(the3) + m5*x5*z5*cos(the3)*cos(the4)*cos(the5)*sin(the2) - m6*x6*z6*cos(the2)*cos(the3)*cos(the5)*sin(the6) - a3*m5*y5*cos(the5)*sin(the2)*sin(the3)*sin(the4) - a2*m6*y6*cos(the2)*sin(the4)*sin(the5)*sin(the6) - a3*m6*z6*cos(the5)*sin(the2)*sin(the3)*sin(the4) - d4*m5*x5*cos(the2)*sin(the3)*sin(the4)*sin(the5) - d4*m5*x5*cos(the3)*sin(the2)*sin(the4)*sin(the5) - m5*y5*z5*cos(the2)*cos(the4)*sin(the3)*sin(the5) - m5*y5*z5*cos(the3)*cos(the4)*sin(the2)*sin(the5) + m6*y6*z6*cos(the5)*cos(the6)*sin(the2)*sin(the3) - a3*m5*x5*sin(the2)*sin(the3)*sin(the4)*sin(the5) + m6*x6*z6*cos(the5)*sin(the2)*sin(the3)*sin(the6) - 2*m6*x6*y6*cos(the2)*cos(the3)*cos(the6)^2*sin(the5) + 2*m6*x6*y6*cos(the6)^2*sin(the2)*sin(the3)*sin(the5) + Ixx6*cos(the2)*cos(the4)*cos(the5)*cos(the6)*sin(the3)*sin(the6) + Ixx6*cos(the3)*cos(the4)*cos(the5)*cos(the6)*sin(the2)*sin(the6) - Iyy6*cos(the2)*cos(the4)*cos(the5)*cos(the6)*sin(the3)*sin(the6) - Iyy6*cos(the3)*cos(the4)*cos(the5)*cos(the6)*sin(the2)*sin(the6) - m6*x6^2*cos(the2)*cos(the3)*cos(the6)*sin(the5)*sin(the6) + m6*y6^2*cos(the2)*cos(the3)*cos(the6)*sin(the5)*sin(the6) - a3*m6*y6*cos(the2)*cos(the3)*sin(the4)*sin(the5)*sin(the6) - d4*m6*x6*cos(the2)*cos(the6)*sin(the3)*sin(the4)*sin(the5) - d4*m6*x6*cos(the3)*cos(the6)*sin(the2)*sin(the4)*sin(the5) + m6*y6*z6*cos(the2)*cos(the4)*cos(the6)*sin(the3)*sin(the5) + m6*y6*z6*cos(the3)*cos(the4)*cos(the6)*sin(the2)*sin(the5) - a3*m6*x6*cos(the6)*sin(the2)*sin(the3)*sin(the4)*sin(the5) + d4*m6*y6*cos(the2)*sin(the3)*sin(the4)*sin(the5)*sin(the6) + d4*m6*y6*cos(the3)*sin(the2)*sin(the4)*sin(the5)*sin(the6) + 2*m6*x6*y6*cos(the2)*cos(the6)*sin(the3)*sin(the4)*sin(the6) + 2*m6*x6*y6*cos(the3)*cos(the6)*sin(the2)*sin(the4)*sin(the6) + m6*x6*z6*cos(the2)*cos(the4)*sin(the3)*sin(the5)*sin(the6) + m6*x6*z6*cos(the3)*cos(the4)*sin(the2)*sin(the5)*sin(the6) + a3*m6*y6*sin(the2)*sin(the3)*sin(the4)*sin(the5)*sin(the6) - 2*m6*x6*y6*cos(the2)*cos(the4)*cos(the5)*cos(the6)^2*sin(the3) - 2*m6*x6*y6*cos(the3)*cos(the4)*cos(the5)*cos(the6)^2*sin(the2) - m6*x6^2*cos(the2)*cos(the4)*cos(the5)*cos(the6)*sin(the3)*sin(the6) - m6*x6^2*cos(the3)*cos(the4)*cos(the5)*cos(the6)*sin(the2)*sin(the6) + m6*y6^2*cos(the2)*cos(the4)*cos(the5)*cos(the6)*sin(the3)*sin(the6) + m6*y6^2*cos(the3)*cos(the4)*cos(the5)*cos(the6)*sin(the2)*sin(the6) + a3*m6*x6*cos(the2)*cos(the3)*cos(the6)*sin(the4)*sin(the5),Izz6*cos(the5)*sin(the2)*sin(the3) - Izz6*cos(the2)*cos(the3)*cos(the5) + IPz6*cos(the2)*cos(the3)*cos(the6)*sin(the5) - IPy6*cos(the2)*cos(the6)*sin(the3)*sin(the4) - IPy6*cos(the3)*cos(the6)*sin(the2)*sin(the4) - IPy6*cos(the2)*cos(the3)*sin(the5)*sin(the6) + Izz6*cos(the2)*cos(the4)*sin(the3)*sin(the5) + Izz6*cos(the3)*cos(the4)*sin(the2)*sin(the5) - m6*x6^2*cos(the2)*cos(the3)*cos(the5) - m6*y6^2*cos(the2)*cos(the3)*cos(the5) - IPz6*cos(the2)*sin(the3)*sin(the4)*sin(the6) - IPz6*cos(the3)*sin(the2)*sin(the4)*sin(the6) - IPz6*cos(the6)*sin(the2)*sin(the3)*sin(the5) + IPy6*sin(the2)*sin(the3)*sin(the5)*sin(the6) + m6*x6^2*cos(the5)*sin(the2)*sin(the3) + m6*y6^2*cos(the5)*sin(the2)*sin(the3) - a1*m6*x6*cos(the4)*cos(the6) + a1*m6*y6*cos(the4)*sin(the6) + m6*x6^2*cos(the2)*cos(the4)*sin(the3)*sin(the5) + m6*x6^2*cos(the3)*cos(the4)*sin(the2)*sin(the5) + m6*y6^2*cos(the2)*cos(the4)*sin(the3)*sin(the5) + m6*y6^2*cos(the3)*cos(the4)*sin(the2)*sin(the5) - a2*m6*x6*cos(the2)*cos(the4)*cos(the6) + a2*m6*y6*cos(the2)*cos(the4)*sin(the6) + a1*m6*y6*cos(the5)*cos(the6)*sin(the4) + a1*m6*x6*cos(the5)*sin(the4)*sin(the6) + IPz6*cos(the2)*cos(the4)*cos(the5)*cos(the6)*sin(the3) + IPz6*cos(the3)*cos(the4)*cos(the5)*cos(the6)*sin(the2) - IPy6*cos(the2)*cos(the4)*cos(the5)*sin(the3)*sin(the6) - IPy6*cos(the3)*cos(the4)*cos(the5)*sin(the2)*sin(the6) - a3*m6*x6*cos(the2)*cos(the3)*cos(the4)*cos(the6) + a3*m6*y6*cos(the2)*cos(the3)*cos(the4)*sin(the6) + a2*m6*y6*cos(the2)*cos(the5)*cos(the6)*sin(the4) + d4*m6*x6*cos(the2)*cos(the4)*cos(the6)*sin(the3) + d4*m6*x6*cos(the3)*cos(the4)*cos(the6)*sin(the2) + a3*m6*x6*cos(the4)*cos(the6)*sin(the2)*sin(the3) + a2*m6*x6*cos(the2)*cos(the5)*sin(the4)*sin(the6) - d4*m6*y6*cos(the2)*cos(the4)*sin(the3)*sin(the6) - d4*m6*y6*cos(the3)*cos(the4)*sin(the2)*sin(the6) + m6*x6*z6*cos(the2)*cos(the3)*cos(the6)*sin(the5) - a3*m6*y6*cos(the4)*sin(the2)*sin(the3)*sin(the6) - m6*y6*z6*cos(the2)*cos(the6)*sin(the3)*sin(the4) - m6*y6*z6*cos(the3)*cos(the6)*sin(the2)*sin(the4) - m6*y6*z6*cos(the2)*cos(the3)*sin(the5)*sin(the6) - m6*x6*z6*cos(the2)*sin(the3)*sin(the4)*sin(the6) - m6*x6*z6*cos(the3)*sin(the2)*sin(the4)*sin(the6) - m6*x6*z6*cos(the6)*sin(the2)*sin(the3)*sin(the5) + m6*y6*z6*sin(the2)*sin(the3)*sin(the5)*sin(the6) - d4*m6*y6*cos(the2)*cos(the5)*cos(the6)*sin(the3)*sin(the4) - d4*m6*y6*cos(the3)*cos(the5)*cos(the6)*sin(the2)*sin(the4) + m6*x6*z6*cos(the2)*cos(the4)*cos(the5)*cos(the6)*sin(the3) + m6*x6*z6*cos(the3)*cos(the4)*cos(the5)*cos(the6)*sin(the2) - a3*m6*y6*cos(the5)*cos(the6)*sin(the2)*sin(the3)*sin(the4) - d4*m6*x6*cos(the2)*cos(the5)*sin(the3)*sin(the4)*sin(the6) - d4*m6*x6*cos(the3)*cos(the5)*sin(the2)*sin(the4)*sin(the6) - m6*y6*z6*cos(the2)*cos(the4)*cos(the5)*sin(the3)*sin(the6) - m6*y6*z6*cos(the3)*cos(the4)*cos(the5)*sin(the2)*sin(the6) - a3*m6*x6*cos(the5)*sin(the2)*sin(the3)*sin(the4)*sin(the6) + a3*m6*y6*cos(the2)*cos(the3)*cos(the5)*cos(the6)*sin(the4) + a3*m6*x6*cos(the2)*cos(the3)*cos(the5)*sin(the4)*sin(the6);
 IPy2*cos(the2) + IPz2*sin(the2) + IPy3*cos(the2)*cos(the3) + IPx4*cos(the2)*sin(the3) + IPx4*cos(the3)*sin(the2) + IPz3*cos(the2)*sin(the3) + IPz3*cos(the3)*sin(the2) - IPy3*sin(the2)*sin(the3) - IPy4*cos(the2)*cos(the3)*cos(the4) + IPx5*cos(the2)*cos(the3)*sin(the4) - IPx6*cos(the2)*cos(the5)*sin(the3) - IPx6*cos(the3)*cos(the5)*sin(the2) - IPz4*cos(the2)*cos(the3)*sin(the4) - IPz5*cos(the2)*cos(the5)*sin(the3) - IPz5*cos(the3)*cos(the5)*sin(the2) + IPy4*cos(the4)*sin(the2)*sin(the3) + IPy5*cos(the2)*sin(the3)*sin(the5) + IPy5*cos(the3)*sin(the2)*sin(the5) - IPx5*sin(the2)*sin(the3)*sin(the4) + IPz4*sin(the2)*sin(the3)*sin(the4) + a2*m3*z3*sin(the2) + m2*y2*z2*cos(the2) - 2*IPx4*cos(the2)*cos(the4)^2*sin(the3) - 2*IPx4*cos(the3)*cos(the4)^2*sin(the2) + m2*x2*z2*sin(the2) + IPy5*cos(the2)*cos(the3)*cos(the4)*cos(the5) + IPx6*cos(the2)*cos(the3)*cos(the4)*sin(the5) + IPz5*cos(the2)*cos(the3)*cos(the4)*sin(the5) + IPz6*cos(the2)*cos(the3)*cos(the6)*sin(the4) - IPy5*cos(the4)*cos(the5)*sin(the2)*sin(the3) - IPy6*cos(the2)*cos(the3)*sin(the4)*sin(the6) - IPy6*cos(the2)*cos(the6)*sin(the3)*sin(the5) - IPy6*cos(the3)*cos(the6)*sin(the2)*sin(the5) + Ixx4*cos(the2)*cos(the4)*sin(the3)*sin(the4) + Ixx4*cos(the3)*cos(the4)*sin(the2)*sin(the4) - Ixx6*cos(the2)*cos(the4)*sin(the3)*sin(the4) - Ixx6*cos(the3)*cos(the4)*sin(the2)*sin(the4) - Iyy4*cos(the2)*cos(the4)*sin(the3)*sin(the4) - Iyy4*cos(the3)*cos(the4)*sin(the2)*sin(the4) + Iyy5*cos(the2)*cos(the4)*sin(the3)*sin(the4) + Iyy5*cos(the3)*cos(the4)*sin(the2)*sin(the4) - Izz5*cos(the2)*cos(the4)*sin(the3)*sin(the4) - Izz5*cos(the3)*cos(the4)*sin(the2)*sin(the4) + Izz6*cos(the2)*cos(the4)*sin(the3)*sin(the4) + Izz6*cos(the3)*cos(the4)*sin(the2)*sin(the4) - IPx6*cos(the4)*sin(the2)*sin(the3)*sin(the5) - IPz5*cos(the4)*sin(the2)*sin(the3)*sin(the5) - IPz6*cos(the6)*sin(the2)*sin(the3)*sin(the4) - IPz6*cos(the2)*sin(the3)*sin(the5)*sin(the6) - IPz6*cos(the3)*sin(the2)*sin(the5)*sin(the6) + IPy6*sin(the2)*sin(the3)*sin(the4)*sin(the6) - a2*m4*y4*cos(the4)*sin(the2) + a2*m5*z5*cos(the4)*sin(the2) + m3*y3*z3*cos(the2)*cos(the3) - a2*m4*x4*sin(the2)*sin(the4) - 2*IPx5*cos(the2)*cos(the3)*cos(the5)^2*sin(the4) + 2*IPx6*cos(the2)*cos(the4)^2*cos(the5)*sin(the3) + 2*IPx6*cos(the3)*cos(the4)^2*cos(the5)*sin(the2) + 2*IPx6*cos(the2)*cos(the5)*cos(the6)^2*sin(the3) + 2*IPx6*cos(the3)*cos(the5)*cos(the6)^2*sin(the2) + 2*IPz5*cos(the2)*cos(the4)^2*cos(the5)*sin(the3) + 2*IPz5*cos(the3)*cos(the4)^2*cos(the5)*sin(the2) + m4*x4*y4*cos(the2)*sin(the3) + m4*x4*y4*cos(the3)*sin(the2) + m3*x3*z3*cos(the2)*sin(the3) + m3*x3*z3*cos(the3)*sin(the2) - 2*IPy5*cos(the2)*cos(the4)^2*sin(the3)*sin(the5) - 2*IPy5*cos(the3)*cos(the4)^2*sin(the2)*sin(the5) - m3*y3*z3*sin(the2)*sin(the3) + 2*IPx5*cos(the5)^2*sin(the2)*sin(the3)*sin(the4) + Ixx5*cos(the2)*cos(the3)*cos(the5)*sin(the4)*sin(the5) - Ixx6*cos(the2)*cos(the5)*cos(the6)*sin(the3)*sin(the6) - Ixx6*cos(the3)*cos(the5)*cos(the6)*sin(the2)*sin(the6) - Iyy5*cos(the2)*cos(the3)*cos(the5)*sin(the4)*sin(the5) + Iyy6*cos(the2)*cos(the3)*cos(the5)*sin(the4)*sin(the5) + Iyy6*cos(the2)*cos(the5)*cos(the6)*sin(the3)*sin(the6) + Iyy6*cos(the3)*cos(the5)*cos(the6)*sin(the2)*sin(the6) - Izz6*cos(the2)*cos(the3)*cos(the5)*sin(the4)*sin(the5) + IPz6*cos(the4)*cos(the5)*sin(the2)*sin(the3)*sin(the6) - Ixx5*cos(the5)*sin(the2)*sin(the3)*sin(the4)*sin(the5) + Iyy5*cos(the5)*sin(the2)*sin(the3)*sin(the4)*sin(the5) - Iyy6*cos(the5)*sin(the2)*sin(the3)*sin(the4)*sin(the5) + Izz6*cos(the5)*sin(the2)*sin(the3)*sin(the4)*sin(the5) - m4*x4^2*cos(the2)*cos(the4)*sin(the3)*sin(the4) - m4*x4^2*cos(the3)*cos(the4)*sin(the2)*sin(the4) + m6*x6^2*cos(the2)*cos(the4)*sin(the3)*sin(the4) + m6*x6^2*cos(the3)*cos(the4)*sin(the2)*sin(the4) + m4*y4^2*cos(the2)*cos(the4)*sin(the3)*sin(the4) + m4*y4^2*cos(the3)*cos(the4)*sin(the2)*sin(the4) - m5*y5^2*cos(the2)*cos(the4)*sin(the3)*sin(the4) - m5*y5^2*cos(the3)*cos(the4)*sin(the2)*sin(the4) + m5*z5^2*cos(the2)*cos(the4)*sin(the3)*sin(the4) + m5*z5^2*cos(the3)*cos(the4)*sin(the2)*sin(the4) - m6*z6^2*cos(the2)*cos(the4)*sin(the3)*sin(the4) - m6*z6^2*cos(the3)*cos(the4)*sin(the2)*sin(the4) - d4*m4*y4*cos(the2)*cos(the3)*cos(the4) + d4*m5*z5*cos(the2)*cos(the3)*cos(the4) - a3*m4*y4*cos(the2)*cos(the4)*sin(the3) - a3*m4*y4*cos(the3)*cos(the4)*sin(the2) - a2*m6*y6*cos(the4)*cos(the6)*sin(the2) + a3*m5*z5*cos(the2)*cos(the4)*sin(the3) + a3*m5*z5*cos(the3)*cos(the4)*sin(the2) - d4*m4*x4*cos(the2)*cos(the3)*sin(the4) - m4*y4*z4*cos(the2)*cos(the3)*cos(the4) - a3*m4*x4*cos(the2)*sin(the3)*sin(the4) - a3*m4*x4*cos(the3)*sin(the2)*sin(the4) - a2*m5*x5*cos(the5)*sin(the2)*sin(the4) - a2*m6*x6*cos(the4)*sin(the2)*sin(the6) - 2*IPx6*cos(the2)*cos(the3)*cos(the4)*cos(the6)^2*sin(the5) - 2*IPz6*cos(the2)*cos(the3)*cos(the5)^2*cos(the6)*sin(the4) + d4*m4*y4*cos(the4)*sin(the2)*sin(the3) - d4*m5*z5*cos(the4)*sin(the2)*sin(the3) + m5*x5*y5*cos(the2)*cos(the3)*sin(the4) - m6*x6*y6*cos(the2)*cos(the5)*sin(the3) - m6*x6*y6*cos(the3)*cos(the5)*sin(the2) - m4*x4*z4*cos(the2)*cos(the3)*sin(the4) - m5*x5*z5*cos(the2)*cos(the5)*sin(the3) - m5*x5*z5*cos(the3)*cos(the5)*sin(the2) + a2*m5*y5*sin(the2)*sin(the4)*sin(the5) + a2*m6*z6*sin(the2)*sin(the4)*sin(the5) + 2*IPy6*cos(the2)*cos(the3)*cos(the5)^2*sin(the4)*sin(the6) + 2*IPy6*cos(the2)*cos(the4)^2*cos(the6)*sin(the3)*sin(the5) + 2*IPy6*cos(the3)*cos(the4)^2*cos(the6)*sin(the2)*sin(the5) + Ixx5*cos(the2)*cos(the4)*cos(the5)^2*sin(the3)*sin(the4) + Ixx5*cos(the3)*cos(the4)*cos(the5)^2*sin(the2)*sin(the4) + Ixx6*cos(the2)*cos(the4)*cos(the6)^2*sin(the3)*sin(the4) + Ixx6*cos(the3)*cos(the4)*cos(the6)^2*sin(the2)*sin(the4) - Iyy5*cos(the2)*cos(the4)*cos(the5)^2*sin(the3)*sin(the4) - Iyy5*cos(the3)*cos(the4)*cos(the5)^2*sin(the2)*sin(the4) + Iyy6*cos(the2)*cos(the4)*cos(the5)^2*sin(the3)*sin(the4) + Iyy6*cos(the3)*cos(the4)*cos(the5)^2*sin(the2)*sin(the4) - Iyy6*cos(the2)*cos(the4)*cos(the6)^2*sin(the3)*sin(the4) - Iyy6*cos(the3)*cos(the4)*cos(the6)^2*sin(the2)*sin(the4) - Izz6*cos(the2)*cos(the4)*cos(the5)^2*sin(the3)*sin(the4) - Izz6*cos(the3)*cos(the4)*cos(the5)^2*sin(the2)*sin(the4) + d4*m4*x4*sin(the2)*sin(the3)*sin(the4) + m4*y4*z4*cos(the4)*sin(the2)*sin(the3) + m5*y5*z5*cos(the2)*sin(the3)*sin(the5) + m5*y5*z5*cos(the3)*sin(the2)*sin(the5) + 2*IPx6*cos(the4)*cos(the6)^2*sin(the2)*sin(the3)*sin(the5) + 2*IPz6*cos(the2)*cos(the4)^2*sin(the3)*sin(the5)*sin(the6) + 2*IPz6*cos(the3)*cos(the4)^2*sin(the2)*sin(the5)*sin(the6) + 2*IPz6*cos(the5)^2*cos(the6)*sin(the2)*sin(the3)*sin(the4) - m5*x5*y5*sin(the2)*sin(the3)*sin(the4) + m4*x4*z4*sin(the2)*sin(the3)*sin(the4) - 2*IPy6*cos(the5)^2*sin(the2)*sin(the3)*sin(the4)*sin(the6) - 4*IPx6*cos(the2)*cos(the4)^2*cos(the5)*cos(the6)^2*sin(the3) - 4*IPx6*cos(the3)*cos(the4)^2*cos(the5)*cos(the6)^2*sin(the2) - 2*m4*x4*y4*cos(the2)*cos(the4)^2*sin(the3) - 2*m4*x4*y4*cos(the3)*cos(the4)^2*sin(the2) - IPy6*cos(the2)*cos(the3)*cos(the4)*cos(the5)*cos(the6) - IPz6*cos(the2)*cos(the3)*cos(the4)*cos(the5)*sin(the6) + IPy6*cos(the4)*cos(the5)*cos(the6)*sin(the2)*sin(the3) - d4*m6*y6*cos(the2)*cos(the3)*cos(the4)*cos(the6) - a3*m6*y6*cos(the2)*cos(the4)*cos(the6)*sin(the3) - a3*m6*y6*cos(the3)*cos(the4)*cos(the6)*sin(the2) - d4*m5*x5*cos(the2)*cos(the3)*cos(the5)*sin(the4) - d4*m6*x6*cos(the2)*cos(the3)*cos(the4)*sin(the6) + m5*x5^2*cos(the5)*sin(the2)*sin(the3)*sin(the4)*sin(the5) - m5*y5^2*cos(the5)*sin(the2)*sin(the3)*sin(the4)*sin(the5) + m6*y6^2*cos(the5)*sin(the2)*sin(the3)*sin(the4)*sin(the5) - m6*z6^2*cos(the5)*sin(the2)*sin(the3)*sin(the4)*sin(the5) + m5*y5*z5*cos(the2)*cos(the3)*cos(the4)*cos(the5) - a3*m5*x5*cos(the2)*cos(the5)*sin(the3)*sin(the4) - a3*m5*x5*cos(the3)*cos(the5)*sin(the2)*sin(the4) - a3*m6*x6*cos(the2)*cos(the4)*sin(the3)*sin(the6) - a3*m6*x6*cos(the3)*cos(the4)*sin(the2)*sin(the6) - a2*m6*x6*cos(the5)*cos(the6)*sin(the2)*sin(the4) + d4*m5*y5*cos(the2)*cos(the3)*sin(the4)*sin(the5) + d4*m6*y6*cos(the4)*cos(the6)*sin(the2)*sin(the3) + d4*m6*z6*cos(the2)*cos(the3)*sin(the4)*sin(the5) + m6*x6*y6*cos(the2)*cos(the3)*cos(the4)*sin(the5) + m5*x5*z5*cos(the2)*cos(the3)*cos(the4)*sin(the5) + m6*x6*z6*cos(the2)*cos(the3)*cos(the6)*sin(the4) + a3*m5*y5*cos(the2)*sin(the3)*sin(the4)*sin(the5) + a3*m5*y5*cos(the3)*sin(the2)*sin(the4)*sin(the5) + a2*m6*y6*cos(the5)*sin(the2)*sin(the4)*sin(the6) + a3*m6*z6*cos(the2)*sin(the3)*sin(the4)*sin(the5) + a3*m6*z6*cos(the3)*sin(the2)*sin(the4)*sin(the5) + Ixx6*cos(the2)*cos(the3)*cos(the5)*cos(the6)^2*sin(the4)*sin(the5) + 2*Ixx6*cos(the2)*cos(the4)^2*cos(the5)*cos(the6)*sin(the3)*sin(the6) + 2*Ixx6*cos(the3)*cos(the4)^2*cos(the5)*cos(the6)*sin(the2)*sin(the6) - Iyy6*cos(the2)*cos(the3)*cos(the5)*cos(the6)^2*sin(the4)*sin(the5) - 2*Iyy6*cos(the2)*cos(the4)^2*cos(the5)*cos(the6)*sin(the3)*sin(the6) - 2*Iyy6*cos(the3)*cos(the4)^2*cos(the5)*cos(the6)*sin(the2)*sin(the6) + d4*m5*x5*cos(the5)*sin(the2)*sin(the3)*sin(the4) + d4*m6*x6*cos(the4)*sin(the2)*sin(the3)*sin(the6) - m5*y5*z5*cos(the4)*cos(the5)*sin(the2)*sin(the3) - m6*y6*z6*cos(the2)*cos(the3)*sin(the4)*sin(the6) - m6*y6*z6*cos(the2)*cos(the6)*sin(the3)*sin(the5) - m6*y6*z6*cos(the3)*cos(the6)*sin(the2)*sin(the5) - d4*m5*y5*sin(the2)*sin(the3)*sin(the4)*sin(the5) - d4*m6*z6*sin(the2)*sin(the3)*sin(the4)*sin(the5) - m6*x6*y6*cos(the4)*sin(the2)*sin(the3)*sin(the5) - m5*x5*z5*cos(the4)*sin(the2)*sin(the3)*sin(the5) - m6*x6*z6*cos(the6)*sin(the2)*sin(the3)*sin(the4) - m6*x6*z6*cos(the2)*sin(the3)*sin(the5)*sin(the6) - m6*x6*z6*cos(the3)*sin(the2)*sin(the5)*sin(the6) - Ixx6*cos(the5)*cos(the6)^2*sin(the2)*sin(the3)*sin(the4)*sin(the5) + Iyy6*cos(the5)*cos(the6)^2*sin(the2)*sin(the3)*sin(the4)*sin(the5) - m5*x5^2*cos(the2)*cos(the4)*cos(the5)^2*sin(the3)*sin(the4) - m5*x5^2*cos(the3)*cos(the4)*cos(the5)^2*sin(the2)*sin(the4) - m6*x6^2*cos(the2)*cos(the4)*cos(the6)^2*sin(the3)*sin(the4) - m6*x6^2*cos(the3)*cos(the4)*cos(the6)^2*sin(the2)*sin(the4) + m5*y5^2*cos(the2)*cos(the4)*cos(the5)^2*sin(the3)*sin(the4) + m5*y5^2*cos(the3)*cos(the4)*cos(the5)^2*sin(the2)*sin(the4) - m6*y6^2*cos(the2)*cos(the4)*cos(the5)^2*sin(the3)*sin(the4) - m6*y6^2*cos(the3)*cos(the4)*cos(the5)^2*sin(the2)*sin(the4) + m6*y6^2*cos(the2)*cos(the4)*cos(the6)^2*sin(the3)*sin(the4) + m6*y6^2*cos(the3)*cos(the4)*cos(the6)^2*sin(the2)*sin(the4) + m6*z6^2*cos(the2)*cos(the4)*cos(the5)^2*sin(the3)*sin(the4) + m6*z6^2*cos(the3)*cos(the4)*cos(the5)^2*sin(the2)*sin(the4) + m6*y6*z6*sin(the2)*sin(the3)*sin(the4)*sin(the6) - 2*m5*x5*y5*cos(the2)*cos(the3)*cos(the5)^2*sin(the4) + 2*m6*x6*y6*cos(the2)*cos(the4)^2*cos(the5)*sin(the3) + 2*m6*x6*y6*cos(the3)*cos(the4)^2*cos(the5)*sin(the2) + 2*m6*x6*y6*cos(the2)*cos(the5)*cos(the6)^2*sin(the3) + 2*m6*x6*y6*cos(the3)*cos(the5)*cos(the6)^2*sin(the2) + 2*m5*x5*z5*cos(the2)*cos(the4)^2*cos(the5)*sin(the3) + 2*m5*x5*z5*cos(the3)*cos(the4)^2*cos(the5)*sin(the2) + Ixx6*cos(the2)*cos(the4)*cos(the5)^2*cos(the6)^2*sin(the3)*sin(the4) + Ixx6*cos(the3)*cos(the4)*cos(the5)^2*cos(the6)^2*sin(the2)*sin(the4) - Iyy6*cos(the2)*cos(the4)*cos(the5)^2*cos(the6)^2*sin(the3)*sin(the4) - Iyy6*cos(the3)*cos(the4)*cos(the5)^2*cos(the6)^2*sin(the2)*sin(the4) - 2*m5*y5*z5*cos(the2)*cos(the4)^2*sin(the3)*sin(the5) - 2*m5*y5*z5*cos(the3)*cos(the4)^2*sin(the2)*sin(the5) + 2*m5*x5*y5*cos(the5)^2*sin(the2)*sin(the3)*sin(the4) + Ixx6*cos(the2)*cos(the3)*cos(the4)*cos(the6)*sin(the5)*sin(the6) - Iyy6*cos(the2)*cos(the3)*cos(the4)*cos(the6)*sin(the5)*sin(the6) + 2*IPx5*cos(the2)*cos(the4)*cos(the5)*sin(the3)*sin(the4)*sin(the5) + 2*IPx5*cos(the3)*cos(the4)*cos(the5)*sin(the2)*sin(the4)*sin(the5) + 2*IPx6*cos(the2)*cos(the4)*cos(the6)*sin(the3)*sin(the4)*sin(the6) + 2*IPx6*cos(the3)*cos(the4)*cos(the6)*sin(the2)*sin(the4)*sin(the6) - Ixx6*cos(the4)*cos(the6)*sin(the2)*sin(the3)*sin(the5)*sin(the6) + Iyy6*cos(the4)*cos(the6)*sin(the2)*sin(the3)*sin(the5)*sin(the6) - m5*x5^2*cos(the2)*cos(the3)*cos(the5)*sin(the4)*sin(the5) + m6*x6^2*cos(the2)*cos(the5)*cos(the6)*sin(the3)*sin(the6) + m6*x6^2*cos(the3)*cos(the5)*cos(the6)*sin(the2)*sin(the6) + m5*y5^2*cos(the2)*cos(the3)*cos(the5)*sin(the4)*sin(the5) - m6*y6^2*cos(the2)*cos(the3)*cos(the5)*sin(the4)*sin(the5) - m6*y6^2*cos(the2)*cos(the5)*cos(the6)*sin(the3)*sin(the6) - m6*y6^2*cos(the3)*cos(the5)*cos(the6)*sin(the2)*sin(the6) + m6*z6^2*cos(the2)*cos(the3)*cos(the5)*sin(the4)*sin(the5) + d4*m6*y6*cos(the2)*cos(the3)*cos(the5)*sin(the4)*sin(the6) - m6*x6*z6*cos(the2)*cos(the3)*cos(the4)*cos(the5)*sin(the6) + a3*m6*y6*cos(the2)*cos(the5)*sin(the3)*sin(the4)*sin(the6) + a3*m6*y6*cos(the3)*cos(the5)*sin(the2)*sin(the4)*sin(the6) + d4*m6*x6*cos(the5)*cos(the6)*sin(the2)*sin(the3)*sin(the4) + m6*y6*z6*cos(the4)*cos(the5)*cos(the6)*sin(the2)*sin(the3) + 2*IPx6*cos(the2)*cos(the4)*cos(the5)^2*cos(the6)*sin(the3)*sin(the4)*sin(the6) + 2*IPx6*cos(the3)*cos(the4)*cos(the5)^2*cos(the6)*sin(the2)*sin(the4)*sin(the6) - d4*m6*y6*cos(the5)*sin(the2)*sin(the3)*sin(the4)*sin(the6) + m6*x6*z6*cos(the4)*cos(the5)*sin(the2)*sin(the3)*sin(the6) - m6*x6^2*cos(the2)*cos(the3)*cos(the5)*cos(the6)^2*sin(the4)*sin(the5) - 2*m6*x6^2*cos(the2)*cos(the4)^2*cos(the5)*cos(the6)*sin(the3)*sin(the6) - 2*m6*x6^2*cos(the3)*cos(the4)^2*cos(the5)*cos(the6)*sin(the2)*sin(the6) + m6*y6^2*cos(the2)*cos(the3)*cos(the5)*cos(the6)^2*sin(the4)*sin(the5) + 2*m6*y6^2*cos(the2)*cos(the4)^2*cos(the5)*cos(the6)*sin(the3)*sin(the6) + 2*m6*y6^2*cos(the3)*cos(the4)^2*cos(the5)*cos(the6)*sin(the2)*sin(the6) + m6*x6^2*cos(the5)*cos(the6)^2*sin(the2)*sin(the3)*sin(the4)*sin(the5) - m6*y6^2*cos(the5)*cos(the6)^2*sin(the2)*sin(the3)*sin(the4)*sin(the5) - 2*m6*x6*y6*cos(the2)*cos(the3)*cos(the4)*cos(the6)^2*sin(the5) - 2*m6*x6*z6*cos(the2)*cos(the3)*cos(the5)^2*cos(the6)*sin(the4) + 2*m6*y6*z6*cos(the2)*cos(the3)*cos(the5)^2*sin(the4)*sin(the6) + 2*m6*y6*z6*cos(the2)*cos(the4)^2*cos(the6)*sin(the3)*sin(the5) + 2*m6*y6*z6*cos(the3)*cos(the4)^2*cos(the6)*sin(the2)*sin(the5) + 2*m6*x6*y6*cos(the4)*cos(the6)^2*sin(the2)*sin(the3)*sin(the5) + 2*m6*x6*z6*cos(the2)*cos(the4)^2*sin(the3)*sin(the5)*sin(the6) + 2*m6*x6*z6*cos(the3)*cos(the4)^2*sin(the2)*sin(the5)*sin(the6) + 2*m6*x6*z6*cos(the5)^2*cos(the6)*sin(the2)*sin(the3)*sin(the4) - m6*x6^2*cos(the2)*cos(the4)*cos(the5)^2*cos(the6)^2*sin(the3)*sin(the4) - m6*x6^2*cos(the3)*cos(the4)*cos(the5)^2*cos(the6)^2*sin(the2)*sin(the4) + m6*y6^2*cos(the2)*cos(the4)*cos(the5)^2*cos(the6)^2*sin(the3)*sin(the4) + m6*y6^2*cos(the3)*cos(the4)*cos(the5)^2*cos(the6)^2*sin(the2)*sin(the4) - 2*m6*y6*z6*cos(the5)^2*sin(the2)*sin(the3)*sin(the4)*sin(the6) + 2*IPx6*cos(the2)*cos(the3)*cos(the5)*cos(the6)*sin(the4)*sin(the5)*sin(the6) + 2*IPz6*cos(the2)*cos(the4)*cos(the5)*cos(the6)*sin(the3)*sin(the4)*sin(the5) + 2*IPz6*cos(the3)*cos(the4)*cos(the5)*cos(the6)*sin(the2)*sin(the4)*sin(the5) - 4*m6*x6*y6*cos(the2)*cos(the4)^2*cos(the5)*cos(the6)^2*sin(the3) - 4*m6*x6*y6*cos(the3)*cos(the4)^2*cos(the5)*cos(the6)^2*sin(the2) - 2*IPy6*cos(the2)*cos(the4)*cos(the5)*sin(the3)*sin(the4)*sin(the5)*sin(the6) - 2*IPy6*cos(the3)*cos(the4)*cos(the5)*sin(the2)*sin(the4)*sin(the5)*sin(the6) - m6*x6^2*cos(the2)*cos(the3)*cos(the4)*cos(the6)*sin(the5)*sin(the6) + m6*y6^2*cos(the2)*cos(the3)*cos(the4)*cos(the6)*sin(the5)*sin(the6) - 2*IPx6*cos(the5)*cos(the6)*sin(the2)*sin(the3)*sin(the4)*sin(the5)*sin(the6) - d4*m6*x6*cos(the2)*cos(the3)*cos(the5)*cos(the6)*sin(the4) + m6*x6^2*cos(the4)*cos(the6)*sin(the2)*sin(the3)*sin(the5)*sin(the6) - m6*y6^2*cos(the4)*cos(the6)*sin(the2)*sin(the3)*sin(the5)*sin(the6) - m6*y6*z6*cos(the2)*cos(the3)*cos(the4)*cos(the5)*cos(the6) - a3*m6*x6*cos(the2)*cos(the5)*cos(the6)*sin(the3)*sin(the4) - a3*m6*x6*cos(the3)*cos(the5)*cos(the6)*sin(the2)*sin(the4) + 2*m5*x5*y5*cos(the2)*cos(the4)*cos(the5)*sin(the3)*sin(the4)*sin(the5) + 2*m5*x5*y5*cos(the3)*cos(the4)*cos(the5)*sin(the2)*sin(the4)*sin(the5) + 2*m6*x6*y6*cos(the2)*cos(the4)*cos(the6)*sin(the3)*sin(the4)*sin(the6) + 2*m6*x6*y6*cos(the3)*cos(the4)*cos(the6)*sin(the2)*sin(the4)*sin(the6) + 2*m6*x6*y6*cos(the2)*cos(the4)*cos(the5)^2*cos(the6)*sin(the3)*sin(the4)*sin(the6) + 2*m6*x6*y6*cos(the3)*cos(the4)*cos(the5)^2*cos(the6)*sin(the2)*sin(the4)*sin(the6) + 2*m6*x6*y6*cos(the2)*cos(the3)*cos(the5)*cos(the6)*sin(the4)*sin(the5)*sin(the6) + 2*m6*x6*z6*cos(the2)*cos(the4)*cos(the5)*cos(the6)*sin(the3)*sin(the4)*sin(the5) + 2*m6*x6*z6*cos(the3)*cos(the4)*cos(the5)*cos(the6)*sin(the2)*sin(the4)*sin(the5) - 2*m6*y6*z6*cos(the2)*cos(the4)*cos(the5)*sin(the3)*sin(the4)*sin(the5)*sin(the6) - 2*m6*y6*z6*cos(the3)*cos(the4)*cos(the5)*sin(the2)*sin(the4)*sin(the5)*sin(the6) - 2*m6*x6*y6*cos(the5)*cos(the6)*sin(the2)*sin(the3)*sin(the4)*sin(the5)*sin(the6),Ixx4 + Iyy5 + Izz2 + Izz3 + Izz6 + a2^2*m3 + a2^2*m4 + a2^2*m5 + a3^2*m4 + a2^2*m6 + a3^2*m5 + a3^2*m6 + d4^2*m4 + d4^2*m5 + d4^2*m6 + m2*x2^2 + m3*x3^2 + m5*x5^2 + m6*x6^2 + m2*y2^2 + m3*y3^2 + m4*y4^2 + m6*y6^2 + m4*z4^2 + m5*z5^2 - Ixx4*cos(the4)^2 + Ixx5*cos(the5)^2 + Ixx6*cos(the4)^2 + Iyy4*cos(the4)^2 - Iyy5*cos(the4)^2 - Iyy5*cos(the5)^2 + Iyy6*cos(the5)^2 + Izz5*cos(the4)^2 - Izz6*cos(the4)^2 - Izz6*cos(the5)^2 - IPx4*sin(2*the4) + IPx5*sin(2*the5) - Ixx5*cos(the4)^2*cos(the5)^2 - Ixx6*cos(the4)^2*cos(the6)^2 + Ixx6*cos(the5)^2*cos(the6)^2 + Iyy5*cos(the4)^2*cos(the5)^2 - Iyy6*cos(the4)^2*cos(the5)^2 + Iyy6*cos(the4)^2*cos(the6)^2 - Iyy6*cos(the5)^2*cos(the6)^2 + Izz6*cos(the4)^2*cos(the5)^2 + 2*d4*m4*z4 + m4*x4^2*cos(the4)^2 - m5*x5^2*cos(the5)^2 - m6*x6^2*cos(the4)^2 - m4*y4^2*cos(the4)^2 + m5*y5^2*cos(the4)^2 + m5*y5^2*cos(the5)^2 - m6*y6^2*cos(the5)^2 - m5*z5^2*cos(the4)^2 + m6*z6^2*cos(the4)^2 + m6*z6^2*cos(the5)^2 - m4*x4*y4*sin(2*the4) + m5*x5*y5*sin(2*the5) + m5*x5^2*cos(the4)^2*cos(the5)^2 + m6*x6^2*cos(the4)^2*cos(the6)^2 - m6*x6^2*cos(the5)^2*cos(the6)^2 - m5*y5^2*cos(the4)^2*cos(the5)^2 + m6*y6^2*cos(the4)^2*cos(the5)^2 - m6*y6^2*cos(the4)^2*cos(the6)^2 + m6*y6^2*cos(the5)^2*cos(the6)^2 - m6*z6^2*cos(the4)^2*cos(the5)^2 + 2*IPx6*cos(the4)*cos(the5)*sin(the4) + 2*IPz5*cos(the4)*cos(the5)*sin(the4) + 2*IPz6*cos(the5)*cos(the6)*sin(the5) - Ixx6*cos(the4)^2*cos(the5)^2*cos(the6)^2 + Iyy6*cos(the4)^2*cos(the5)^2*cos(the6)^2 - 2*IPy5*cos(the4)*sin(the4)*sin(the5) - 2*IPy6*cos(the5)*sin(the5)*sin(the6) + 2*a2*a3*m4*cos(the3) + 2*a2*a3*m5*cos(the3) + 2*a2*a3*m6*cos(the3) - 2*a2*d4*m4*sin(the3) - 2*a2*d4*m5*sin(the3) - 2*a2*d4*m6*sin(the3) + 2*a2*m3*x3*cos(the3) + 2*a3*m4*x4*cos(the4) + 2*d4*m5*y5*cos(the5) + 2*d4*m6*z6*cos(the5) - 2*a2*m3*y3*sin(the3) - 2*a3*m4*y4*sin(the4) - 2*a2*m4*z4*sin(the3) + 2*a3*m5*z5*sin(the4) + 2*d4*m5*x5*sin(the5) - 2*IPx5*cos(the4)^2*cos(the5)*sin(the5) - 2*IPx6*cos(the4)^2*cos(the6)*sin(the6) + 2*IPx6*cos(the5)^2*cos(the6)*sin(the6) + 2*IPy6*cos(the4)*cos(the6)*sin(the4)*sin(the5) + 2*IPz6*cos(the4)*sin(the4)*sin(the5)*sin(the6) + m6*x6^2*cos(the4)^2*cos(the5)^2*cos(the6)^2 - m6*y6^2*cos(the4)^2*cos(the5)^2*cos(the6)^2 + 2*a2*m4*x4*cos(the3)*cos(the4) + 2*a3*m5*x5*cos(the4)*cos(the5) - 2*a2*m4*y4*cos(the3)*sin(the4) - 2*a2*m5*y5*cos(the5)*sin(the3) - 2*a3*m5*y5*cos(the4)*sin(the5) - 2*a3*m6*y6*cos(the6)*sin(the4) + 2*a2*m5*z5*cos(the3)*sin(the4) - 2*a2*m6*z6*cos(the5)*sin(the3) - 2*a3*m6*z6*cos(the4)*sin(the5) + 2*d4*m6*x6*cos(the6)*sin(the5) - 2*a2*m5*x5*sin(the3)*sin(the5) - 2*a3*m6*x6*sin(the4)*sin(the6) - 4*IPx6*cos(the4)*cos(the5)*cos(the6)^2*sin(the4) - 2*IPz6*cos(the4)^2*cos(the5)*cos(the6)*sin(the5) - 2*d4*m6*y6*sin(the5)*sin(the6) + 2*IPy6*cos(the4)^2*cos(the5)*sin(the5)*sin(the6) - 2*IPx6*cos(the4)^2*cos(the5)^2*cos(the6)*sin(the6) + 2*Ixx6*cos(the4)*cos(the5)*cos(the6)*sin(the4)*sin(the6) - 2*Iyy6*cos(the4)*cos(the5)*cos(the6)*sin(the4)*sin(the6) + 2*a2*m5*x5*cos(the3)*cos(the4)*cos(the5) + 2*a3*m6*x6*cos(the4)*cos(the5)*cos(the6) - 2*a2*m5*y5*cos(the3)*cos(the4)*sin(the5) - 2*a2*m6*y6*cos(the3)*cos(the6)*sin(the4) - 2*a3*m6*y6*cos(the4)*cos(the5)*sin(the6) - 2*a2*m6*z6*cos(the3)*cos(the4)*sin(the5) - 2*a2*m6*x6*cos(the3)*sin(the4)*sin(the6) - 2*a2*m6*x6*cos(the6)*sin(the3)*sin(the5) + 2*m6*x6*y6*cos(the4)*cos(the5)*sin(the4) + 2*m5*x5*z5*cos(the4)*cos(the5)*sin(the4) + 2*m6*x6*z6*cos(the5)*cos(the6)*sin(the5) + 2*a2*m6*y6*sin(the3)*sin(the5)*sin(the6) - 2*m5*y5*z5*cos(the4)*sin(the4)*sin(the5) - 2*m6*y6*z6*cos(the5)*sin(the5)*sin(the6) - 2*m5*x5*y5*cos(the4)^2*cos(the5)*sin(the5) - 2*m6*x6*y6*cos(the4)^2*cos(the6)*sin(the6) + 2*m6*x6*y6*cos(the5)^2*cos(the6)*sin(the6) + 2*a2*m6*x6*cos(the3)*cos(the4)*cos(the5)*cos(the6) - 2*a2*m6*y6*cos(the3)*cos(the4)*cos(the5)*sin(the6) + 2*m6*y6*z6*cos(the4)*cos(the6)*sin(the4)*sin(the5) + 2*m6*x6*z6*cos(the4)*sin(the4)*sin(the5)*sin(the6) - 4*m6*x6*y6*cos(the4)*cos(the5)*cos(the6)^2*sin(the4) - 2*m6*x6*z6*cos(the4)^2*cos(the5)*cos(the6)*sin(the5) + 2*m6*y6*z6*cos(the4)^2*cos(the5)*sin(the5)*sin(the6) - 2*m6*x6*y6*cos(the4)^2*cos(the5)^2*cos(the6)*sin(the6) - 2*m6*x6^2*cos(the4)*cos(the5)*cos(the6)*sin(the4)*sin(the6) + 2*m6*y6^2*cos(the4)*cos(the5)*cos(the6)*sin(the4)*sin(the6),Ixx4 + Iyy5 + Izz3 + Izz6 + a3^2*m4 + a3^2*m5 + a3^2*m6 + d4^2*m4 + d4^2*m5 + d4^2*m6 + m3*x3^2 + m5*x5^2 + m6*x6^2 + m3*y3^2 + m4*y4^2 + m6*y6^2 + m4*z4^2 + m5*z5^2 - Ixx4*cos(the4)^2 + Ixx5*cos(the5)^2 + Ixx6*cos(the4)^2 + Iyy4*cos(the4)^2 - Iyy5*cos(the4)^2 - Iyy5*cos(the5)^2 + Iyy6*cos(the5)^2 + Izz5*cos(the4)^2 - Izz6*cos(the4)^2 - Izz6*cos(the5)^2 - IPx4*sin(2*the4) + IPx5*sin(2*the5) - Ixx5*cos(the4)^2*cos(the5)^2 - Ixx6*cos(the4)^2*cos(the6)^2 + Ixx6*cos(the5)^2*cos(the6)^2 + Iyy5*cos(the4)^2*cos(the5)^2 - Iyy6*cos(the4)^2*cos(the5)^2 + Iyy6*cos(the4)^2*cos(the6)^2 - Iyy6*cos(the5)^2*cos(the6)^2 + Izz6*cos(the4)^2*cos(the5)^2 + 2*d4*m4*z4 + m4*x4^2*cos(the4)^2 - m5*x5^2*cos(the5)^2 - m6*x6^2*cos(the4)^2 - m4*y4^2*cos(the4)^2 + m5*y5^2*cos(the4)^2 + m5*y5^2*cos(the5)^2 - m6*y6^2*cos(the5)^2 - m5*z5^2*cos(the4)^2 + m6*z6^2*cos(the4)^2 + m6*z6^2*cos(the5)^2 - m4*x4*y4*sin(2*the4) + m5*x5*y5*sin(2*the5) + m5*x5^2*cos(the4)^2*cos(the5)^2 + m6*x6^2*cos(the4)^2*cos(the6)^2 - m6*x6^2*cos(the5)^2*cos(the6)^2 - m5*y5^2*cos(the4)^2*cos(the5)^2 + m6*y6^2*cos(the4)^2*cos(the5)^2 - m6*y6^2*cos(the4)^2*cos(the6)^2 + m6*y6^2*cos(the5)^2*cos(the6)^2 - m6*z6^2*cos(the4)^2*cos(the5)^2 + 2*IPx6*cos(the4)*cos(the5)*sin(the4) + 2*IPz5*cos(the4)*cos(the5)*sin(the4) + 2*IPz6*cos(the5)*cos(the6)*sin(the5) - Ixx6*cos(the4)^2*cos(the5)^2*cos(the6)^2 + Iyy6*cos(the4)^2*cos(the5)^2*cos(the6)^2 - 2*IPy5*cos(the4)*sin(the4)*sin(the5) - 2*IPy6*cos(the5)*sin(the5)*sin(the6) + a2*a3*m4*cos(the3) + a2*a3*m5*cos(the3) + a2*a3*m6*cos(the3) - a2*d4*m4*sin(the3) - a2*d4*m5*sin(the3) - a2*d4*m6*sin(the3) + a2*m3*x3*cos(the3) + 2*a3*m4*x4*cos(the4) + 2*d4*m5*y5*cos(the5) + 2*d4*m6*z6*cos(the5) - a2*m3*y3*sin(the3) - 2*a3*m4*y4*sin(the4) - a2*m4*z4*sin(the3) + 2*a3*m5*z5*sin(the4) + 2*d4*m5*x5*sin(the5) - 2*IPx5*cos(the4)^2*cos(the5)*sin(the5) - 2*IPx6*cos(the4)^2*cos(the6)*sin(the6) + 2*IPx6*cos(the5)^2*cos(the6)*sin(the6) + 2*IPy6*cos(the4)*cos(the6)*sin(the4)*sin(the5) + 2*IPz6*cos(the4)*sin(the4)*sin(the5)*sin(the6) + m6*x6^2*cos(the4)^2*cos(the5)^2*cos(the6)^2 - m6*y6^2*cos(the4)^2*cos(the5)^2*cos(the6)^2 + a2*m4*x4*cos(the3)*cos(the4) + 2*a3*m5*x5*cos(the4)*cos(the5) - a2*m4*y4*cos(the3)*sin(the4) - a2*m5*y5*cos(the5)*sin(the3) - 2*a3*m5*y5*cos(the4)*sin(the5) - 2*a3*m6*y6*cos(the6)*sin(the4) + a2*m5*z5*cos(the3)*sin(the4) - a2*m6*z6*cos(the5)*sin(the3) - 2*a3*m6*z6*cos(the4)*sin(the5) + 2*d4*m6*x6*cos(the6)*sin(the5) - a2*m5*x5*sin(the3)*sin(the5) - 2*a3*m6*x6*sin(the4)*sin(the6) - 4*IPx6*cos(the4)*cos(the5)*cos(the6)^2*sin(the4) - 2*IPz6*cos(the4)^2*cos(the5)*cos(the6)*sin(the5) - 2*d4*m6*y6*sin(the5)*sin(the6) + 2*IPy6*cos(the4)^2*cos(the5)*sin(the5)*sin(the6) - 2*IPx6*cos(the4)^2*cos(the5)^2*cos(the6)*sin(the6) + 2*Ixx6*cos(the4)*cos(the5)*cos(the6)*sin(the4)*sin(the6) - 2*Iyy6*cos(the4)*cos(the5)*cos(the6)*sin(the4)*sin(the6) + a2*m5*x5*cos(the3)*cos(the4)*cos(the5) + 2*a3*m6*x6*cos(the4)*cos(the5)*cos(the6) - a2*m5*y5*cos(the3)*cos(the4)*sin(the5) - a2*m6*y6*cos(the3)*cos(the6)*sin(the4) - 2*a3*m6*y6*cos(the4)*cos(the5)*sin(the6) - a2*m6*z6*cos(the3)*cos(the4)*sin(the5) - a2*m6*x6*cos(the3)*sin(the4)*sin(the6) - a2*m6*x6*cos(the6)*sin(the3)*sin(the5) + 2*m6*x6*y6*cos(the4)*cos(the5)*sin(the4) + 2*m5*x5*z5*cos(the4)*cos(the5)*sin(the4) + 2*m6*x6*z6*cos(the5)*cos(the6)*sin(the5) + a2*m6*y6*sin(the3)*sin(the5)*sin(the6) - 2*m5*y5*z5*cos(the4)*sin(the4)*sin(the5) - 2*m6*y6*z6*cos(the5)*sin(the5)*sin(the6) - 2*m5*x5*y5*cos(the4)^2*cos(the5)*sin(the5) - 2*m6*x6*y6*cos(the4)^2*cos(the6)*sin(the6) + 2*m6*x6*y6*cos(the5)^2*cos(the6)*sin(the6) + a2*m6*x6*cos(the3)*cos(the4)*cos(the5)*cos(the6) - a2*m6*y6*cos(the3)*cos(the4)*cos(the5)*sin(the6) + 2*m6*y6*z6*cos(the4)*cos(the6)*sin(the4)*sin(the5) + 2*m6*x6*z6*cos(the4)*sin(the4)*sin(the5)*sin(the6) - 4*m6*x6*y6*cos(the4)*cos(the5)*cos(the6)^2*sin(the4) - 2*m6*x6*z6*cos(the4)^2*cos(the5)*cos(the6)*sin(the5) + 2*m6*y6*z6*cos(the4)^2*cos(the5)*sin(the5)*sin(the6) - 2*m6*x6*y6*cos(the4)^2*cos(the5)^2*cos(the6)*sin(the6) - 2*m6*x6^2*cos(the4)*cos(the5)*cos(the6)*sin(the4)*sin(the6) + 2*m6*y6^2*cos(the4)*cos(the5)*cos(the6)*sin(the4)*sin(the6),IPy4*cos(the4) - IPx5*sin(the4) + IPz4*sin(the4) - IPy5*cos(the4)*cos(the5) - IPx6*cos(the4)*sin(the5) - IPz5*cos(the4)*sin(the5) - IPz6*cos(the6)*sin(the4) + IPy6*sin(the4)*sin(the6) + 2*IPx5*cos(the5)^2*sin(the4) + IPy6*cos(the4)*cos(the5)*cos(the6) + IPz6*cos(the4)*cos(the5)*sin(the6) - Ixx5*cos(the5)*sin(the4)*sin(the5) + Iyy5*cos(the5)*sin(the4)*sin(the5) - Iyy6*cos(the5)*sin(the4)*sin(the5) + Izz6*cos(the5)*sin(the4)*sin(the5) + d4*m4*y4*cos(the4) - d4*m5*z5*cos(the4) + d4*m4*x4*sin(the4) + m4*y4*z4*cos(the4) + 2*IPx6*cos(the4)*cos(the6)^2*sin(the5) + 2*IPz6*cos(the5)^2*cos(the6)*sin(the4) - m5*x5*y5*sin(the4) + m4*x4*z4*sin(the4) - 2*IPy6*cos(the5)^2*sin(the4)*sin(the6) - Ixx6*cos(the4)*cos(the6)*sin(the5)*sin(the6) + Iyy6*cos(the4)*cos(the6)*sin(the5)*sin(the6) + m5*x5^2*cos(the5)*sin(the4)*sin(the5) - m5*y5^2*cos(the5)*sin(the4)*sin(the5) + m6*y6^2*cos(the5)*sin(the4)*sin(the5) - m6*z6^2*cos(the5)*sin(the4)*sin(the5) + d4*m6*y6*cos(the4)*cos(the6) - a2*m4*y4*cos(the4)*sin(the3) + a2*m5*z5*cos(the4)*sin(the3) + d4*m5*x5*cos(the5)*sin(the4) + d4*m6*x6*cos(the4)*sin(the6) - m5*y5*z5*cos(the4)*cos(the5) - a2*m4*x4*sin(the3)*sin(the4) - d4*m5*y5*sin(the4)*sin(the5) - d4*m6*z6*sin(the4)*sin(the5) - m6*x6*y6*cos(the4)*sin(the5) - m5*x5*z5*cos(the4)*sin(the5) - m6*x6*z6*cos(the6)*sin(the4) - Ixx6*cos(the5)*cos(the6)^2*sin(the4)*sin(the5) + Iyy6*cos(the5)*cos(the6)^2*sin(the4)*sin(the5) + m6*y6*z6*sin(the4)*sin(the6) + 2*m5*x5*y5*cos(the5)^2*sin(the4) - 2*IPx6*cos(the5)*cos(the6)*sin(the4)*sin(the5)*sin(the6) + m6*x6^2*cos(the4)*cos(the6)*sin(the5)*sin(the6) - m6*y6^2*cos(the4)*cos(the6)*sin(the5)*sin(the6) - a2*m6*y6*cos(the4)*cos(the6)*sin(the3) + d4*m6*x6*cos(the5)*cos(the6)*sin(the4) + m6*y6*z6*cos(the4)*cos(the5)*cos(the6) - a2*m5*x5*cos(the5)*sin(the3)*sin(the4) - a2*m6*x6*cos(the4)*sin(the3)*sin(the6) - d4*m6*y6*cos(the5)*sin(the4)*sin(the6) + m6*x6*z6*cos(the4)*cos(the5)*sin(the6) + a2*m5*y5*sin(the3)*sin(the4)*sin(the5) + a2*m6*z6*sin(the3)*sin(the4)*sin(the5) + m6*x6^2*cos(the5)*cos(the6)^2*sin(the4)*sin(the5) - m6*y6^2*cos(the5)*cos(the6)^2*sin(the4)*sin(the5) + 2*m6*x6*y6*cos(the4)*cos(the6)^2*sin(the5) + 2*m6*x6*z6*cos(the5)^2*cos(the6)*sin(the4) - 2*m6*y6*z6*cos(the5)^2*sin(the4)*sin(the6) - a2*m6*x6*cos(the5)*cos(the6)*sin(the3)*sin(the4) + a2*m6*y6*cos(the5)*sin(the3)*sin(the4)*sin(the6) - 2*m6*x6*y6*cos(the5)*cos(the6)*sin(the4)*sin(the5)*sin(the6),Ixx6*cos(the4) + Izz5*cos(the4) + IPx6*cos(the5)*sin(the4) + IPz5*cos(the5)*sin(the4) - IPy5*sin(the4)*sin(the5) + m5*x5^2*cos(the4) + m5*y5^2*cos(the4) + m6*y6^2*cos(the4) + m6*z6^2*cos(the4) - Ixx6*cos(the4)*cos(the6)^2 + Iyy6*cos(the4)*cos(the6)^2 - 2*IPx6*cos(the4)*cos(the6)*sin(the6) + IPy6*cos(the6)*sin(the4)*sin(the5) + IPz6*sin(the4)*sin(the5)*sin(the6) + a3*m5*x5*cos(the5) - a3*m5*y5*sin(the5) - a3*m6*z6*sin(the5) - 2*IPx6*cos(the5)*cos(the6)^2*sin(the4) + m6*x6^2*cos(the4)*cos(the6)^2 - m6*y6^2*cos(the4)*cos(the6)^2 + Ixx6*cos(the5)*cos(the6)*sin(the4)*sin(the6) - Iyy6*cos(the5)*cos(the6)*sin(the4)*sin(the6) + a2*m5*x5*cos(the3)*cos(the5) + a3*m6*x6*cos(the5)*cos(the6) + d4*m5*y5*cos(the4)*cos(the5) + d4*m6*z6*cos(the4)*cos(the5) - a2*m5*y5*cos(the3)*sin(the5) - a3*m6*y6*cos(the5)*sin(the6) - a2*m6*z6*cos(the3)*sin(the5) + d4*m5*x5*cos(the4)*sin(the5) + m6*x6*y6*cos(the5)*sin(the4) + m5*x5*z5*cos(the5)*sin(the4) - m5*y5*z5*sin(the4)*sin(the5) - m6*x6^2*cos(the5)*cos(the6)*sin(the4)*sin(the6) + m6*y6^2*cos(the5)*cos(the6)*sin(the4)*sin(the6) + a2*m6*x6*cos(the3)*cos(the5)*cos(the6) - a2*m5*y5*cos(the4)*cos(the5)*sin(the3) - a2*m6*y6*cos(the3)*cos(the5)*sin(the6) - a2*m6*z6*cos(the4)*cos(the5)*sin(the3) + d4*m6*x6*cos(the4)*cos(the6)*sin(the5) - a2*m5*x5*cos(the4)*sin(the3)*sin(the5) - d4*m6*y6*cos(the4)*sin(the5)*sin(the6) - 2*m6*x6*y6*cos(the4)*cos(the6)*sin(the6) + m6*y6*z6*cos(the6)*sin(the4)*sin(the5) + m6*x6*z6*sin(the4)*sin(the5)*sin(the6) - 2*m6*x6*y6*cos(the5)*cos(the6)^2*sin(the4) - a2*m6*x6*cos(the4)*cos(the6)*sin(the3)*sin(the5) + a2*m6*y6*cos(the4)*sin(the3)*sin(the5)*sin(the6),IPy6*cos(the4)*cos(the6) + IPz6*cos(the4)*sin(the6) + Izz6*sin(the4)*sin(the5) + IPz6*cos(the5)*cos(the6)*sin(the4) - IPy6*cos(the5)*sin(the4)*sin(the6) + m6*x6^2*sin(the4)*sin(the5) + m6*y6^2*sin(the4)*sin(the5) - a3*m6*y6*cos(the6)*sin(the5) + d4*m6*x6*cos(the6)*sin(the4) + m6*y6*z6*cos(the4)*cos(the6) - a3*m6*x6*sin(the5)*sin(the6) - d4*m6*y6*sin(the4)*sin(the6) + m6*x6*z6*cos(the4)*sin(the6) + d4*m6*y6*cos(the4)*cos(the5)*cos(the6) - a2*m6*y6*cos(the3)*cos(the6)*sin(the5) + d4*m6*x6*cos(the4)*cos(the5)*sin(the6) - a2*m6*x6*cos(the6)*sin(the3)*sin(the4) - a2*m6*x6*cos(the3)*sin(the5)*sin(the6) + m6*x6*z6*cos(the5)*cos(the6)*sin(the4) + a2*m6*y6*sin(the3)*sin(the4)*sin(the6) - m6*y6*z6*cos(the5)*sin(the4)*sin(the6) - a2*m6*y6*cos(the4)*cos(the5)*cos(the6)*sin(the3) - a2*m6*x6*cos(the4)*cos(the5)*sin(the3)*sin(the6);
